simulink library "mbd_s32k1xx_ec_toolbox"  (Simulink 9.0)
settings: Solver=FixedStepDiscrete  StartTime=0.0  StopTime=10.0  FixedStep=0.1  RelTol=1e-3  EnableMultiTasking=on
InitFcn:
  | mbd_s32k_consistency_checks(bdroot(gcs));
(part 6 of 8)

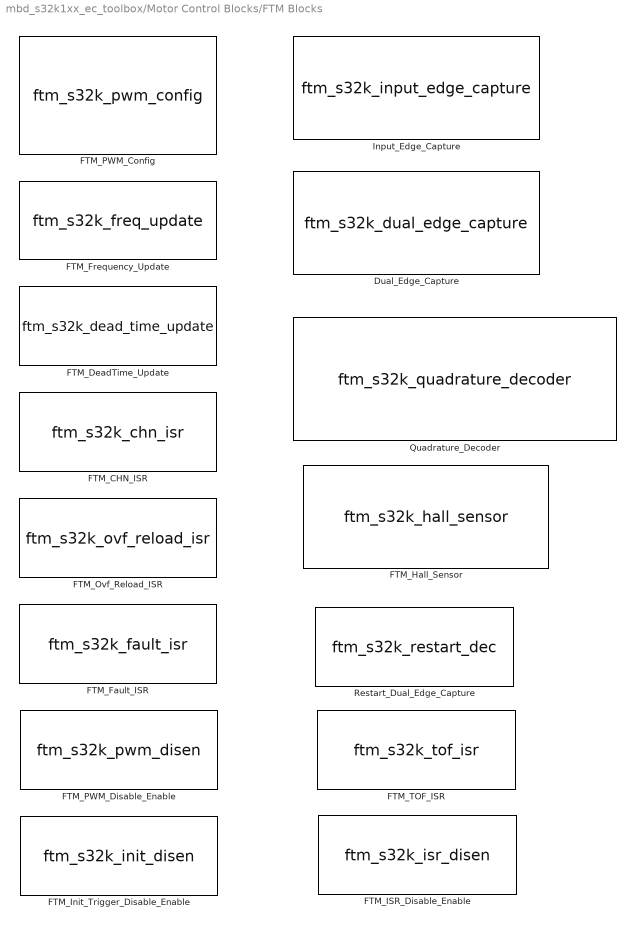
== system mbd_s32k1xx_ec_toolbox/Motor Control Blocks/FTM Blocks ==
  Dual_Edge_Capture : S-Function  FunctionName=ftm_s32k_dual_edge_capture  Parameters=funcParam  SFunctionDeploymentMode=off  EnableBusSupport=off  mask(FTM_s32k_dual_edge_capture_block){ftmModule=0, channel=0-1, c_mode=One-Shot, mesur=positive pulse (rising - falling), prescaler=1, filter_en=off, filter_value=0, isrlevel=15, pinFtmCh=PTD15: [FTM0_CH0 | FTM Channel]}
      mask prompts: ftmModule "Module"; channel "Channel pair"; c_mode "Capture mode"; mesur "Measurement"; prescaler "Prescale Factor"; filter_en "Filter enable"; filter_value "Input Filter value"; isrlevel "ISR priority"; pinFtmCh "FTM input pin"
      mask help: Dual Edge Capture block for signal pulse or period measurement on the even channel input.
      mask init:
      | mbd_s32k_ftm_display_modules(gcb);
      | mbd_s32k_ftm_edge_cbk(gcb, 'dual');
      | mbd_s32k_isr_priority_cbk(gcb, 'isrlevel');
      | 
      | [labels, maskStr] = mbd_s32k_ftm_dual_edge_init(gcb);
      | set_param(gcb, 'MaskDisplay', labels);
      | 
      | funcParam = [];
      settings: NameChangeFcn=mbd_s32k_name_check(gcb);
      mask Help: web(fullfile(mbd_s32k_block_help, 'ftm', 'dual_edge_capture_input.html'));
      mask TypeOptions ftmModule: 0 | 1 | 2 | 3 | 4 | 5 | 6 | 7
      mask Callback ftmModule:
      | mbd_s32k_ftm_display_modules(gcb);
      | mbd_s32k_ftm_edge_cbk(gcb, 'dual');
      mask TypeOptions channel: 0-1 | 2-3 | 4-5 | 6-7
      mask Callback channel: mbd_s32k_ftm_edge_cbk(gcb, 'dual');
      mask TypeOptions c_mode: One-Shot | Continuous
      mask TypeOptions mesur: positive pulse (rising - falling) | negative pulse (falling - rising) | period (rising - rising) | period (falling - falling)
      mask TypeOptions prescaler: 1 | 2 | 4 | 8 | 16 | 32 | 64 | 128
      mask Callback filter_en:
      | vis = get_param(gcb, 'MaskVisibilities');
      | 
      | %show/hide Filter value
      | idx = mbd_s32k_get_param_index(gcb, 'filter_value');
      | if strcmp(get_param(gcb,'filter_en'),'on')==1,
      |      vis{idx} = 'on';
      | elseif strcmp(get_param(gcb,'filter_en'),'off')==1,
      |     vis{idx} = 'off';
      | end
      | 
      | set_param(gcb,'MaskVisibilities',vis);
      | clear vis;
      mask TypeOptions isrlevel: 0 | 1 | 2 | 3 | 4 | 5 | 6 | 7 | 8 | 9 | 10 | 11 | 12 | 13 | 14 | 15
      mask TypeOptions pinFtmCh: PTD15: [FTM0_CH0 | FTM Channel] | PTB13: [FTM0_CH1 | FTM Channel] | PTC1: [FTM0_CH1 | FTM Channel] | PTD16: [FTM0_CH1 | FTM Channel] | PTC2: [FTM0_CH2 | FTM Channel] | PTD0: [FTM0_CH2 | FTM Channel] | PTC3: [FTM0_CH3 | FTM Channel] | PTD1: [FTM0_CH3 | FTM Channel] | PTB4: [FTM0_CH4 | FTM Channel] | PTB5: [FTM0_CH5 | FTM Channel] | PTE8: [FTM0_CH6 | FTM Channel] | PTE9: [FTM0_CH7 | FTM Channel] | PTB2: [FTM1_CH0 | FTM Channel] | PTC4: [FTM1_CH0 | FTM Channel] | PTA1: [FTM1_CH1 | FTM Channel] | PTB3: [FTM1_CH1 | FTM Channel] | PTC14: [FTM1_CH2 | FTM Channel] | PTC15: [FTM1_CH3 | FTM Channel] | PTA10: [FTM1_CH4 | FTM Channel] | PTA11: [FTM1_CH5 | FTM Channel] | PTA12: [FTM1_CH6 | FTM Channel] | PTA13: [FTM1_CH7 | FTM Channel] | PTC1: [FTM1_CH7 | FTM Channel] | PTD15: [FTM0_CH0 | FTM Channel] | PTB13: [FTM0_CH1 | FTM Channel] | PTC1: [FTM0_CH1 | FTM Channel] | PTD16: [FTM0_CH1 | FTM Channel] | PTC2: [FTM0_CH2 | FTM Channel] | PTD0: [FTM0_CH2 | FTM Channel] | PTC3: [FTM0_CH3 | FTM Channel] | PTD1: [FTM0_CH3 | FTM Channel] | PTB4: [FTM0_CH4 | FTM Channel] | PTB5: [FTM0_CH5 | FTM Channel] | PTE8: [FTM0_CH6 | FTM Channel] | PTE9: [FTM0_CH7 | FTM Channel] | PTB2: [FTM1_CH0 | FTM Channel] | PTC4: [FTM1_CH0 | FTM Channel] | PTA1: [FTM1_CH1 | FTM Channel] | PTB3: [FTM1_CH1 | FTM Channel] | PTC14: [FTM1_CH2 | FTM Channel] | PTC15: [FTM1_CH3 | FTM Channel] | PTA10: [FTM1_CH4 | FTM Channel] | PTA11: [FTM1_CH5 | FTM Channel] | PTA12: [FTM1_CH6 | FTM Channel] | PTA13: [FTM1_CH7 | FTM Channel] | PTC1: [FTM1_CH7 | FTM Channel] | PTD15: [FTM0_CH0 | FTM Channel] | PTB13: [FTM0_CH1 | FTM Channel] | PTC1: [FTM0_CH1 | FTM Channel] | PTD16: [FTM0_CH1 | FTM Channel] | PTC2: [FTM0_CH2 | FTM Channel] | PTD0: [FTM0_CH2 | FTM Channel] | PTC3: [FTM0_CH3 | FTM Channel] | PTD1: [FTM0_CH3 | FTM Channel] | PTB4: [FTM0_CH4 | FTM Channel] | PTB5: [FTM0_CH5 | FTM Channel] | PTE8: [FTM0_CH6 | FTM Channel] | PTE9: [FTM0_CH7 | FTM Channel] | PTB2: [FTM1_CH0 | FTM Channel] | PTC4: [FTM1_CH0 | FTM Channel] | PTA1: [FTM1_CH1 | FTM Channel] | PTB3: [FTM1_CH1 | FTM Channel] | PTC14: [FTM1_CH2 | FTM Channel] | PTC15: [FTM1_CH3 | FTM Channel] | PTA10: [FTM1_CH4 | FTM Channel] | PTA11: [FTM1_CH5 | FTM Channel] | PTA12: [FTM1_CH6 | FTM Channel] | PTA13: [FTM1_CH7 | FTM Channel] | PTC1: [FTM1_CH7 | FTM Channel] | PTC5: [FTM2_CH0 | FTM Channel] | PTD0: [FTM2_CH0 | FTM Channel] | PTD10: [FTM2_CH0 | FTM Channel] | PTA0: [FTM2_CH1 | FTM Channel] | PTD1: [FTM2_CH1 | FTM Channel] | PTD11: [FTM2_CH1 | FTM Channel] | PTD12: [FTM2_CH2 | FTM Channel] | PTE4: [FTM2_CH2 | FTM Channel] | PTD5: [FTM2_CH3 | FTM Channel] | PTE5: [FTM2_CH3 | FTM Channel] | PTD13: [FTM2_CH4 | FTM Channel] | PTE10: [FTM2_CH4 | FTM Channel] | PTD14: [FTM2_CH5 | FTM Channel] | PTE11: [FTM2_CH5 | FTM Channel] | PTC12: [FTM2_CH6 | FTM Channel] | PTE15: [FTM2_CH6 | FTM Channel] | PTC13: [FTM2_CH7 | FTM Channel] | PTE16: [FTM2_CH7 | FTM Channel] | PTA2: [FTM3_CH0 | FTM Channel] | PTB8: [FTM3_CH0 | FTM Channel] | PTA3: [FTM3_CH1 | FTM Channel] | PTB9: [FTM3_CH1 | FTM Channel] | PTB10: [FTM3_CH2 | FTM Channel] | PTC6: [FTM3_CH2 | FTM Channel] | PTB11: [FTM3_CH3 | FTM Channel] | PTC7: [FTM3_CH3 | FTM Channel] | PTC10: [FTM3_CH4 | FTM Channel] | PTD2: [FTM3_CH4 | FTM Channel] | PTC11: [FTM3_CH5 | FTM Channel] | PTD3: [FTM3_CH5 | FTM Channel] | PTC12: [FTM3_CH6 | FTM Channel] | PTE2: [FTM3_CH6 | FTM Channel] | PTC13: [FTM3_CH7 | FTM Channel] | PTE6: [FTM3_CH7 | FTM Channel] | PTD15: [FTM0_CH0 | FTM Channel] | PTB13: [FTM0_CH1 | FTM Channel] | PTC1: [FTM0_CH1 | FTM Channel] | PTD16: [FTM0_CH1 | FTM Channel] | PTC2: [FTM0_CH2 | FTM Channel] | PTD0: [FTM0_CH2 | FTM Channel] | PTC3: [FTM0_CH3 | FTM Channel] | PTD1: [FTM0_CH3 | FTM Channel] | PTB4: [FTM0_CH4 | FTM Channel] | PTB5: [FTM0_CH5 | FTM Channel] | PTE8: [FTM0_CH6 | FTM Channel] | PTE9: [FTM0_CH7 | FTM Channel] | PTB2: [FTM1_CH0 | FTM Channel] | PTC4: [FTM1_CH0 | FTM Channel] | PTA1: [FTM1_CH1 | FTM Channel] | PTB3: [FTM1_CH1 | FTM Channel] | PTC14: [FTM1_CH2 | FTM Channel] | PTC15: [FTM1_CH3 | FTM Channel] | PTA10: [FTM1_CH4 | FTM Channel] | PTA11: [FTM1_CH5 | FTM Channel] | PTA12: [FTM1_CH6 | FTM Channel] | PTA13: [FTM1_CH7 | FTM Channel] | PTC1: [FTM1_CH7 | FTM Channel] | PTC5: [FTM2_CH0 | FTM Channel] | PTD0: [FTM2_CH0 | FTM Channel] | PTD10: [FTM2_CH0 | FTM Channel] | PTA0: [FTM2_CH1 | FTM Channel] | PTD1: [FTM2_CH1 | FTM Channel] | PTD11: [FTM2_CH1 | FTM Channel] | PTD12: [FTM2_CH2 | FTM Channel] | PTE4: [FTM2_CH2 | FTM Channel] | PTD5: [FTM2_CH3 | FTM Channel] | PTE5: [FTM2_CH3 | FTM Channel] | PTD13: [FTM2_CH4 | FTM Channel] | PTE10: [FTM2_CH4 | FTM Channel] | PTD14: [FTM2_CH5 | FTM Channel] | PTE11: [FTM2_CH5 | FTM Channel] | PTC12: [FTM2_CH6 | FTM Channel] | PTE15: [FTM2_CH6 | FTM Channel] | PTC13: [FTM2_CH7 | FTM Channel] | PTE16: [FTM2_CH7 | FTM Channel] | PTA2: [FTM3_CH0 | FTM Channel] | PTB8: [FTM3_CH0 | FTM Channel] | PTA3: [FTM3_CH1 | FTM Channel] | PTB9: [FTM3_CH1 | FTM Channel] | PTB10: [FTM3_CH2 | FTM Channel] | PTC6: [FTM3_CH2 | FTM Channel] | PTB11: [FTM3_CH3 | FTM Channel] | PTC7: [FTM3_CH3 | FTM Channel] | PTC10: [FTM3_CH4 | FTM Channel] | PTD2: [FTM3_CH4 | FTM Channel] | PTC11: [FTM3_CH5 | FTM Channel] | PTD3: [FTM3_CH5 | FTM Channel] | PTC12: [FTM3_CH6 | FTM Channel] | PTE2: [FTM3_CH6 | FTM Channel] | PTC13: [FTM3_CH7 | FTM Channel] | PTE6: [FTM3_CH7 | FTM Channel] | PTD15: [FTM0_CH0 | FTM Channel] | PTB13: [FTM0_CH1 | FTM Channel] | PTC1: [FTM0_CH1 | FTM Channel] | PTD16: [FTM0_CH1 | FTM Channel] | PTC2: [FTM0_CH2 | FTM Channel] | PTD0: [FTM0_CH2 | FTM Channel] | PTC3: [FTM0_CH3 | FTM Channel] | PTD1: [FTM0_CH3 | FTM Channel] | PTB4: [FTM0_CH4 | FTM Channel] | PTB5: [FTM0_CH5 | FTM Channel] | PTE8: [FTM0_CH6 | FTM Channel] | PTE9: [FTM0_CH7 | FTM Channel] | PTB2: [FTM1_CH0 | FTM Channel] | PTC4: [FTM1_CH0 | FTM Channel] | PTA1: [FTM1_CH1 | FTM Channel] | PTB3: [FTM1_CH1 | FTM Channel] | PTC14: [FTM1_CH2 | FTM Channel] | PTC15: [FTM1_CH3 | FTM Channel] | PTA10: [FTM1_CH4 | FTM Channel] | PTA11: [FTM1_CH5 | FTM Channel] | PTA12: [FTM1_CH6 | FTM Channel] | PTA13: [FTM1_CH7 | FTM Channel] | PTC1: [FTM1_CH7 | FTM Channel] | PTC5: [FTM2_CH0 | FTM Channel] | PTD0: [FTM2_CH0 | FTM Channel] | PTD10: [FTM2_CH0 | FTM Channel] | PTA0: [FTM2_CH1 | FTM Channel] | PTD1: [FTM2_CH1 | FTM Channel] | PTD11: [FTM2_CH1 | FTM Channel] | PTD12: [FTM2_CH2 | FTM Channel] | PTE4: [FTM2_CH2 | FTM Channel] | PTD5: [FTM2_CH3 | FTM Channel] | PTE5: [FTM2_CH3 | FTM Channel] | PTD13: [FTM2_CH4 | FTM Channel] | PTE10: [FTM2_CH4 | FTM Channel] | PTD14: [FTM2_CH5 | FTM Channel] | PTE11: [FTM2_CH5 | FTM Channel] | PTC12: [FTM2_CH6 | FTM Channel] | PTE15: [FTM2_CH6 | FTM Channel] | PTC13: [FTM2_CH7 | FTM Channel] | PTE16: [FTM2_CH7 | FTM Channel] | PTA2: [FTM3_CH0 | FTM Channel] | PTB8: [FTM3_CH0 | FTM Channel] | PTA3: [FTM3_CH1 | FTM Channel] | PTB9: [FTM3_CH1 | FTM Channel] | PTB10: [FTM3_CH2 | FTM Channel] | PTC6: [FTM3_CH2 | FTM Channel] | PTB11: [FTM3_CH3 | FTM Channel] | PTC7: [FTM3_CH3 | FTM Channel] | PTC10: [FTM3_CH4 | FTM Channel] | PTD2: [FTM3_CH4 | FTM Channel] | PTC11: [FTM3_CH5 | FTM Channel] | PTD3: [FTM3_CH5 | FTM Channel] | PTC12: [FTM3_CH6 | FTM Channel] | PTE2: [FTM3_CH6 | FTM Channel] | PTC13: [FTM3_CH7 | FTM Channel] | PTE6: [FTM3_CH7 | FTM Channel] | PTE20: [FTM4_CH0 | FTM Channel] | PTE21: [FTM4_CH1 | FTM Channel] | PTC11: [FTM4_CH2 | FTM Channel] | PTE22: [FTM4_CH2 | FTM Channel] | PTE23: [FTM4_CH3 | FTM Channel] | PTC27: [FTM4_CH4 | FTM Channel] | PTE24: [FTM4_CH4 | FTM Channel] | PTB1: [FTM4_CH5 | FTM Channel] | PTE13: [FTM4_CH5 | FTM Channel] | PTE25: [FTM4_CH5 | FTM Channel] | PTB0: [FTM4_CH6 | FTM Channel] | PTC28: [FTM4_CH7 | FTM Channel] | PTA25: [FTM5_CH0 | FTM Channel] | PTC9: [FTM5_CH0 | FTM Channel] | PTA26: [FTM5_CH1 | FTM Channel] | PTC8: [FTM5_CH1 | FTM Channel] | PTA27: [FTM5_CH2 | FTM Channel] | PTC29: [FTM5_CH2 | FTM Channel] | PTA7: [FTM5_CH3 | FTM Channel] | PTA28: [FTM5_CH3 | FTM Channel] | PTA29: [FTM5_CH4 | FTM Channel] | PTC30: [FTM5_CH4 | FTM Channel] | PTA6: [FTM5_CH5 | FTM Channel] | PTA30: [FTM5_CH5 | FTM Channel] | PTA31: [FTM5_CH6 | FTM Channel] | PTC31: [FTM5_CH6 | FTM Channel] | PTB18: [FTM5_CH7 | FTM Channel] | PTD18: [FTM5_CH7 | FTM Channel] | PTD15: [FTM0_CH0 | FTM Channel] | PTB13: [FTM0_CH1 | FTM Channel] | PTC1: [FTM0_CH1 | FTM Channel] | PTD16: [FTM0_CH1 | FTM Channel] | PTC2: [FTM0_CH2 | FTM Channel] | PTD0: [FTM0_CH2 | FTM Channel] | PTC3: [FTM0_CH3 | FTM Channel] | PTD1: [FTM0_CH3 | FTM Channel] | PTB4: [FTM0_CH4 | FTM Channel] | PTB5: [FTM0_CH5 | FTM Channel] | PTE8: [FTM0_CH6 | FTM Channel] | PTE9: [FTM0_CH7 | FTM Channel] | PTB2: [FTM1_CH0 | FTM Channel] | PTC4: [FTM1_CH0 | FTM Channel] | PTA1: [FTM1_CH1 | FTM Channel] | PTB3: [FTM1_CH1 | FTM Channel] | PTC14: [FTM1_CH2 | FTM Channel] | PTC15: [FTM1_CH3 | FTM Channel] | PTA10: [FTM1_CH4 | FTM Channel] | PTA11: [FTM1_CH5 | FTM Channel] | PTA12: [FTM1_CH6 | FTM Channel] | PTA13: [FTM1_CH7 | FTM Channel] | PTC1: [FTM1_CH7 | FTM Channel] | PTC5: [FTM2_CH0 | FTM Channel] | PTD0: [FTM2_CH0 | FTM Channel] | PTD10: [FTM2_CH0 | FTM Channel] | PTA0: [FTM2_CH1 | FTM Channel] | PTD1: [FTM2_CH1 | FTM Channel] | PTD11: [FTM2_CH1 | FTM Channel] | PTD12: [FTM2_CH2 | FTM Channel] | PTE4: [FTM2_CH2 | FTM Channel] | PTD5: [FTM2_CH3 | FTM Channel] | PTE5: [FTM2_CH3 | FTM Channel] | PTD13: [FTM2_CH4 | FTM Channel] | PTE10: [FTM2_CH4 | FTM Channel] | PTD14: [FTM2_CH5 | FTM Channel] | PTE11: [FTM2_CH5 | FTM Channel] | PTC12: [FTM2_CH6 | FTM Channel] | PTE15: [FTM2_CH6 | FTM Channel] | PTC13: [FTM2_CH7 | FTM Channel] | PTE16: [FTM2_CH7 | FTM Channel] | PTA2: [FTM3_CH0 | FTM Channel] | PTB8: [FTM3_CH0 | FTM Channel] | PTA3: [FTM3_CH1 | FTM Channel] | PTB9: [FTM3_CH1 | FTM Channel] | PTB10: [FTM3_CH2 | FTM Channel] | PTC6: [FTM3_CH2 | FTM Channel] | PTB11: [FTM3_CH3 | FTM Channel] | PTC7: [FTM3_CH3 | FTM Channel] | PTC10: [FTM3_CH4 | FTM Channel] | PTD2: [FTM3_CH4 | FTM Channel] | PTC11: [FTM3_CH5 | FTM Channel] | PTD3: [FTM3_CH5 | FTM Channel] | PTC12: [FTM3_CH6 | FTM Channel] | PTE2: [FTM3_CH6 | FTM Channel] | PTC13: [FTM3_CH7 | FTM Channel] | PTE6: [FTM3_CH7 | FTM Channel] | PTE20: [FTM4_CH0 | FTM Channel] | PTE21: [FTM4_CH1 | FTM Channel] | PTC11: [FTM4_CH2 | FTM Channel] | PTE22: [FTM4_CH2 | FTM Channel] | PTE23: [FTM4_CH3 | FTM Channel] | PTC27: [FTM4_CH4 | FTM Channel] | PTE24: [FTM4_CH4 | FTM Channel] | PTB1: [FTM4_CH5 | FTM Channel] | PTE13: [FTM4_CH5 | FTM Channel] | PTE25: [FTM4_CH5 | FTM Channel] | PTB0: [FTM4_CH6 | FTM Channel] | PTC28: [FTM4_CH7 | FTM Channel] | PTA25: [FTM5_CH0 | FTM Channel] | PTC9: [FTM5_CH0 | FTM Channel] | PTA26: [FTM5_CH1 | FTM Channel] | PTC8: [FTM5_CH1 | FTM Channel] | PTA27: [FTM5_CH2 | FTM Channel] | PTC29: [FTM5_CH2 | FTM Channel] | PTA7: [FTM5_CH3 | FTM Channel] | PTA28: [FTM5_CH3 | FTM Channel] | PTA29: [FTM5_CH4 | FTM Channel] | PTC30: [FTM5_CH4 | FTM Channel] | PTA6: [FTM5_CH5 | FTM Channel] | PTA30: [FTM5_CH5 | FTM Channel] | PTA31: [FTM5_CH6 | FTM Channel] | PTC31: [FTM5_CH6 | FTM Channel] | PTB18: [FTM5_CH7 | FTM Channel] | PTD18: [FTM5_CH7 | FTM Channel] | PTA18: [FTM6_CH0 | FTM Channel] | PTB20: [FTM6_CH0 | FTM Channel] | PTD19: [FTM6_CH0 | FTM Channel] | PTB21: [FTM6_CH1 | FTM Channel] | PTD20: [FTM6_CH1 | FTM Channel] | PTB22: [FTM6_CH2 | FTM Channel] | PTD21: [FTM6_CH2 | FTM Channel] | PTB23: [FTM6_CH3 | FTM Channel] | PTD22: [FTM6_CH3 | FTM Channel] | PTB24: [FTM6_CH4 | FTM Channel] | PTD23: [FTM6_CH4 | FTM Channel] | PTB25: [FTM6_CH5 | FTM Channel] | PTD24: [FTM6_CH5 | FTM Channel] | PTB26: [FTM6_CH6 | FTM Channel] | PTD25: [FTM6_CH6 | FTM Channel] | PTB27: [FTM6_CH7 | FTM Channel] | PTD26: [FTM6_CH7 | FTM Channel] | PTB28: [FTM7_CH0 | FTM Channel] | PTD27: [FTM7_CH0 | FTM Channel] | PTB29: [FTM7_CH1 | FTM Channel] | PTD28: [FTM7_CH1 | FTM Channel] | PTB30: [FTM7_CH2 | FTM Channel] | PTD29: [FTM7_CH2 | FTM Channel] | PTB31: [FTM7_CH3 | FTM Channel] | PTD30: [FTM7_CH3 | FTM Channel] | PTC18: [FTM7_CH4 | FTM Channel] | PTD31: [FTM7_CH4 | FTM Channel] | PTC19: [FTM7_CH5 | FTM Channel] | PTE17: [FTM7_CH5 | FTM Channel] | PTC20: [FTM7_CH6 | FTM Channel] | PTE18: [FTM7_CH6 | FTM Channel] | PTC21: [FTM7_CH7 | FTM Channel] | PTE19: [FTM7_CH7 | FTM Channel]
      mask Display:
      | image('nxp_logo.png', 'top-right');
      | port_label('output',1,'Trigger');
      | port_label('output',2,'Measured Time');
      | disp(maskStr);
  FTM_CHN_ISR : S-Function  Priority=10  FunctionName=ftm_s32k_chn_isr  Parameters=ftmModule,channel,isrlevel  SFunctionDeploymentMode=off  EnableBusSupport=off  mask(FTM_s32k_chn_isr_block){ftmModule=0, channel=0, isrlevel=15, mcuTargetUpdate=on}
      mask prompts: ftmModule "Module"; isrlevel "ISR priority"; mcuTargetUpdate "Mcu target update"
      mask help: FTM Channel interrupt handler
      mask init:
      | mbd_s32k_ftm_display_modules(gcb);
      | mbd_s32k_isr_priority_cbk(gcb, 'isrlevel');
      | 
      | maskStr = [ 'FTM PWM Channel ISR', newline, newline, ...
      |             'Module : ', get_param(gcb,'ftmModule'), newline, ...
      |             'Channel: ', get_param(gcb, 'channel'), newline, ...
      |             'Interrupt Priority: ', get_param(gcb, 'isrlevel')];
      settings: NameChangeFcn=mbd_s32k_name_check(gcb);
      mask Help: web(fullfile(mbd_s32k_block_help, 'ftm', 'ftm_chn_isr_block.html'));
      mask TypeOptions ftmModule: 0 | 1 | 2 | 3 | 4 | 5 | 6 | 7
      mask TypeOptions channel: 0 | 1 | 2 | 3 | 4 | 5 | 6 | 7
      mask TypeOptions isrlevel: 0 | 1 | 2 | 3 | 4 | 5 | 6 | 7 | 8 | 9 | 10 | 11 | 12 | 13 | 14 | 15
      mask Display:
      | image('nxp_logo.png', 'top-right');
      | disp(maskStr);
      | port_label('output',1,'function');
  FTM_DeadTime_Update : S-Function  Priority=1  FunctionName=ftm_s32k_dead_time_update  Parameters=funcParams  SFunctionDeploymentMode=off  EnableBusSupport=off  mask(FTM_s32k_dead_time_update_block){ftmModule=0, mcuTargetUpdate=on, deadtimeUnits=Nanoseconds, deadtimePrescaler=Divide by 1}
      mask prompts: ftmModule "Module"; mcuTargetUpdate "Mcu target update"; deadtimeUnits "Deadtime expressed in units of:"; deadtimePrescaler "Deadtime prescaler"
      mask help: FTM DeadTime update for PWM output block.
      mask init:
      | mbd_s32k_ftm_display_modules(gcb);
      | 
      | [labels, maskStr] = mbd_s32k_ftm_pwm_deadtime_update_init(gcb);
      | 
      | funcParams = [0 10 1];
      | set_param(gcb, 'MaskDisplay', labels);
      settings: NameChangeFcn=mbd_s32k_name_check(gcb);
      mask Help: web(fullfile(mbd_s32k_block_help, 'ftm', 'ftm_dead_time_update_block.html'));
      mask TypeOptions ftmModule: 0 | 1 | 2 | 3 | 4 | 5 | 6 | 7
      mask TypeOptions deadtimeUnits: Ticks | Nanoseconds
      mask Callback deadtimeUnits: mbd_s32k_ftm_pwm_deadtime_update_cbk(gcb, 'ftm_show_deadtime');
      mask TypeOptions deadtimePrescaler: Divide by 1 | Divide by 4 | Divide by 16
      mask DialogControl ParameterTabVar0 Prompt: General
      mask Display:
      | image('nxp_logo.png', 'top-right');
      | port_label('input',1,'DeadTime')
      | disp(maskStr);
  FTM_Fault_ISR : S-Function  Priority=10  FunctionName=ftm_s32k_fault_isr  Parameters=sFuncParams  SFunctionDeploymentMode=off  EnableBusSupport=off  mask(FTM_s32k_fault_isr){ftmModule=0, faultChannel=1, isrPriority=15, mcuTargetUpdate=on}
      mask prompts: ftmModule "Module"; faultChannel "Channel"; isrPriority "ISR priority"; mcuTargetUpdate "Mcu target update"
      mask help: FTM Channel Fault Interrupt Handler
      mask init:
      | mbd_s32k_ftm_display_modules(gcb);
      | sFuncParams = [];
      | maskStr = [ 'FTM PWM Fault ISR', newline, newline, ...
      |             'Module : ', get_param(gcb,'ftmModule'), newline, ...
      |             'Fault channel: ', get_param(gcb,'faultChannel')];
      settings: NameChangeFcn=mbd_s32k_name_check(gcb);
      mask Help: web(fullfile(mbd_s32k_block_help, 'ftm', 'ftm_fault_isr_block.html'));
      mask TypeOptions ftmModule: 0 | 1 | 2 | 3 | 4 | 5 | 6 | 7
      mask Callback ftmModule:
      | mbd_s32k_ftm_display_modules(gcb);
      | mbd_s32k_ftm_pwm_fault_cbk(gcb, 'ftm_update_fault_channel');
      mask TypeOptions faultChannel: 0 | 1 | 2 | 3
      mask TypeOptions isrPriority: 0 | 1 | 2 | 3 | 4 | 5 | 6 | 7 | 8 | 9 | 10 | 11 | 12 | 13 | 14 | 15
      mask Display:
      | image('nxp_logo.png', 'top-right');
      | disp(maskStr);
      | port_label('output',1,'function');
  FTM_Frequency_Update : S-Function  Priority=1  FunctionName=ftm_s32k_freq_update  Parameters=funcParams  SFunctionDeploymentMode=off  EnableBusSupport=off  mask(FTM_s32k_freq_update_block){ftmModule=0, mcuTargetUpdate=on, ftmPwmUnits=Hz}
      mask prompts: ftmModule "Module"; mcuTargetUpdate "Mcu target update"; ftmPwmUnits "PWM Period expressed in units of:"
      mask help: FTM PWM output frequency update.
      mask init:
      | mbd_s32k_ftm_display_modules(gcb);
      | 
      | funcParams = [0];
      | 
      | [labels, maskStr] = mbd_s32k_ftm_pwm_frequency_update_init(gcb);
      | 
      | funcParams = [0 10 1];
      | set_param(gcb, 'MaskDisplay', labels);
      settings: NameChangeFcn=mbd_s32k_name_check(gcb);
      mask Help: web(fullfile(mbd_s32k_block_help, 'ftm', 'ftm_freq_update_block.html'));
      mask TypeOptions ftmModule: 0 | 1 | 2 | 3 | 4 | 5 | 6 | 7
      mask TypeOptions ftmPwmUnits: Ticks | Hz
      mask DialogControl ParameterTabVar0 Prompt: General
      mask Display:
      | image('nxp_logo.png', 'top-right');
      | port_label('input',1,'Frequency')
      | disp(maskStr);
  FTM_Hall_Sensor : S-Function  Priority=1  FunctionName=ftm_s32k_hall_sensor  Parameters=funcParam  SFunctionDeploymentMode=off  EnableBusSupport=off  mask(FTM_s32k_hall_sensor_block){e_mode=Rising or Falling, prescaler=1, max_period=0.00081919, isrlevel=15, mcuTargetUpdate=on, filter_en=off, filter_value=0, pinFtm1Ch1=PTA1: [FTM1_CH1 | FTM Channel], pinFtm2Ch0=PTD10: [FTM2_CH0 | FTM Channel], pinFtm2Ch1=PTD11: [FTM2_CH1 | FTM Channel]}
      mask prompts: e_mode "Edge-sensitive mode"; prescaler "Prescale Factor"; max_period "Max period (s)"; isrlevel "ISR priority"; filter_en "Filter enable"; filter_value "Input Filter value"; pinFtm1Ch1 "FTM1 Channel 1 input pin"; pinFtm2Ch0 "FTM2 Channel 0 input pin"; pinFtm2Ch1 "FTM2 Channel 1 input pin"
      mask help: To simplify the speed calculation required by the CPU on each hall sensor's input, all 3 inputs are "exclusively OR'd" into one timer channel and the free running counter is refreshed on every edge. The counter value is returned as block output value.
      mask init:
      | mbd_s32k_ftm_hall_sensor_cbk(gcb);
      | 
      | [labels, maskStr] = mbd_s32k_ftm_hall_sensor_init(gcb);
      | set_param(gcb, 'MaskDisplay', labels);
      | 
      | funcParam = [];
      settings: NameChangeFcn=mbd_s32k_name_check(gcb);
      mask Help: web(fullfile(mbd_s32k_block_help, 'ftm', 'hall_sensor.html'));
      mask TypeOptions e_mode: Rising | Falling | Rising or Falling
      mask Callback e_mode: mbd_s32k_ftm_hall_sensor_cbk(gcb)
      mask TypeOptions prescaler: 1 | 2 | 4 | 8 | 16 | 32 | 64 | 128
      mask Callback prescaler:
      | prescale = str2double(get_param(gcb, 'prescaler'));
      | clockFreq = mbd_s32k_get_system_clock();
      | max_period = ((2^16-1) * prescale) / clockFreq;
      | set_param(gcb, 'max_period',num2str(max_period));
      mask TypeOptions isrlevel: 0 | 1 | 2 | 3 | 4 | 5 | 6 | 7 | 8 | 9 | 10 | 11 | 12 | 13 | 14 | 15
      mask Callback filter_en:
      | vis = get_param(gcb, 'MaskVisibilities');
      | 
      | %show/hide Filter value
      | idx = mbd_s32k_get_param_index(gcb, 'filter_value');
      | if strcmp(get_param(gcb,'filter_en'),'on')==1,
      |      vis{idx} = 'on';
      | elseif strcmp(get_param(gcb,'filter_en'),'off')==1,
      |     vis{idx} = 'off';
      | end
      | 
      | set_param(gcb,'MaskVisibilities',vis);
      mask TypeOptions pinFtm1Ch1: PTD15: [FTM0_CH0 | FTM Channel] | PTB13: [FTM0_CH1 | FTM Channel] | PTC1: [FTM0_CH1 | FTM Channel] | PTD16: [FTM0_CH1 | FTM Channel] | PTC2: [FTM0_CH2 | FTM Channel] | PTD0: [FTM0_CH2 | FTM Channel] | PTC3: [FTM0_CH3 | FTM Channel] | PTD1: [FTM0_CH3 | FTM Channel] | PTB4: [FTM0_CH4 | FTM Channel] | PTB5: [FTM0_CH5 | FTM Channel] | PTE8: [FTM0_CH6 | FTM Channel] | PTE9: [FTM0_CH7 | FTM Channel] | PTB2: [FTM1_CH0 | FTM Channel] | PTC4: [FTM1_CH0 | FTM Channel] | PTA1: [FTM1_CH1 | FTM Channel] | PTB3: [FTM1_CH1 | FTM Channel] | PTC14: [FTM1_CH2 | FTM Channel] | PTC15: [FTM1_CH3 | FTM Channel] | PTA10: [FTM1_CH4 | FTM Channel] | PTA11: [FTM1_CH5 | FTM Channel] | PTA12: [FTM1_CH6 | FTM Channel] | PTA13: [FTM1_CH7 | FTM Channel] | PTC1: [FTM1_CH7 | FTM Channel] | PTD15: [FTM0_CH0 | FTM Channel] | PTB13: [FTM0_CH1 | FTM Channel] | PTC1: [FTM0_CH1 | FTM Channel] | PTD16: [FTM0_CH1 | FTM Channel] | PTC2: [FTM0_CH2 | FTM Channel] | PTD0: [FTM0_CH2 | FTM Channel] | PTC3: [FTM0_CH3 | FTM Channel] | PTD1: [FTM0_CH3 | FTM Channel] | PTB4: [FTM0_CH4 | FTM Channel] | PTB5: [FTM0_CH5 | FTM Channel] | PTE8: [FTM0_CH6 | FTM Channel] | PTE9: [FTM0_CH7 | FTM Channel] | PTB2: [FTM1_CH0 | FTM Channel] | PTC4: [FTM1_CH0 | FTM Channel] | PTA1: [FTM1_CH1 | FTM Channel] | PTB3: [FTM1_CH1 | FTM Channel] | PTC14: [FTM1_CH2 | FTM Channel] | PTC15: [FTM1_CH3 | FTM Channel] | PTA10: [FTM1_CH4 | FTM Channel] | PTA11: [FTM1_CH5 | FTM Channel] | PTA12: [FTM1_CH6 | FTM Channel] | PTA13: [FTM1_CH7 | FTM Channel] | PTC1: [FTM1_CH7 | FTM Channel] | PTD15: [FTM0_CH0 | FTM Channel] | PTB13: [FTM0_CH1 | FTM Channel] | PTC1: [FTM0_CH1 | FTM Channel] | PTD16: [FTM0_CH1 | FTM Channel] | PTC2: [FTM0_CH2 | FTM Channel] | PTD0: [FTM0_CH2 | FTM Channel] | PTC3: [FTM0_CH3 | FTM Channel] | PTD1: [FTM0_CH3 | FTM Channel] | PTB4: [FTM0_CH4 | FTM Channel] | PTB5: [FTM0_CH5 | FTM Channel] | PTE8: [FTM0_CH6 | FTM Channel] | PTE9: [FTM0_CH7 | FTM Channel] | PTB2: [FTM1_CH0 | FTM Channel] | PTC4: [FTM1_CH0 | FTM Channel] | PTA1: [FTM1_CH1 | FTM Channel] | PTB3: [FTM1_CH1 | FTM Channel] | PTC14: [FTM1_CH2 | FTM Channel] | PTC15: [FTM1_CH3 | FTM Channel] | PTA10: [FTM1_CH4 | FTM Channel] | PTA11: [FTM1_CH5 | FTM Channel] | PTA12: [FTM1_CH6 | FTM Channel] | PTA13: [FTM1_CH7 | FTM Channel] | PTC1: [FTM1_CH7 | FTM Channel] | PTC5: [FTM2_CH0 | FTM Channel] | PTD0: [FTM2_CH0 | FTM Channel] | PTD10: [FTM2_CH0 | FTM Channel] | PTA0: [FTM2_CH1 | FTM Channel] | PTD1: [FTM2_CH1 | FTM Channel] | PTD11: [FTM2_CH1 | FTM Channel] | PTD12: [FTM2_CH2 | FTM Channel] | PTE4: [FTM2_CH2 | FTM Channel] | PTD5: [FTM2_CH3 | FTM Channel] | PTE5: [FTM2_CH3 | FTM Channel] | PTD13: [FTM2_CH4 | FTM Channel] | PTE10: [FTM2_CH4 | FTM Channel] | PTD14: [FTM2_CH5 | FTM Channel] | PTE11: [FTM2_CH5 | FTM Channel] | PTC12: [FTM2_CH6 | FTM Channel] | PTE15: [FTM2_CH6 | FTM Channel] | PTC13: [FTM2_CH7 | FTM Channel] | PTE16: [FTM2_CH7 | FTM Channel] | PTA2: [FTM3_CH0 | FTM Channel] | PTB8: [FTM3_CH0 | FTM Channel] | PTA3: [FTM3_CH1 | FTM Channel] | PTB9: [FTM3_CH1 | FTM Channel] | PTB10: [FTM3_CH2 | FTM Channel] | PTC6: [FTM3_CH2 | FTM Channel] | PTB11: [FTM3_CH3 | FTM Channel] | PTC7: [FTM3_CH3 | FTM Channel] | PTC10: [FTM3_CH4 | FTM Channel] | PTD2: [FTM3_CH4 | FTM Channel] | PTC11: [FTM3_CH5 | FTM Channel] | PTD3: [FTM3_CH5 | FTM Channel] | PTC12: [FTM3_CH6 | FTM Channel] | PTE2: [FTM3_CH6 | FTM Channel] | PTC13: [FTM3_CH7 | FTM Channel] | PTE6: [FTM3_CH7 | FTM Channel] | PTD15: [FTM0_CH0 | FTM Channel] | PTB13: [FTM0_CH1 | FTM Channel] | PTC1: [FTM0_CH1 | FTM Channel] | PTD16: [FTM0_CH1 | FTM Channel] | PTC2: [FTM0_CH2 | FTM Channel] | PTD0: [FTM0_CH2 | FTM Channel] | PTC3: [FTM0_CH3 | FTM Channel] | PTD1: [FTM0_CH3 | FTM Channel] | PTB4: [FTM0_CH4 | FTM Channel] | PTB5: [FTM0_CH5 | FTM Channel] | PTE8: [FTM0_CH6 | FTM Channel] | PTE9: [FTM0_CH7 | FTM Channel] | PTB2: [FTM1_CH0 | FTM Channel] | PTC4: [FTM1_CH0 | FTM Channel] | PTA1: [FTM1_CH1 | FTM Channel] | PTB3: [FTM1_CH1 | FTM Channel] | PTC14: [FTM1_CH2 | FTM Channel] | PTC15: [FTM1_CH3 | FTM Channel] | PTA10: [FTM1_CH4 | FTM Channel] | PTA11: [FTM1_CH5 | FTM Channel] | PTA12: [FTM1_CH6 | FTM Channel] | PTA13: [FTM1_CH7 | FTM Channel] | PTC1: [FTM1_CH7 | FTM Channel] | PTC5: [FTM2_CH0 | FTM Channel] | PTD0: [FTM2_CH0 | FTM Channel] | PTD10: [FTM2_CH0 | FTM Channel] | PTA0: [FTM2_CH1 | FTM Channel] | PTD1: [FTM2_CH1 | FTM Channel] | PTD11: [FTM2_CH1 | FTM Channel] | PTD12: [FTM2_CH2 | FTM Channel] | PTE4: [FTM2_CH2 | FTM Channel] | PTD5: [FTM2_CH3 | FTM Channel] | PTE5: [FTM2_CH3 | FTM Channel] | PTD13: [FTM2_CH4 | FTM Channel] | PTE10: [FTM2_CH4 | FTM Channel] | PTD14: [FTM2_CH5 | FTM Channel] | PTE11: [FTM2_CH5 | FTM Channel] | PTC12: [FTM2_CH6 | FTM Channel] | PTE15: [FTM2_CH6 | FTM Channel] | PTC13: [FTM2_CH7 | FTM Channel] | PTE16: [FTM2_CH7 | FTM Channel] | PTA2: [FTM3_CH0 | FTM Channel] | PTB8: [FTM3_CH0 | FTM Channel] | PTA3: [FTM3_CH1 | FTM Channel] | PTB9: [FTM3_CH1 | FTM Channel] | PTB10: [FTM3_CH2 | FTM Channel] | PTC6: [FTM3_CH2 | FTM Channel] | PTB11: [FTM3_CH3 | FTM Channel] | PTC7: [FTM3_CH3 | FTM Channel] | PTC10: [FTM3_CH4 | FTM Channel] | PTD2: [FTM3_CH4 | FTM Channel] | PTC11: [FTM3_CH5 | FTM Channel] | PTD3: [FTM3_CH5 | FTM Channel] | PTC12: [FTM3_CH6 | FTM Channel] | PTE2: [FTM3_CH6 | FTM Channel] | PTC13: [FTM3_CH7 | FTM Channel] | PTE6: [FTM3_CH7 | FTM Channel] | PTD15: [FTM0_CH0 | FTM Channel] | PTB13: [FTM0_CH1 | FTM Channel] | PTC1: [FTM0_CH1 | FTM Channel] | PTD16: [FTM0_CH1 | FTM Channel] | PTC2: [FTM0_CH2 | FTM Channel] | PTD0: [FTM0_CH2 | FTM Channel] | PTC3: [FTM0_CH3 | FTM Channel] | PTD1: [FTM0_CH3 | FTM Channel] | PTB4: [FTM0_CH4 | FTM Channel] | PTB5: [FTM0_CH5 | FTM Channel] | PTE8: [FTM0_CH6 | FTM Channel] | PTE9: [FTM0_CH7 | FTM Channel] | PTB2: [FTM1_CH0 | FTM Channel] | PTC4: [FTM1_CH0 | FTM Channel] | PTA1: [FTM1_CH1 | FTM Channel] | PTB3: [FTM1_CH1 | FTM Channel] | PTC14: [FTM1_CH2 | FTM Channel] | PTC15: [FTM1_CH3 | FTM Channel] | PTA10: [FTM1_CH4 | FTM Channel] | PTA11: [FTM1_CH5 | FTM Channel] | PTA12: [FTM1_CH6 | FTM Channel] | PTA13: [FTM1_CH7 | FTM Channel] | PTC1: [FTM1_CH7 | FTM Channel] | PTC5: [FTM2_CH0 | FTM Channel] | PTD0: [FTM2_CH0 | FTM Channel] | PTD10: [FTM2_CH0 | FTM Channel] | PTA0: [FTM2_CH1 | FTM Channel] | PTD1: [FTM2_CH1 | FTM Channel] | PTD11: [FTM2_CH1 | FTM Channel] | PTD12: [FTM2_CH2 | FTM Channel] | PTE4: [FTM2_CH2 | FTM Channel] | PTD5: [FTM2_CH3 | FTM Channel] | PTE5: [FTM2_CH3 | FTM Channel] | PTD13: [FTM2_CH4 | FTM Channel] | PTE10: [FTM2_CH4 | FTM Channel] | PTD14: [FTM2_CH5 | FTM Channel] | PTE11: [FTM2_CH5 | FTM Channel] | PTC12: [FTM2_CH6 | FTM Channel] | PTE15: [FTM2_CH6 | FTM Channel] | PTC13: [FTM2_CH7 | FTM Channel] | PTE16: [FTM2_CH7 | FTM Channel] | PTA2: [FTM3_CH0 | FTM Channel] | PTB8: [FTM3_CH0 | FTM Channel] | PTA3: [FTM3_CH1 | FTM Channel] | PTB9: [FTM3_CH1 | FTM Channel] | PTB10: [FTM3_CH2 | FTM Channel] | PTC6: [FTM3_CH2 | FTM Channel] | PTB11: [FTM3_CH3 | FTM Channel] | PTC7: [FTM3_CH3 | FTM Channel] | PTC10: [FTM3_CH4 | FTM Channel] | PTD2: [FTM3_CH4 | FTM Channel] | PTC11: [FTM3_CH5 | FTM Channel] | PTD3: [FTM3_CH5 | FTM Channel] | PTC12: [FTM3_CH6 | FTM Channel] | PTE2: [FTM3_CH6 | FTM Channel] | PTC13: [FTM3_CH7 | FTM Channel] | PTE6: [FTM3_CH7 | FTM Channel] | PTE20: [FTM4_CH0 | FTM Channel] | PTE21: [FTM4_CH1 | FTM Channel] | PTC11: [FTM4_CH2 | FTM Channel] | PTE22: [FTM4_CH2 | FTM Channel] | PTE23: [FTM4_CH3 | FTM Channel] | PTC27: [FTM4_CH4 | FTM Channel] | PTE24: [FTM4_CH4 | FTM Channel] | PTB1: [FTM4_CH5 | FTM Channel] | PTE13: [FTM4_CH5 | FTM Channel] | PTE25: [FTM4_CH5 | FTM Channel] | PTB0: [FTM4_CH6 | FTM Channel] | PTC28: [FTM4_CH7 | FTM Channel] | PTA25: [FTM5_CH0 | FTM Channel] | PTC9: [FTM5_CH0 | FTM Channel] | PTA26: [FTM5_CH1 | FTM Channel] | PTC8: [FTM5_CH1 | FTM Channel] | PTA27: [FTM5_CH2 | FTM Channel] | PTC29: [FTM5_CH2 | FTM Channel] | PTA7: [FTM5_CH3 | FTM Channel] | PTA28: [FTM5_CH3 | FTM Channel] | PTA29: [FTM5_CH4 | FTM Channel] | PTC30: [FTM5_CH4 | FTM Channel] | PTA6: [FTM5_CH5 | FTM Channel] | PTA30: [FTM5_CH5 | FTM Channel] | PTA31: [FTM5_CH6 | FTM Channel] | PTC31: [FTM5_CH6 | FTM Channel] | PTB18: [FTM5_CH7 | FTM Channel] | PTD18: [FTM5_CH7 | FTM Channel] | PTD15: [FTM0_CH0 | FTM Channel] | PTB13: [FTM0_CH1 | FTM Channel] | PTC1: [FTM0_CH1 | FTM Channel] | PTD16: [FTM0_CH1 | FTM Channel] | PTC2: [FTM0_CH2 | FTM Channel] | PTD0: [FTM0_CH2 | FTM Channel] | PTC3: [FTM0_CH3 | FTM Channel] | PTD1: [FTM0_CH3 | FTM Channel] | PTB4: [FTM0_CH4 | FTM Channel] | PTB5: [FTM0_CH5 | FTM Channel] | PTE8: [FTM0_CH6 | FTM Channel] | PTE9: [FTM0_CH7 | FTM Channel] | PTB2: [FTM1_CH0 | FTM Channel] | PTC4: [FTM1_CH0 | FTM Channel] | PTA1: [FTM1_CH1 | FTM Channel] | PTB3: [FTM1_CH1 | FTM Channel] | PTC14: [FTM1_CH2 | FTM Channel] | PTC15: [FTM1_CH3 | FTM Channel] | PTA10: [FTM1_CH4 | FTM Channel] | PTA11: [FTM1_CH5 | FTM Channel] | PTA12: [FTM1_CH6 | FTM Channel] | PTA13: [FTM1_CH7 | FTM Channel] | PTC1: [FTM1_CH7 | FTM Channel] | PTC5: [FTM2_CH0 | FTM Channel] | PTD0: [FTM2_CH0 | FTM Channel] | PTD10: [FTM2_CH0 | FTM Channel] | PTA0: [FTM2_CH1 | FTM Channel] | PTD1: [FTM2_CH1 | FTM Channel] | PTD11: [FTM2_CH1 | FTM Channel] | PTD12: [FTM2_CH2 | FTM Channel] | PTE4: [FTM2_CH2 | FTM Channel] | PTD5: [FTM2_CH3 | FTM Channel] | PTE5: [FTM2_CH3 | FTM Channel] | PTD13: [FTM2_CH4 | FTM Channel] | PTE10: [FTM2_CH4 | FTM Channel] | PTD14: [FTM2_CH5 | FTM Channel] | PTE11: [FTM2_CH5 | FTM Channel] | PTC12: [FTM2_CH6 | FTM Channel] | PTE15: [FTM2_CH6 | FTM Channel] | PTC13: [FTM2_CH7 | FTM Channel] | PTE16: [FTM2_CH7 | FTM Channel] | PTA2: [FTM3_CH0 | FTM Channel] | PTB8: [FTM3_CH0 | FTM Channel] | PTA3: [FTM3_CH1 | FTM Channel] | PTB9: [FTM3_CH1 | FTM Channel] | PTB10: [FTM3_CH2 | FTM Channel] | PTC6: [FTM3_CH2 | FTM Channel] | PTB11: [FTM3_CH3 | FTM Channel] | PTC7: [FTM3_CH3 | FTM Channel] | PTC10: [FTM3_CH4 | FTM Channel] | PTD2: [FTM3_CH4 | FTM Channel] | PTC11: [FTM3_CH5 | FTM Channel] | PTD3: [FTM3_CH5 | FTM Channel] | PTC12: [FTM3_CH6 | FTM Channel] | PTE2: [FTM3_CH6 | FTM Channel] | PTC13: [FTM3_CH7 | FTM Channel] | PTE6: [FTM3_CH7 | FTM Channel] | PTE20: [FTM4_CH0 | FTM Channel] | PTE21: [FTM4_CH1 | FTM Channel] | PTC11: [FTM4_CH2 | FTM Channel] | PTE22: [FTM4_CH2 | FTM Channel] | PTE23: [FTM4_CH3 | FTM Channel] | PTC27: [FTM4_CH4 | FTM Channel] | PTE24: [FTM4_CH4 | FTM Channel] | PTB1: [FTM4_CH5 | FTM Channel] | PTE13: [FTM4_CH5 | FTM Channel] | PTE25: [FTM4_CH5 | FTM Channel] | PTB0: [FTM4_CH6 | FTM Channel] | PTC28: [FTM4_CH7 | FTM Channel] | PTA25: [FTM5_CH0 | FTM Channel] | PTC9: [FTM5_CH0 | FTM Channel] | PTA26: [FTM5_CH1 | FTM Channel] | PTC8: [FTM5_CH1 | FTM Channel] | PTA27: [FTM5_CH2 | FTM Channel] | PTC29: [FTM5_CH2 | FTM Channel] | PTA7: [FTM5_CH3 | FTM Channel] | PTA28: [FTM5_CH3 | FTM Channel] | PTA29: [FTM5_CH4 | FTM Channel] | PTC30: [FTM5_CH4 | FTM Channel] | PTA6: [FTM5_CH5 | FTM Channel] | PTA30: [FTM5_CH5 | FTM Channel] | PTA31: [FTM5_CH6 | FTM Channel] | PTC31: [FTM5_CH6 | FTM Channel] | PTB18: [FTM5_CH7 | FTM Channel] | PTD18: [FTM5_CH7 | FTM Channel] | PTA18: [FTM6_CH0 | FTM Channel] | PTB20: [FTM6_CH0 | FTM Channel] | PTD19: [FTM6_CH0 | FTM Channel] | PTB21: [FTM6_CH1 | FTM Channel] | PTD20: [FTM6_CH1 | FTM Channel] | PTB22: [FTM6_CH2 | FTM Channel] | PTD21: [FTM6_CH2 | FTM Channel] | PTB23: [FTM6_CH3 | FTM Channel] | PTD22: [FTM6_CH3 | FTM Channel] | PTB24: [FTM6_CH4 | FTM Channel] | PTD23: [FTM6_CH4 | FTM Channel] | PTB25: [FTM6_CH5 | FTM Channel] | PTD24: [FTM6_CH5 | FTM Channel] | PTB26: [FTM6_CH6 | FTM Channel] | PTD25: [FTM6_CH6 | FTM Channel] | PTB27: [FTM6_CH7 | FTM Channel] | PTD26: [FTM6_CH7 | FTM Channel] | PTB28: [FTM7_CH0 | FTM Channel] | PTD27: [FTM7_CH0 | FTM Channel] | PTB29: [FTM7_CH1 | FTM Channel] | PTD28: [FTM7_CH1 | FTM Channel] | PTB30: [FTM7_CH2 | FTM Channel] | PTD29: [FTM7_CH2 | FTM Channel] | PTB31: [FTM7_CH3 | FTM Channel] | PTD30: [FTM7_CH3 | FTM Channel] | PTC18: [FTM7_CH4 | FTM Channel] | PTD31: [FTM7_CH4 | FTM Channel] | PTC19: [FTM7_CH5 | FTM Channel] | PTE17: [FTM7_CH5 | FTM Channel] | PTC20: [FTM7_CH6 | FTM Channel] | PTE18: [FTM7_CH6 | FTM Channel] | PTC21: [FTM7_CH7 | FTM Channel] | PTE19: [FTM7_CH7 | FTM Channel]
      mask TypeOptions pinFtm2Ch0: PTD15: [FTM0_CH0 | FTM Channel] | PTB13: [FTM0_CH1 | FTM Channel] | PTC1: [FTM0_CH1 | FTM Channel] | PTD16: [FTM0_CH1 | FTM Channel] | PTC2: [FTM0_CH2 | FTM Channel] | PTD0: [FTM0_CH2 | FTM Channel] | PTC3: [FTM0_CH3 | FTM Channel] | PTD1: [FTM0_CH3 | FTM Channel] | PTB4: [FTM0_CH4 | FTM Channel] | PTB5: [FTM0_CH5 | FTM Channel] | PTE8: [FTM0_CH6 | FTM Channel] | PTE9: [FTM0_CH7 | FTM Channel] | PTB2: [FTM1_CH0 | FTM Channel] | PTC4: [FTM1_CH0 | FTM Channel] | PTA1: [FTM1_CH1 | FTM Channel] | PTB3: [FTM1_CH1 | FTM Channel] | PTC14: [FTM1_CH2 | FTM Channel] | PTC15: [FTM1_CH3 | FTM Channel] | PTA10: [FTM1_CH4 | FTM Channel] | PTA11: [FTM1_CH5 | FTM Channel] | PTA12: [FTM1_CH6 | FTM Channel] | PTA13: [FTM1_CH7 | FTM Channel] | PTC1: [FTM1_CH7 | FTM Channel] | PTD15: [FTM0_CH0 | FTM Channel] | PTB13: [FTM0_CH1 | FTM Channel] | PTC1: [FTM0_CH1 | FTM Channel] | PTD16: [FTM0_CH1 | FTM Channel] | PTC2: [FTM0_CH2 | FTM Channel] | PTD0: [FTM0_CH2 | FTM Channel] | PTC3: [FTM0_CH3 | FTM Channel] | PTD1: [FTM0_CH3 | FTM Channel] | PTB4: [FTM0_CH4 | FTM Channel] | PTB5: [FTM0_CH5 | FTM Channel] | PTE8: [FTM0_CH6 | FTM Channel] | PTE9: [FTM0_CH7 | FTM Channel] | PTB2: [FTM1_CH0 | FTM Channel] | PTC4: [FTM1_CH0 | FTM Channel] | PTA1: [FTM1_CH1 | FTM Channel] | PTB3: [FTM1_CH1 | FTM Channel] | PTC14: [FTM1_CH2 | FTM Channel] | PTC15: [FTM1_CH3 | FTM Channel] | PTA10: [FTM1_CH4 | FTM Channel] | PTA11: [FTM1_CH5 | FTM Channel] | PTA12: [FTM1_CH6 | FTM Channel] | PTA13: [FTM1_CH7 | FTM Channel] | PTC1: [FTM1_CH7 | FTM Channel] | PTD15: [FTM0_CH0 | FTM Channel] | PTB13: [FTM0_CH1 | FTM Channel] | PTC1: [FTM0_CH1 | FTM Channel] | PTD16: [FTM0_CH1 | FTM Channel] | PTC2: [FTM0_CH2 | FTM Channel] | PTD0: [FTM0_CH2 | FTM Channel] | PTC3: [FTM0_CH3 | FTM Channel] | PTD1: [FTM0_CH3 | FTM Channel] | PTB4: [FTM0_CH4 | FTM Channel] | PTB5: [FTM0_CH5 | FTM Channel] | PTE8: [FTM0_CH6 | FTM Channel] | PTE9: [FTM0_CH7 | FTM Channel] | PTB2: [FTM1_CH0 | FTM Channel] | PTC4: [FTM1_CH0 | FTM Channel] | PTA1: [FTM1_CH1 | FTM Channel] | PTB3: [FTM1_CH1 | FTM Channel] | PTC14: [FTM1_CH2 | FTM Channel] | PTC15: [FTM1_CH3 | FTM Channel] | PTA10: [FTM1_CH4 | FTM Channel] | PTA11: [FTM1_CH5 | FTM Channel] | PTA12: [FTM1_CH6 | FTM Channel] | PTA13: [FTM1_CH7 | FTM Channel] | PTC1: [FTM1_CH7 | FTM Channel] | PTC5: [FTM2_CH0 | FTM Channel] | PTD0: [FTM2_CH0 | FTM Channel] | PTD10: [FTM2_CH0 | FTM Channel] | PTA0: [FTM2_CH1 | FTM Channel] | PTD1: [FTM2_CH1 | FTM Channel] | PTD11: [FTM2_CH1 | FTM Channel] | PTD12: [FTM2_CH2 | FTM Channel] | PTE4: [FTM2_CH2 | FTM Channel] | PTD5: [FTM2_CH3 | FTM Channel] | PTE5: [FTM2_CH3 | FTM Channel] | PTD13: [FTM2_CH4 | FTM Channel] | PTE10: [FTM2_CH4 | FTM Channel] | PTD14: [FTM2_CH5 | FTM Channel] | PTE11: [FTM2_CH5 | FTM Channel] | PTC12: [FTM2_CH6 | FTM Channel] | PTE15: [FTM2_CH6 | FTM Channel] | PTC13: [FTM2_CH7 | FTM Channel] | PTE16: [FTM2_CH7 | FTM Channel] | PTA2: [FTM3_CH0 | FTM Channel] | PTB8: [FTM3_CH0 | FTM Channel] | PTA3: [FTM3_CH1 | FTM Channel] | PTB9: [FTM3_CH1 | FTM Channel] | PTB10: [FTM3_CH2 | FTM Channel] | PTC6: [FTM3_CH2 | FTM Channel] | PTB11: [FTM3_CH3 | FTM Channel] | PTC7: [FTM3_CH3 | FTM Channel] | PTC10: [FTM3_CH4 | FTM Channel] | PTD2: [FTM3_CH4 | FTM Channel] | PTC11: [FTM3_CH5 | FTM Channel] | PTD3: [FTM3_CH5 | FTM Channel] | PTC12: [FTM3_CH6 | FTM Channel] | PTE2: [FTM3_CH6 | FTM Channel] | PTC13: [FTM3_CH7 | FTM Channel] | PTE6: [FTM3_CH7 | FTM Channel] | PTD15: [FTM0_CH0 | FTM Channel] | PTB13: [FTM0_CH1 | FTM Channel] | PTC1: [FTM0_CH1 | FTM Channel] | PTD16: [FTM0_CH1 | FTM Channel] | PTC2: [FTM0_CH2 | FTM Channel] | PTD0: [FTM0_CH2 | FTM Channel] | PTC3: [FTM0_CH3 | FTM Channel] | PTD1: [FTM0_CH3 | FTM Channel] | PTB4: [FTM0_CH4 | FTM Channel] | PTB5: [FTM0_CH5 | FTM Channel] | PTE8: [FTM0_CH6 | FTM Channel] | PTE9: [FTM0_CH7 | FTM Channel] | PTB2: [FTM1_CH0 | FTM Channel] | PTC4: [FTM1_CH0 | FTM Channel] | PTA1: [FTM1_CH1 | FTM Channel] | PTB3: [FTM1_CH1 | FTM Channel] | PTC14: [FTM1_CH2 | FTM Channel] | PTC15: [FTM1_CH3 | FTM Channel] | PTA10: [FTM1_CH4 | FTM Channel] | PTA11: [FTM1_CH5 | FTM Channel] | PTA12: [FTM1_CH6 | FTM Channel] | PTA13: [FTM1_CH7 | FTM Channel] | PTC1: [FTM1_CH7 | FTM Channel] | PTC5: [FTM2_CH0 | FTM Channel] | PTD0: [FTM2_CH0 | FTM Channel] | PTD10: [FTM2_CH0 | FTM Channel] | PTA0: [FTM2_CH1 | FTM Channel] | PTD1: [FTM2_CH1 | FTM Channel] | PTD11: [FTM2_CH1 | FTM Channel] | PTD12: [FTM2_CH2 | FTM Channel] | PTE4: [FTM2_CH2 | FTM Channel] | PTD5: [FTM2_CH3 | FTM Channel] | PTE5: [FTM2_CH3 | FTM Channel] | PTD13: [FTM2_CH4 | FTM Channel] | PTE10: [FTM2_CH4 | FTM Channel] | PTD14: [FTM2_CH5 | FTM Channel] | PTE11: [FTM2_CH5 | FTM Channel] | PTC12: [FTM2_CH6 | FTM Channel] | PTE15: [FTM2_CH6 | FTM Channel] | PTC13: [FTM2_CH7 | FTM Channel] | PTE16: [FTM2_CH7 | FTM Channel] | PTA2: [FTM3_CH0 | FTM Channel] | PTB8: [FTM3_CH0 | FTM Channel] | PTA3: [FTM3_CH1 | FTM Channel] | PTB9: [FTM3_CH1 | FTM Channel] | PTB10: [FTM3_CH2 | FTM Channel] | PTC6: [FTM3_CH2 | FTM Channel] | PTB11: [FTM3_CH3 | FTM Channel] | PTC7: [FTM3_CH3 | FTM Channel] | PTC10: [FTM3_CH4 | FTM Channel] | PTD2: [FTM3_CH4 | FTM Channel] | PTC11: [FTM3_CH5 | FTM Channel] | PTD3: [FTM3_CH5 | FTM Channel] | PTC12: [FTM3_CH6 | FTM Channel] | PTE2: [FTM3_CH6 | FTM Channel] | PTC13: [FTM3_CH7 | FTM Channel] | PTE6: [FTM3_CH7 | FTM Channel] | PTD15: [FTM0_CH0 | FTM Channel] | PTB13: [FTM0_CH1 | FTM Channel] | PTC1: [FTM0_CH1 | FTM Channel] | PTD16: [FTM0_CH1 | FTM Channel] | PTC2: [FTM0_CH2 | FTM Channel] | PTD0: [FTM0_CH2 | FTM Channel] | PTC3: [FTM0_CH3 | FTM Channel] | PTD1: [FTM0_CH3 | FTM Channel] | PTB4: [FTM0_CH4 | FTM Channel] | PTB5: [FTM0_CH5 | FTM Channel] | PTE8: [FTM0_CH6 | FTM Channel] | PTE9: [FTM0_CH7 | FTM Channel] | PTB2: [FTM1_CH0 | FTM Channel] | PTC4: [FTM1_CH0 | FTM Channel] | PTA1: [FTM1_CH1 | FTM Channel] | PTB3: [FTM1_CH1 | FTM Channel] | PTC14: [FTM1_CH2 | FTM Channel] | PTC15: [FTM1_CH3 | FTM Channel] | PTA10: [FTM1_CH4 | FTM Channel] | PTA11: [FTM1_CH5 | FTM Channel] | PTA12: [FTM1_CH6 | FTM Channel] | PTA13: [FTM1_CH7 | FTM Channel] | PTC1: [FTM1_CH7 | FTM Channel] | PTC5: [FTM2_CH0 | FTM Channel] | PTD0: [FTM2_CH0 | FTM Channel] | PTD10: [FTM2_CH0 | FTM Channel] | PTA0: [FTM2_CH1 | FTM Channel] | PTD1: [FTM2_CH1 | FTM Channel] | PTD11: [FTM2_CH1 | FTM Channel] | PTD12: [FTM2_CH2 | FTM Channel] | PTE4: [FTM2_CH2 | FTM Channel] | PTD5: [FTM2_CH3 | FTM Channel] | PTE5: [FTM2_CH3 | FTM Channel] | PTD13: [FTM2_CH4 | FTM Channel] | PTE10: [FTM2_CH4 | FTM Channel] | PTD14: [FTM2_CH5 | FTM Channel] | PTE11: [FTM2_CH5 | FTM Channel] | PTC12: [FTM2_CH6 | FTM Channel] | PTE15: [FTM2_CH6 | FTM Channel] | PTC13: [FTM2_CH7 | FTM Channel] | PTE16: [FTM2_CH7 | FTM Channel] | PTA2: [FTM3_CH0 | FTM Channel] | PTB8: [FTM3_CH0 | FTM Channel] | PTA3: [FTM3_CH1 | FTM Channel] | PTB9: [FTM3_CH1 | FTM Channel] | PTB10: [FTM3_CH2 | FTM Channel] | PTC6: [FTM3_CH2 | FTM Channel] | PTB11: [FTM3_CH3 | FTM Channel] | PTC7: [FTM3_CH3 | FTM Channel] | PTC10: [FTM3_CH4 | FTM Channel] | PTD2: [FTM3_CH4 | FTM Channel] | PTC11: [FTM3_CH5 | FTM Channel] | PTD3: [FTM3_CH5 | FTM Channel] | PTC12: [FTM3_CH6 | FTM Channel] | PTE2: [FTM3_CH6 | FTM Channel] | PTC13: [FTM3_CH7 | FTM Channel] | PTE6: [FTM3_CH7 | FTM Channel] | PTE20: [FTM4_CH0 | FTM Channel] | PTE21: [FTM4_CH1 | FTM Channel] | PTC11: [FTM4_CH2 | FTM Channel] | PTE22: [FTM4_CH2 | FTM Channel] | PTE23: [FTM4_CH3 | FTM Channel] | PTC27: [FTM4_CH4 | FTM Channel] | PTE24: [FTM4_CH4 | FTM Channel] | PTB1: [FTM4_CH5 | FTM Channel] | PTE13: [FTM4_CH5 | FTM Channel] | PTE25: [FTM4_CH5 | FTM Channel] | PTB0: [FTM4_CH6 | FTM Channel] | PTC28: [FTM4_CH7 | FTM Channel] | PTA25: [FTM5_CH0 | FTM Channel] | PTC9: [FTM5_CH0 | FTM Channel] | PTA26: [FTM5_CH1 | FTM Channel] | PTC8: [FTM5_CH1 | FTM Channel] | PTA27: [FTM5_CH2 | FTM Channel] | PTC29: [FTM5_CH2 | FTM Channel] | PTA7: [FTM5_CH3 | FTM Channel] | PTA28: [FTM5_CH3 | FTM Channel] | PTA29: [FTM5_CH4 | FTM Channel] | PTC30: [FTM5_CH4 | FTM Channel] | PTA6: [FTM5_CH5 | FTM Channel] | PTA30: [FTM5_CH5 | FTM Channel] | PTA31: [FTM5_CH6 | FTM Channel] | PTC31: [FTM5_CH6 | FTM Channel] | PTB18: [FTM5_CH7 | FTM Channel] | PTD18: [FTM5_CH7 | FTM Channel] | PTD15: [FTM0_CH0 | FTM Channel] | PTB13: [FTM0_CH1 | FTM Channel] | PTC1: [FTM0_CH1 | FTM Channel] | PTD16: [FTM0_CH1 | FTM Channel] | PTC2: [FTM0_CH2 | FTM Channel] | PTD0: [FTM0_CH2 | FTM Channel] | PTC3: [FTM0_CH3 | FTM Channel] | PTD1: [FTM0_CH3 | FTM Channel] | PTB4: [FTM0_CH4 | FTM Channel] | PTB5: [FTM0_CH5 | FTM Channel] | PTE8: [FTM0_CH6 | FTM Channel] | PTE9: [FTM0_CH7 | FTM Channel] | PTB2: [FTM1_CH0 | FTM Channel] | PTC4: [FTM1_CH0 | FTM Channel] | PTA1: [FTM1_CH1 | FTM Channel] | PTB3: [FTM1_CH1 | FTM Channel] | PTC14: [FTM1_CH2 | FTM Channel] | PTC15: [FTM1_CH3 | FTM Channel] | PTA10: [FTM1_CH4 | FTM Channel] | PTA11: [FTM1_CH5 | FTM Channel] | PTA12: [FTM1_CH6 | FTM Channel] | PTA13: [FTM1_CH7 | FTM Channel] | PTC1: [FTM1_CH7 | FTM Channel] | PTC5: [FTM2_CH0 | FTM Channel] | PTD0: [FTM2_CH0 | FTM Channel] | PTD10: [FTM2_CH0 | FTM Channel] | PTA0: [FTM2_CH1 | FTM Channel] | PTD1: [FTM2_CH1 | FTM Channel] | PTD11: [FTM2_CH1 | FTM Channel] | PTD12: [FTM2_CH2 | FTM Channel] | PTE4: [FTM2_CH2 | FTM Channel] | PTD5: [FTM2_CH3 | FTM Channel] | PTE5: [FTM2_CH3 | FTM Channel] | PTD13: [FTM2_CH4 | FTM Channel] | PTE10: [FTM2_CH4 | FTM Channel] | PTD14: [FTM2_CH5 | FTM Channel] | PTE11: [FTM2_CH5 | FTM Channel] | PTC12: [FTM2_CH6 | FTM Channel] | PTE15: [FTM2_CH6 | FTM Channel] | PTC13: [FTM2_CH7 | FTM Channel] | PTE16: [FTM2_CH7 | FTM Channel] | PTA2: [FTM3_CH0 | FTM Channel] | PTB8: [FTM3_CH0 | FTM Channel] | PTA3: [FTM3_CH1 | FTM Channel] | PTB9: [FTM3_CH1 | FTM Channel] | PTB10: [FTM3_CH2 | FTM Channel] | PTC6: [FTM3_CH2 | FTM Channel] | PTB11: [FTM3_CH3 | FTM Channel] | PTC7: [FTM3_CH3 | FTM Channel] | PTC10: [FTM3_CH4 | FTM Channel] | PTD2: [FTM3_CH4 | FTM Channel] | PTC11: [FTM3_CH5 | FTM Channel] | PTD3: [FTM3_CH5 | FTM Channel] | PTC12: [FTM3_CH6 | FTM Channel] | PTE2: [FTM3_CH6 | FTM Channel] | PTC13: [FTM3_CH7 | FTM Channel] | PTE6: [FTM3_CH7 | FTM Channel] | PTE20: [FTM4_CH0 | FTM Channel] | PTE21: [FTM4_CH1 | FTM Channel] | PTC11: [FTM4_CH2 | FTM Channel] | PTE22: [FTM4_CH2 | FTM Channel] | PTE23: [FTM4_CH3 | FTM Channel] | PTC27: [FTM4_CH4 | FTM Channel] | PTE24: [FTM4_CH4 | FTM Channel] | PTB1: [FTM4_CH5 | FTM Channel] | PTE13: [FTM4_CH5 | FTM Channel] | PTE25: [FTM4_CH5 | FTM Channel] | PTB0: [FTM4_CH6 | FTM Channel] | PTC28: [FTM4_CH7 | FTM Channel] | PTA25: [FTM5_CH0 | FTM Channel] | PTC9: [FTM5_CH0 | FTM Channel] | PTA26: [FTM5_CH1 | FTM Channel] | PTC8: [FTM5_CH1 | FTM Channel] | PTA27: [FTM5_CH2 | FTM Channel] | PTC29: [FTM5_CH2 | FTM Channel] | PTA7: [FTM5_CH3 | FTM Channel] | PTA28: [FTM5_CH3 | FTM Channel] | PTA29: [FTM5_CH4 | FTM Channel] | PTC30: [FTM5_CH4 | FTM Channel] | PTA6: [FTM5_CH5 | FTM Channel] | PTA30: [FTM5_CH5 | FTM Channel] | PTA31: [FTM5_CH6 | FTM Channel] | PTC31: [FTM5_CH6 | FTM Channel] | PTB18: [FTM5_CH7 | FTM Channel] | PTD18: [FTM5_CH7 | FTM Channel] | PTA18: [FTM6_CH0 | FTM Channel] | PTB20: [FTM6_CH0 | FTM Channel] | PTD19: [FTM6_CH0 | FTM Channel] | PTB21: [FTM6_CH1 | FTM Channel] | PTD20: [FTM6_CH1 | FTM Channel] | PTB22: [FTM6_CH2 | FTM Channel] | PTD21: [FTM6_CH2 | FTM Channel] | PTB23: [FTM6_CH3 | FTM Channel] | PTD22: [FTM6_CH3 | FTM Channel] | PTB24: [FTM6_CH4 | FTM Channel] | PTD23: [FTM6_CH4 | FTM Channel] | PTB25: [FTM6_CH5 | FTM Channel] | PTD24: [FTM6_CH5 | FTM Channel] | PTB26: [FTM6_CH6 | FTM Channel] | PTD25: [FTM6_CH6 | FTM Channel] | PTB27: [FTM6_CH7 | FTM Channel] | PTD26: [FTM6_CH7 | FTM Channel] | PTB28: [FTM7_CH0 | FTM Channel] | PTD27: [FTM7_CH0 | FTM Channel] | PTB29: [FTM7_CH1 | FTM Channel] | PTD28: [FTM7_CH1 | FTM Channel] | PTB30: [FTM7_CH2 | FTM Channel] | PTD29: [FTM7_CH2 | FTM Channel] | PTB31: [FTM7_CH3 | FTM Channel] | PTD30: [FTM7_CH3 | FTM Channel] | PTC18: [FTM7_CH4 | FTM Channel] | PTD31: [FTM7_CH4 | FTM Channel] | PTC19: [FTM7_CH5 | FTM Channel] | PTE17: [FTM7_CH5 | FTM Channel] | PTC20: [FTM7_CH6 | FTM Channel] | PTE18: [FTM7_CH6 | FTM Channel] | PTC21: [FTM7_CH7 | FTM Channel] | PTE19: [FTM7_CH7 | FTM Channel]
      mask TypeOptions pinFtm2Ch1: PTD15: [FTM0_CH0 | FTM Channel] | PTB13: [FTM0_CH1 | FTM Channel] | PTC1: [FTM0_CH1 | FTM Channel] | PTD16: [FTM0_CH1 | FTM Channel] | PTC2: [FTM0_CH2 | FTM Channel] | PTD0: [FTM0_CH2 | FTM Channel] | PTC3: [FTM0_CH3 | FTM Channel] | PTD1: [FTM0_CH3 | FTM Channel] | PTB4: [FTM0_CH4 | FTM Channel] | PTB5: [FTM0_CH5 | FTM Channel] | PTE8: [FTM0_CH6 | FTM Channel] | PTE9: [FTM0_CH7 | FTM Channel] | PTB2: [FTM1_CH0 | FTM Channel] | PTC4: [FTM1_CH0 | FTM Channel] | PTA1: [FTM1_CH1 | FTM Channel] | PTB3: [FTM1_CH1 | FTM Channel] | PTC14: [FTM1_CH2 | FTM Channel] | PTC15: [FTM1_CH3 | FTM Channel] | PTA10: [FTM1_CH4 | FTM Channel] | PTA11: [FTM1_CH5 | FTM Channel] | PTA12: [FTM1_CH6 | FTM Channel] | PTA13: [FTM1_CH7 | FTM Channel] | PTC1: [FTM1_CH7 | FTM Channel] | PTD15: [FTM0_CH0 | FTM Channel] | PTB13: [FTM0_CH1 | FTM Channel] | PTC1: [FTM0_CH1 | FTM Channel] | PTD16: [FTM0_CH1 | FTM Channel] | PTC2: [FTM0_CH2 | FTM Channel] | PTD0: [FTM0_CH2 | FTM Channel] | PTC3: [FTM0_CH3 | FTM Channel] | PTD1: [FTM0_CH3 | FTM Channel] | PTB4: [FTM0_CH4 | FTM Channel] | PTB5: [FTM0_CH5 | FTM Channel] | PTE8: [FTM0_CH6 | FTM Channel] | PTE9: [FTM0_CH7 | FTM Channel] | PTB2: [FTM1_CH0 | FTM Channel] | PTC4: [FTM1_CH0 | FTM Channel] | PTA1: [FTM1_CH1 | FTM Channel] | PTB3: [FTM1_CH1 | FTM Channel] | PTC14: [FTM1_CH2 | FTM Channel] | PTC15: [FTM1_CH3 | FTM Channel] | PTA10: [FTM1_CH4 | FTM Channel] | PTA11: [FTM1_CH5 | FTM Channel] | PTA12: [FTM1_CH6 | FTM Channel] | PTA13: [FTM1_CH7 | FTM Channel] | PTC1: [FTM1_CH7 | FTM Channel] | PTD15: [FTM0_CH0 | FTM Channel] | PTB13: [FTM0_CH1 | FTM Channel] | PTC1: [FTM0_CH1 | FTM Channel] | PTD16: [FTM0_CH1 | FTM Channel] | PTC2: [FTM0_CH2 | FTM Channel] | PTD0: [FTM0_CH2 | FTM Channel] | PTC3: [FTM0_CH3 | FTM Channel] | PTD1: [FTM0_CH3 | FTM Channel] | PTB4: [FTM0_CH4 | FTM Channel] | PTB5: [FTM0_CH5 | FTM Channel] | PTE8: [FTM0_CH6 | FTM Channel] | PTE9: [FTM0_CH7 | FTM Channel] | PTB2: [FTM1_CH0 | FTM Channel] | PTC4: [FTM1_CH0 | FTM Channel] | PTA1: [FTM1_CH1 | FTM Channel] | PTB3: [FTM1_CH1 | FTM Channel] | PTC14: [FTM1_CH2 | FTM Channel] | PTC15: [FTM1_CH3 | FTM Channel] | PTA10: [FTM1_CH4 | FTM Channel] | PTA11: [FTM1_CH5 | FTM Channel] | PTA12: [FTM1_CH6 | FTM Channel] | PTA13: [FTM1_CH7 | FTM Channel] | PTC1: [FTM1_CH7 | FTM Channel] | PTC5: [FTM2_CH0 | FTM Channel] | PTD0: [FTM2_CH0 | FTM Channel] | PTD10: [FTM2_CH0 | FTM Channel] | PTA0: [FTM2_CH1 | FTM Channel] | PTD1: [FTM2_CH1 | FTM Channel] | PTD11: [FTM2_CH1 | FTM Channel] | PTD12: [FTM2_CH2 | FTM Channel] | PTE4: [FTM2_CH2 | FTM Channel] | PTD5: [FTM2_CH3 | FTM Channel] | PTE5: [FTM2_CH3 | FTM Channel] | PTD13: [FTM2_CH4 | FTM Channel] | PTE10: [FTM2_CH4 | FTM Channel] | PTD14: [FTM2_CH5 | FTM Channel] | PTE11: [FTM2_CH5 | FTM Channel] | PTC12: [FTM2_CH6 | FTM Channel] | PTE15: [FTM2_CH6 | FTM Channel] | PTC13: [FTM2_CH7 | FTM Channel] | PTE16: [FTM2_CH7 | FTM Channel] | PTA2: [FTM3_CH0 | FTM Channel] | PTB8: [FTM3_CH0 | FTM Channel] | PTA3: [FTM3_CH1 | FTM Channel] | PTB9: [FTM3_CH1 | FTM Channel] | PTB10: [FTM3_CH2 | FTM Channel] | PTC6: [FTM3_CH2 | FTM Channel] | PTB11: [FTM3_CH3 | FTM Channel] | PTC7: [FTM3_CH3 | FTM Channel] | PTC10: [FTM3_CH4 | FTM Channel] | PTD2: [FTM3_CH4 | FTM Channel] | PTC11: [FTM3_CH5 | FTM Channel] | PTD3: [FTM3_CH5 | FTM Channel] | PTC12: [FTM3_CH6 | FTM Channel] | PTE2: [FTM3_CH6 | FTM Channel] | PTC13: [FTM3_CH7 | FTM Channel] | PTE6: [FTM3_CH7 | FTM Channel] | PTD15: [FTM0_CH0 | FTM Channel] | PTB13: [FTM0_CH1 | FTM Channel] | PTC1: [FTM0_CH1 | FTM Channel] | PTD16: [FTM0_CH1 | FTM Channel] | PTC2: [FTM0_CH2 | FTM Channel] | PTD0: [FTM0_CH2 | FTM Channel] | PTC3: [FTM0_CH3 | FTM Channel] | PTD1: [FTM0_CH3 | FTM Channel] | PTB4: [FTM0_CH4 | FTM Channel] | PTB5: [FTM0_CH5 | FTM Channel] | PTE8: [FTM0_CH6 | FTM Channel] | PTE9: [FTM0_CH7 | FTM Channel] | PTB2: [FTM1_CH0 | FTM Channel] | PTC4: [FTM1_CH0 | FTM Channel] | PTA1: [FTM1_CH1 | FTM Channel] | PTB3: [FTM1_CH1 | FTM Channel] | PTC14: [FTM1_CH2 | FTM Channel] | PTC15: [FTM1_CH3 | FTM Channel] | PTA10: [FTM1_CH4 | FTM Channel] | PTA11: [FTM1_CH5 | FTM Channel] | PTA12: [FTM1_CH6 | FTM Channel] | PTA13: [FTM1_CH7 | FTM Channel] | PTC1: [FTM1_CH7 | FTM Channel] | PTC5: [FTM2_CH0 | FTM Channel] | PTD0: [FTM2_CH0 | FTM Channel] | PTD10: [FTM2_CH0 | FTM Channel] | PTA0: [FTM2_CH1 | FTM Channel] | PTD1: [FTM2_CH1 | FTM Channel] | PTD11: [FTM2_CH1 | FTM Channel] | PTD12: [FTM2_CH2 | FTM Channel] | PTE4: [FTM2_CH2 | FTM Channel] | PTD5: [FTM2_CH3 | FTM Channel] | PTE5: [FTM2_CH3 | FTM Channel] | PTD13: [FTM2_CH4 | FTM Channel] | PTE10: [FTM2_CH4 | FTM Channel] | PTD14: [FTM2_CH5 | FTM Channel] | PTE11: [FTM2_CH5 | FTM Channel] | PTC12: [FTM2_CH6 | FTM Channel] | PTE15: [FTM2_CH6 | FTM Channel] | PTC13: [FTM2_CH7 | FTM Channel] | PTE16: [FTM2_CH7 | FTM Channel] | PTA2: [FTM3_CH0 | FTM Channel] | PTB8: [FTM3_CH0 | FTM Channel] | PTA3: [FTM3_CH1 | FTM Channel] | PTB9: [FTM3_CH1 | FTM Channel] | PTB10: [FTM3_CH2 | FTM Channel] | PTC6: [FTM3_CH2 | FTM Channel] | PTB11: [FTM3_CH3 | FTM Channel] | PTC7: [FTM3_CH3 | FTM Channel] | PTC10: [FTM3_CH4 | FTM Channel] | PTD2: [FTM3_CH4 | FTM Channel] | PTC11: [FTM3_CH5 | FTM Channel] | PTD3: [FTM3_CH5 | FTM Channel] | PTC12: [FTM3_CH6 | FTM Channel] | PTE2: [FTM3_CH6 | FTM Channel] | PTC13: [FTM3_CH7 | FTM Channel] | PTE6: [FTM3_CH7 | FTM Channel] | PTD15: [FTM0_CH0 | FTM Channel] | PTB13: [FTM0_CH1 | FTM Channel] | PTC1: [FTM0_CH1 | FTM Channel] | PTD16: [FTM0_CH1 | FTM Channel] | PTC2: [FTM0_CH2 | FTM Channel] | PTD0: [FTM0_CH2 | FTM Channel] | PTC3: [FTM0_CH3 | FTM Channel] | PTD1: [FTM0_CH3 | FTM Channel] | PTB4: [FTM0_CH4 | FTM Channel] | PTB5: [FTM0_CH5 | FTM Channel] | PTE8: [FTM0_CH6 | FTM Channel] | PTE9: [FTM0_CH7 | FTM Channel] | PTB2: [FTM1_CH0 | FTM Channel] | PTC4: [FTM1_CH0 | FTM Channel] | PTA1: [FTM1_CH1 | FTM Channel] | PTB3: [FTM1_CH1 | FTM Channel] | PTC14: [FTM1_CH2 | FTM Channel] | PTC15: [FTM1_CH3 | FTM Channel] | PTA10: [FTM1_CH4 | FTM Channel] | PTA11: [FTM1_CH5 | FTM Channel] | PTA12: [FTM1_CH6 | FTM Channel] | PTA13: [FTM1_CH7 | FTM Channel] | PTC1: [FTM1_CH7 | FTM Channel] | PTC5: [FTM2_CH0 | FTM Channel] | PTD0: [FTM2_CH0 | FTM Channel] | PTD10: [FTM2_CH0 | FTM Channel] | PTA0: [FTM2_CH1 | FTM Channel] | PTD1: [FTM2_CH1 | FTM Channel] | PTD11: [FTM2_CH1 | FTM Channel] | PTD12: [FTM2_CH2 | FTM Channel] | PTE4: [FTM2_CH2 | FTM Channel] | PTD5: [FTM2_CH3 | FTM Channel] | PTE5: [FTM2_CH3 | FTM Channel] | PTD13: [FTM2_CH4 | FTM Channel] | PTE10: [FTM2_CH4 | FTM Channel] | PTD14: [FTM2_CH5 | FTM Channel] | PTE11: [FTM2_CH5 | FTM Channel] | PTC12: [FTM2_CH6 | FTM Channel] | PTE15: [FTM2_CH6 | FTM Channel] | PTC13: [FTM2_CH7 | FTM Channel] | PTE16: [FTM2_CH7 | FTM Channel] | PTA2: [FTM3_CH0 | FTM Channel] | PTB8: [FTM3_CH0 | FTM Channel] | PTA3: [FTM3_CH1 | FTM Channel] | PTB9: [FTM3_CH1 | FTM Channel] | PTB10: [FTM3_CH2 | FTM Channel] | PTC6: [FTM3_CH2 | FTM Channel] | PTB11: [FTM3_CH3 | FTM Channel] | PTC7: [FTM3_CH3 | FTM Channel] | PTC10: [FTM3_CH4 | FTM Channel] | PTD2: [FTM3_CH4 | FTM Channel] | PTC11: [FTM3_CH5 | FTM Channel] | PTD3: [FTM3_CH5 | FTM Channel] | PTC12: [FTM3_CH6 | FTM Channel] | PTE2: [FTM3_CH6 | FTM Channel] | PTC13: [FTM3_CH7 | FTM Channel] | PTE6: [FTM3_CH7 | FTM Channel] | PTE20: [FTM4_CH0 | FTM Channel] | PTE21: [FTM4_CH1 | FTM Channel] | PTC11: [FTM4_CH2 | FTM Channel] | PTE22: [FTM4_CH2 | FTM Channel] | PTE23: [FTM4_CH3 | FTM Channel] | PTC27: [FTM4_CH4 | FTM Channel] | PTE24: [FTM4_CH4 | FTM Channel] | PTB1: [FTM4_CH5 | FTM Channel] | PTE13: [FTM4_CH5 | FTM Channel] | PTE25: [FTM4_CH5 | FTM Channel] | PTB0: [FTM4_CH6 | FTM Channel] | PTC28: [FTM4_CH7 | FTM Channel] | PTA25: [FTM5_CH0 | FTM Channel] | PTC9: [FTM5_CH0 | FTM Channel] | PTA26: [FTM5_CH1 | FTM Channel] | PTC8: [FTM5_CH1 | FTM Channel] | PTA27: [FTM5_CH2 | FTM Channel] | PTC29: [FTM5_CH2 | FTM Channel] | PTA7: [FTM5_CH3 | FTM Channel] | PTA28: [FTM5_CH3 | FTM Channel] | PTA29: [FTM5_CH4 | FTM Channel] | PTC30: [FTM5_CH4 | FTM Channel] | PTA6: [FTM5_CH5 | FTM Channel] | PTA30: [FTM5_CH5 | FTM Channel] | PTA31: [FTM5_CH6 | FTM Channel] | PTC31: [FTM5_CH6 | FTM Channel] | PTB18: [FTM5_CH7 | FTM Channel] | PTD18: [FTM5_CH7 | FTM Channel] | PTD15: [FTM0_CH0 | FTM Channel] | PTB13: [FTM0_CH1 | FTM Channel] | PTC1: [FTM0_CH1 | FTM Channel] | PTD16: [FTM0_CH1 | FTM Channel] | PTC2: [FTM0_CH2 | FTM Channel] | PTD0: [FTM0_CH2 | FTM Channel] | PTC3: [FTM0_CH3 | FTM Channel] | PTD1: [FTM0_CH3 | FTM Channel] | PTB4: [FTM0_CH4 | FTM Channel] | PTB5: [FTM0_CH5 | FTM Channel] | PTE8: [FTM0_CH6 | FTM Channel] | PTE9: [FTM0_CH7 | FTM Channel] | PTB2: [FTM1_CH0 | FTM Channel] | PTC4: [FTM1_CH0 | FTM Channel] | PTA1: [FTM1_CH1 | FTM Channel] | PTB3: [FTM1_CH1 | FTM Channel] | PTC14: [FTM1_CH2 | FTM Channel] | PTC15: [FTM1_CH3 | FTM Channel] | PTA10: [FTM1_CH4 | FTM Channel] | PTA11: [FTM1_CH5 | FTM Channel] | PTA12: [FTM1_CH6 | FTM Channel] | PTA13: [FTM1_CH7 | FTM Channel] | PTC1: [FTM1_CH7 | FTM Channel] | PTC5: [FTM2_CH0 | FTM Channel] | PTD0: [FTM2_CH0 | FTM Channel] | PTD10: [FTM2_CH0 | FTM Channel] | PTA0: [FTM2_CH1 | FTM Channel] | PTD1: [FTM2_CH1 | FTM Channel] | PTD11: [FTM2_CH1 | FTM Channel] | PTD12: [FTM2_CH2 | FTM Channel] | PTE4: [FTM2_CH2 | FTM Channel] | PTD5: [FTM2_CH3 | FTM Channel] | PTE5: [FTM2_CH3 | FTM Channel] | PTD13: [FTM2_CH4 | FTM Channel] | PTE10: [FTM2_CH4 | FTM Channel] | PTD14: [FTM2_CH5 | FTM Channel] | PTE11: [FTM2_CH5 | FTM Channel] | PTC12: [FTM2_CH6 | FTM Channel] | PTE15: [FTM2_CH6 | FTM Channel] | PTC13: [FTM2_CH7 | FTM Channel] | PTE16: [FTM2_CH7 | FTM Channel] | PTA2: [FTM3_CH0 | FTM Channel] | PTB8: [FTM3_CH0 | FTM Channel] | PTA3: [FTM3_CH1 | FTM Channel] | PTB9: [FTM3_CH1 | FTM Channel] | PTB10: [FTM3_CH2 | FTM Channel] | PTC6: [FTM3_CH2 | FTM Channel] | PTB11: [FTM3_CH3 | FTM Channel] | PTC7: [FTM3_CH3 | FTM Channel] | PTC10: [FTM3_CH4 | FTM Channel] | PTD2: [FTM3_CH4 | FTM Channel] | PTC11: [FTM3_CH5 | FTM Channel] | PTD3: [FTM3_CH5 | FTM Channel] | PTC12: [FTM3_CH6 | FTM Channel] | PTE2: [FTM3_CH6 | FTM Channel] | PTC13: [FTM3_CH7 | FTM Channel] | PTE6: [FTM3_CH7 | FTM Channel] | PTE20: [FTM4_CH0 | FTM Channel] | PTE21: [FTM4_CH1 | FTM Channel] | PTC11: [FTM4_CH2 | FTM Channel] | PTE22: [FTM4_CH2 | FTM Channel] | PTE23: [FTM4_CH3 | FTM Channel] | PTC27: [FTM4_CH4 | FTM Channel] | PTE24: [FTM4_CH4 | FTM Channel] | PTB1: [FTM4_CH5 | FTM Channel] | PTE13: [FTM4_CH5 | FTM Channel] | PTE25: [FTM4_CH5 | FTM Channel] | PTB0: [FTM4_CH6 | FTM Channel] | PTC28: [FTM4_CH7 | FTM Channel] | PTA25: [FTM5_CH0 | FTM Channel] | PTC9: [FTM5_CH0 | FTM Channel] | PTA26: [FTM5_CH1 | FTM Channel] | PTC8: [FTM5_CH1 | FTM Channel] | PTA27: [FTM5_CH2 | FTM Channel] | PTC29: [FTM5_CH2 | FTM Channel] | PTA7: [FTM5_CH3 | FTM Channel] | PTA28: [FTM5_CH3 | FTM Channel] | PTA29: [FTM5_CH4 | FTM Channel] | PTC30: [FTM5_CH4 | FTM Channel] | PTA6: [FTM5_CH5 | FTM Channel] | PTA30: [FTM5_CH5 | FTM Channel] | PTA31: [FTM5_CH6 | FTM Channel] | PTC31: [FTM5_CH6 | FTM Channel] | PTB18: [FTM5_CH7 | FTM Channel] | PTD18: [FTM5_CH7 | FTM Channel] | PTA18: [FTM6_CH0 | FTM Channel] | PTB20: [FTM6_CH0 | FTM Channel] | PTD19: [FTM6_CH0 | FTM Channel] | PTB21: [FTM6_CH1 | FTM Channel] | PTD20: [FTM6_CH1 | FTM Channel] | PTB22: [FTM6_CH2 | FTM Channel] | PTD21: [FTM6_CH2 | FTM Channel] | PTB23: [FTM6_CH3 | FTM Channel] | PTD22: [FTM6_CH3 | FTM Channel] | PTB24: [FTM6_CH4 | FTM Channel] | PTD23: [FTM6_CH4 | FTM Channel] | PTB25: [FTM6_CH5 | FTM Channel] | PTD24: [FTM6_CH5 | FTM Channel] | PTB26: [FTM6_CH6 | FTM Channel] | PTD25: [FTM6_CH6 | FTM Channel] | PTB27: [FTM6_CH7 | FTM Channel] | PTD26: [FTM6_CH7 | FTM Channel] | PTB28: [FTM7_CH0 | FTM Channel] | PTD27: [FTM7_CH0 | FTM Channel] | PTB29: [FTM7_CH1 | FTM Channel] | PTD28: [FTM7_CH1 | FTM Channel] | PTB30: [FTM7_CH2 | FTM Channel] | PTD29: [FTM7_CH2 | FTM Channel] | PTB31: [FTM7_CH3 | FTM Channel] | PTD30: [FTM7_CH3 | FTM Channel] | PTC18: [FTM7_CH4 | FTM Channel] | PTD31: [FTM7_CH4 | FTM Channel] | PTC19: [FTM7_CH5 | FTM Channel] | PTE17: [FTM7_CH5 | FTM Channel] | PTC20: [FTM7_CH6 | FTM Channel] | PTE18: [FTM7_CH6 | FTM Channel] | PTC21: [FTM7_CH7 | FTM Channel] | PTE19: [FTM7_CH7 | FTM Channel]
      mask Display:
      | image('nxp_logo.png', 'top-right');
      | port_label('output',1,'Trigger');
      | port_label('output',2,'FTM Counter');
      | disp(maskStr);
  FTM_ISR_Disable_Enable : S-Function  FunctionName=ftm_s32k_isr_disen  Parameters=ftmModule,channel,dis  SFunctionDeploymentMode=off  EnableBusSupport=off  mask(FTM_s32k_isr_disen){ftmModule=0, channel=TOF, dis=interrupt source Disable, mcuTargetUpdate=0}
      mask prompts: ftmModule "Module"; channel "Interrupt source"; dis "Enable/Disable"
      mask help: This block allows user to Enable\Disable FTM ISR routine.
      mask init:
      | mbd_s32k_ftm_display_modules(gcb);
      | 
      | st = [ 'FTM ISR Disable Enable', newline, newline, ...
      |     'Module: ', get_param(gcb,'ftmModule'), newline, ...
      |     get_param(gcb, 'channel'), ' ', get_param(gcb,'dis') ];
      settings: NameChangeFcn=mbd_s32k_name_check(gcb);
      mask Help: web(fullfile(mbd_s32k_block_help, 'ftm', 'ftm_isr_endis.html'));
      mask TypeOptions ftmModule: 0 | 1 | 2 | 3 | 4 | 5 | 6 | 7
      mask Callback ftmModule: mbd_s32k_ftm_display_modules(gcb);
      mask TypeOptions channel: TOF | channel 0 | channel 1 | channel 2 | channel 3 | channel 4 | channel 5 | channel 6 | channel 7
      mask TypeOptions dis: interrupt source Disable | interrupt source Enable
      mask Display:
      | image('nxp_logo.png', 'top-right');
      | disp(st);
  FTM_Init_Trigger_Disable_Enable : S-Function  FunctionName=ftm_s32k_init_disen  SFunctionDeploymentMode=off  EnableBusSupport=off  mask(FTM_s32k_init_disen){ftmModule=0, action=Disable}
      mask prompts: ftmModule "Module"
      mask help: Disables/Enables the PWM Init Trigger for the selected PWM module.
      mask init:
      | mbd_s32k_ftm_display_modules(gcb);
      | maskStr = ['FTM PWM Init Trigger Disable Enable', newline, newline, ...
      |     'Module : ', get_param(gcb,'ftmModule'), newline, ...
      |     ' Action : ', get_param(gcb,'action') ];
      settings: NameChangeFcn=mbd_s32k_name_check(gcb);
      mask Help: web(fullfile(mbd_s32k_block_help, 'ftm', 'ftm_init_disen.html'));
      mask TypeOptions ftmModule: 0 | 1 | 2 | 3 | 4 | 5 | 6 | 7
      mask TypeOptions action: Disable | Enable
      mask Display:
      | image('nxp_logo.png', 'top-right');
      | disp(maskStr);
  FTM_Ovf_Reload_ISR : S-Function  Priority=10  FunctionName=ftm_s32k_ovf_reload_isr  Parameters=sFuncParams  SFunctionDeploymentMode=off  EnableBusSupport=off  mask(FTM_s32k_ovf_reload_isr){ftmModule=0, mcuTargetUpdate=on}
      mask prompts: ftmModule "Module"; mcuTargetUpdate "Mcu target update"
      mask help: FTM Channel timer overflow reload interrupt handler for PWM blocks.
      mask init:
      | mbd_s32k_ftm_display_modules(gcb);
      | maskStr = [ 'FTM PWM Overflow ISR', newline, newline, ...
      |             'Module : ', get_param(gcb,'ftmModule')];
      | sFuncParams = [];
      settings: NameChangeFcn=mbd_s32k_name_check(gcb);
      mask Help: web(fullfile(mbd_s32k_block_help, 'ftm', 'ftm_ovf_reload_isr_block.html'));
      mask TypeOptions ftmModule: 0 | 1 | 2 | 3 | 4 | 5 | 6 | 7
      mask Display:
      | image('nxp_logo.png', 'top-right');
      | disp(maskStr);
      | port_label('output',1,'function');
  FTM_PWM_Config : S-Function  FunctionName=ftm_s32k_pwm_config  Parameters=funcParams  SFunctionDeploymentMode=off  EnableBusSupport=off  mask(FTM_s32k_pwm_config_block){ftmModule=0, ftmMode=Edge-Aligned PWM, ftmSourceClock=80 MHz, swcontrol_enable=off, chan0En=on, chan0Type=Complementary, chan2En=off, chan2Type=Independent, chan4En=off, chan4Type=Independent, chan6En=off, chan6Type=Independent, ftmPwmUnits=Hz, outFrequency=1000, ftmPeriod=20000, ftmPrescaler=Divide by 4, deadtimeUnits=Nanoseconds, deadtimeNs=0, deadtimeTicks=0, deadtimePrescaler=Divide by 1, dutyCycleCh0=0.25, dutyCycleCh1=0.25, dutyCycleCh2=0.25, dutyCycleCh3=0.25, dutyCycleCh4=0.25, dutyCycleCh5=0.25, dutyCycleCh6=0.25, dutyCycleCh7=0.25, dutyCycleSim=on, startAfterInit=on, showAdvOpt=on, pinFtmCh0=PTD15: [FTM0_CH0 | FTM Channel], pinFtmCh1=None, pinPolCh0=Active Low, pinPolCh1=Active Low, outputComplem0=Main duplicated, outputLevel0=Low, outputLevel1=Low, pinFtmCh2=PTC2: [FTM0_CH2 | FTM Channel], pinFtmCh3=None, pinPolCh2=Active Low, pinPolCh3=Active Low, outputComplem2=Main duplicated, outputLevel2=Low, outputLevel3=Low, pinFtmCh4=PTB4: [FTM0_CH4 | FTM Channel], pinFtmCh5=None, pinPolCh4=Active Low, pinPolCh5=Active Low, outputComplem4=Main duplicated, outputLevel4=Low, outputLevel5=Low, pinFtmCh6=PTD15: [FTM0_CH0 | FTM Channel], pinFtmCh7=None, pinPolCh6=Active Low, pinPolCh7=Active Low, outputComplem6=Main duplicated, outputLevel6=Low, outputLevel7=Low, initTrigger=off, chTrigger0=off, chTrigger1=off, chTrigger2=off, chTrigger3=off, chTrigger4=off, chTrigger5=off, chTrigger6=off, chTrigger7=off, mcuTargetUpdate=on, pwmSyncTrg=Software trigger, pwmSyncHwRouting=TRGMUX_FTM7, pwmSyncTrg0=off, pwmSyncTrg1=off, pwmSyncTrg2=off, pwmSyncAutoClear=on, pwmSyncMinLoad=on, pwmSyncMaxLoad=on, pwmSyncInvert=System Clock, pwmSyncOutControl=System Clock, pwmSyncOutMask=System Clock, pwmSyncCounterInitial=System Clock, pwmSyncPoints=Update now, reloadEnable=off, reloadPriority=15, reloadHalfCycle=off, reloadHCR=0, reloadFrequency=0, chnMatch0=off, chnMatch1=off, chnMatch2=off, chnMatch3=off, chnMatch4=off, chnMatch5=off, chnMatch6=off, chnMatch7=off, pwmFaultProtection=off, pwmFaultInterrupt=off, pwmFaultClearing=Fault control disabled, pwmFaultPinState=Safe Value, pwmFaultFilterValue=0, pwmFaultPriority=15, fault_disen_0=off, fault_filter_0=off, fault_polarity_0=Active High, fault_disen_1=off, fault_filter_1=off, fault_polarity_1=Active high, fault_disen_2=off, fault_filter_2=off, fault_polarity_2=Active high, fault_disen_3=off, fault_filter_3=off, fault_polarity_3=Active high, fault_pin_0=None, fault_pin_1=None, fault_pin_2=None, fault_pin_3=None}
      mask prompts: ftmModule "Module"; ftmMode "Mode"; ftmSourceClock "FTM Source Clock"; swcontrol_enable "FTM Software Output Control"; chan0En "PWM Pair 0 - 1 (A)"; chan2En "PWM Pair 2 - 3 (B)"; chan4En "PWM Pair 4 - 5 (C)"; chan6En "PWM Pair 6 - 7 (D)"; ftmPwmUnits "PWM Period expressed in units of:"; outFrequency "PWM Output Frequency (Hz)"; ftmPeriod "PWM Period Value (Ticks)"; ftmPrescaler "PWM Prescaler"; deadtimeUnits "Deadtime expressed in units of:"; deadtimeNs "Deadtime (ns)"; deadtimeTicks "Deadtime (Ticks)"; deadtimePrescaler "Deadtime Prescaler"; dutyCycleCh0 "Initial Duty Cycle Ch 0 (0 - 1.0)"; dutyCycleCh1 "Initial Duty Cycle Ch 1 (0 - 1.0)"; dutyCycleCh2 "Initial Duty Cycle Ch 2 (0 - 1.0)"; dutyCycleCh3 "Initial Duty Cycle Ch 3 (0 - 1.0)"; dutyCycleCh4 "Initial Duty Cycle Ch 4 (0 - 1.0)"; dutyCycleCh5 "Initial Duty Cycle Ch 5 (0 - 1.0)"; dutyCycleCh6 "Initial Duty Cycle Ch 6 (0 - 1.0)"; dutyCycleCh7 "Initial Duty Cycle Ch 7 (0 - 1.0)"; dutyCycleSim "Duty Cycle Simulation output"; startAfterInit "Start PWM signals generation immediately after initialization"; showAdvOpt "Show advanced options"; pinFtmCh0 "Ch[0] output pin"; pinFtmCh1 "Ch[1] output pin"; pinPolCh0 "Ch[0] polarity"; pinPolCh1 "Ch[1] polarity"; outputComplem0 "Ch[1] polarity"; outputLevel0 "Ch[0] safe state"; outputLevel1 "Ch[1] safe state"; pinFtmCh2 "Ch[2] output pin"; pinFtmCh3 "Ch[3] output pin"; pinPolCh2 "Ch[2] polarity"; pinPolCh3 "Ch[3] polarity"; outputComplem2 "Ch[3] polarity"; outputLevel2 "Ch[2] safe state"; outputLevel3 "Ch[3] safe state"; pinFtmCh4 "Ch[4] output pin"; pinFtmCh5 "Ch[5] output pin"; pinPolCh4 "Ch[4] polarity"; pinPolCh5 "Ch[5] polarity"; outputComplem4 "Ch[5] polarity"; outputLevel4 "Ch[4] safe state"; outputLevel5 "Ch[5] safe state"; pinFtmCh6 "Ch[6] output pin"; pinFtmCh7 "Ch[7] output pin"; pinPolCh6 "Ch[6] polarity"; pinPolCh7 "Ch[7] polarity"; outputComplem6 "Ch[7] polarity"; outputLevel6 "Ch[6] safe state"; outputLevel7 "Ch[7] safe state"; initTrigger "Initialization Trigger"; chTrigger0 "Ch[0] Trigger"; chTrigger1 "Ch[1] Trigger"; chTrigger2 "Ch[2] Trigger"; chTrigger3 "Ch[3] Trigger"; chTrigger4 "Ch[4] Trigger"; chTrigger5 "Ch[5] Trigger"; chTrigger6 "Ch[6] Trigger"; chTrigger7 "Ch[7] Trigger"; mcuTargetUpdate "Mcu target update"; pwmSyncTrg "PWM synchronization"; pwmSyncHwRouting "HW sync routing"; pwmSyncTrg0 "Hardware trigger 0"; pwmSyncTrg1 "Hardware trigger 1"; pwmSyncTrg2 "Hardware trigger 2"; pwmSyncAutoClear "Auto Clear Trigger"; pwmSyncMinLoad "Minimum Loading Point Enable"; pwmSyncMaxLoad "Maximum Loading Point Enable"; pwmSyncInvert "Inverting Control Synchronization"; pwmSyncOutControl "Software Output Control Synchronization"; pwmSyncOutMask "Output Mask Synchronization"; pwmSyncCounterInitial "Counter Initial Synchronization"; pwmSyncPoints "Synchronization Points"; reloadEnable "Enable Reload Interrupt"; reloadPriority "Reload Interrupt Priority"; reloadHalfCycle "Half-cycle reload"; reloadHCR "Half Cycle Register (HCR)"; reloadFrequency "Frequency of the Reload Opportunities"; chnMatch0 "Channel 0 match is included as a reload opportunity"; chnMatch1 "Channel 1 match is included as a reload opportunity"; chnMatch2 "Channel 2 match is included as a reload opportunity"; chnMatch3 "Channel 3 match is included as a reload opportunity"; chnMatch4 "Channel 4 match is included as a reload opportunity"; chnMatch5 "Channel 5 match is included as a reload opportunity"; chnMatch6 "Channel 6 match is included as a reload opportunity"; chnMatch7 "Channel 7 match is included as a reload opportunity"; pwmFaultProtection "Enable Fault Protection"; pwmFaultInterrupt "Enable Fault Interrupt"; pwmFaultClearing "Automatic clearing"; pwmFaultPinState "PWM Output-pin State on Fault"; pwmFaultFilterValue "Fault Filter Value"; pwmFaultPriority "Fault Interrupt Priority"; fault_disen_0 "Channel 0"; fault_filter_0 "Filter enabled"; fault_polarity_0 "Polarity"; fault_disen_1 "Channel 1"; fault_filter_1 "Filter enabled"; fault_polarity_1 "Polarity"; fault_disen_2 "Channel 2"; fault_filter_2 "Filter enabled"; fault_polarity_2 "Polarity"; fault_disen_3 "Channel 3"; fault_filter_3 "Filter enabled"; fault_polarity_3 "Polarity"; fault_pin_0 "Fault 0 input pin"; fault_pin_1 "Fault 1 input pin"; fault_pin_2 "Fault 2 input pin"; fault_pin_3 "Fault 3 input pin"
      mask help: FTM Pulse Width Modulation Configuration Block which enables PWM signals on each FTM module in Edge/Center-Aligned/Combined mode with Deadtime, Syncronization points and Fault management.
      mask init:
      | funcParams = mbd_s32k_ftm_pwm_config_make_params(gcb);
      | 
      | mbd_s32k_isr_priority_cbk(gcb, 'reloadPriority');
      | mbd_s32k_isr_priority_cbk(gcb, 'pwmFaultPriority');
      | 
      | [labels, maskStr] = mbd_s32k_ftm_pwm_config_init(gcb);
      | set_param(gcb, 'MaskDisplay', labels);
      settings: NameChangeFcn=mbd_s32k_name_check(gcb);
      mask Help: web(fullfile(mbd_s32k_block_help, 'ftm', 'ftm_pwm_config_block.html'));
      mask TypeOptions ftmModule: 0 | 1 | 2 | 3 | 4 | 5 | 6 | 7
      mask Callback ftmModule:
      | mbd_s32k_ftm_display_modules(gcb);
      | 
      | mbd_s32k_ftm_pwm_config_cbk(gcb, 'ftm_change_modules');
      | mbd_s32k_ftm_pwm_config_cbk(gcb, 'ftm_show_pins');
      | mbd_s32k_ftm_pwm_config_cbk(gcb, 'ftm_fault_pins');
      | mbd_s32k_ftm_pwm_config_cbk(gcb, 'ftm_pwm_signals');
      mask TypeOptions ftmMode: Edge-Aligned PWM | Center-Aligned PWM | Combine mode PWM
      mask Callback ftmMode:
      | mbd_s32k_ftm_pwm_config_cbk(gcb, 'ftm_set_mode');
      | mbd_s32k_ftm_pwm_config_cbk(gcb, 'ftm_show_pins');
      mask Callback swcontrol_enable: mbd_s32k_ftm_pwm_config_cbk(gcb, 'ftm_sw_control');
      mask Callback chan0En: mbd_s32k_ftm_pwm_config_cbk(gcb, 'ftm_show_pins');
      mask TypeOptions chan0Type: Independent | Complementary
      mask Callback chan0Type: mbd_s32k_ftm_pwm_config_cbk(gcb, 'ftm_show_pins');
      mask Callback chan2En: mbd_s32k_ftm_pwm_config_cbk(gcb, 'ftm_show_pins');
      mask TypeOptions chan2Type: Independent | Complementary
      mask Callback chan2Type: mbd_s32k_ftm_pwm_config_cbk(gcb, 'ftm_show_pins');
      mask Callback chan4En: mbd_s32k_ftm_pwm_config_cbk(gcb, 'ftm_show_pins');
      mask TypeOptions chan4Type: Independent | Complementary
      mask Callback chan4Type: mbd_s32k_ftm_pwm_config_cbk(gcb, 'ftm_show_pins');
      mask Callback chan6En: mbd_s32k_ftm_pwm_config_cbk(gcb, 'ftm_show_pins');
      mask TypeOptions chan6Type: Independent | Complementary
      mask Callback chan6Type: mbd_s32k_ftm_pwm_config_cbk(gcb, 'ftm_show_pins');
      mask TypeOptions ftmPwmUnits: Hz | Ticks
      mask Callback ftmPwmUnits:
      | mbd_s32k_ftm_pwm_config_cbk(gcb, 'ftm_show_frequency');
      | mbd_s32k_ftm_pwm_config_cbk(gcb, 'ftm_set_frequency');
      mask Callback outFrequency: mbd_s32k_ftm_pwm_config_cbk(gcb, 'ftm_set_frequency');
      mask Callback ftmPeriod: mbd_s32k_ftm_pwm_config_cbk(gcb, 'ftm_set_frequency');
      mask TypeOptions ftmPrescaler: Divide by 1 | Divide by 2 | Divide by 4 | Divide by 8 | Divide by 16 | Divide by 32 | Divide by 64 | Divide by 128
      mask Callback ftmPrescaler: mbd_s32k_ftm_pwm_config_cbk(gcb, 'ftm_set_frequency');
      mask TypeOptions deadtimeUnits: Ticks | Nanoseconds
      mask Callback deadtimeUnits:
      | mbd_s32k_ftm_pwm_config_cbk(gcb, 'ftm_show_deadtime');
      | mbd_s32k_ftm_pwm_config_cbk(gcb, 'ftm_set_deadtime');
      mask Callback deadtimeNs: mbd_s32k_ftm_pwm_config_cbk(gcb, 'ftm_set_deadtime');
      mask Callback deadtimeTicks: mbd_s32k_ftm_pwm_config_cbk(gcb, 'ftm_set_deadtime');
      mask TypeOptions deadtimePrescaler: Divide by 1 | Divide by 4 | Divide by 16
      mask Callback deadtimePrescaler: mbd_s32k_ftm_pwm_config_cbk(gcb, 'ftm_set_deadtime');
      mask Callback dutyCycleCh0: mbd_s32k_ftm_pwm_config_cbk(gcb, 'ftm_check_duty_cycle');
      mask Callback dutyCycleCh1: mbd_s32k_ftm_pwm_config_cbk(gcb, 'ftm_check_duty_cycle');
      mask Callback dutyCycleCh2: mbd_s32k_ftm_pwm_config_cbk(gcb, 'ftm_check_duty_cycle');
      mask Callback dutyCycleCh3: mbd_s32k_ftm_pwm_config_cbk(gcb, 'ftm_check_duty_cycle');
      mask Callback dutyCycleCh4: mbd_s32k_ftm_pwm_config_cbk(gcb, 'ftm_check_duty_cycle');
      mask Callback dutyCycleCh5: mbd_s32k_ftm_pwm_config_cbk(gcb, 'ftm_check_duty_cycle');
      mask Callback dutyCycleCh6: mbd_s32k_ftm_pwm_config_cbk(gcb, 'ftm_check_duty_cycle');
      mask Callback dutyCycleCh7: mbd_s32k_ftm_pwm_config_cbk(gcb, 'ftm_check_duty_cycle');
      mask Callback showAdvOpt: mbd_s32k_ftm_pwm_config_cbk(gcb, 'ftm_show_adv_opts');
      mask TypeOptions pinFtmCh0: PTD15: [FTM0_CH0 | FTM Channel] | PTB13: [FTM0_CH1 | FTM Channel] | PTC1: [FTM0_CH1 | FTM Channel] | PTD16: [FTM0_CH1 | FTM Channel] | PTC2: [FTM0_CH2 | FTM Channel] | PTD0: [FTM0_CH2 | FTM Channel] | PTC3: [FTM0_CH3 | FTM Channel] | PTD1: [FTM0_CH3 | FTM Channel] | PTB4: [FTM0_CH4 | FTM Channel] | PTB5: [FTM0_CH5 | FTM Channel] | PTE8: [FTM0_CH6 | FTM Channel] | PTE9: [FTM0_CH7 | FTM Channel] | PTB2: [FTM1_CH0 | FTM Channel] | PTC4: [FTM1_CH0 | FTM Channel] | PTA1: [FTM1_CH1 | FTM Channel] | PTB3: [FTM1_CH1 | FTM Channel] | PTC14: [FTM1_CH2 | FTM Channel] | PTC15: [FTM1_CH3 | FTM Channel] | PTA10: [FTM1_CH4 | FTM Channel] | PTA11: [FTM1_CH5 | FTM Channel] | PTA12: [FTM1_CH6 | FTM Channel] | PTA13: [FTM1_CH7 | FTM Channel] | PTC1: [FTM1_CH7 | FTM Channel] | PTD15: [FTM0_CH0 | FTM Channel] | PTB13: [FTM0_CH1 | FTM Channel] | PTC1: [FTM0_CH1 | FTM Channel] | PTD16: [FTM0_CH1 | FTM Channel] | PTC2: [FTM0_CH2 | FTM Channel] | PTD0: [FTM0_CH2 | FTM Channel] | PTC3: [FTM0_CH3 | FTM Channel] | PTD1: [FTM0_CH3 | FTM Channel] | PTB4: [FTM0_CH4 | FTM Channel] | PTB5: [FTM0_CH5 | FTM Channel] | PTE8: [FTM0_CH6 | FTM Channel] | PTE9: [FTM0_CH7 | FTM Channel] | PTB2: [FTM1_CH0 | FTM Channel] | PTC4: [FTM1_CH0 | FTM Channel] | PTA1: [FTM1_CH1 | FTM Channel] | PTB3: [FTM1_CH1 | FTM Channel] | PTC14: [FTM1_CH2 | FTM Channel] | PTC15: [FTM1_CH3 | FTM Channel] | PTA10: [FTM1_CH4 | FTM Channel] | PTA11: [FTM1_CH5 | FTM Channel] | PTA12: [FTM1_CH6 | FTM Channel] | PTA13: [FTM1_CH7 | FTM Channel] | PTC1: [FTM1_CH7 | FTM Channel] | PTD15: [FTM0_CH0 | FTM Channel] | PTB13: [FTM0_CH1 | FTM Channel] | PTC1: [FTM0_CH1 | FTM Channel] | PTD16: [FTM0_CH1 | FTM Channel] | PTC2: [FTM0_CH2 | FTM Channel] | PTD0: [FTM0_CH2 | FTM Channel] | PTC3: [FTM0_CH3 | FTM Channel] | PTD1: [FTM0_CH3 | FTM Channel] | PTB4: [FTM0_CH4 | FTM Channel] | PTB5: [FTM0_CH5 | FTM Channel] | PTE8: [FTM0_CH6 | FTM Channel] | PTE9: [FTM0_CH7 | FTM Channel] | PTB2: [FTM1_CH0 | FTM Channel] | PTC4: [FTM1_CH0 | FTM Channel] | PTA1: [FTM1_CH1 | FTM Channel] | PTB3: [FTM1_CH1 | FTM Channel] | PTC14: [FTM1_CH2 | FTM Channel] | PTC15: [FTM1_CH3 | FTM Channel] | PTA10: [FTM1_CH4 | FTM Channel] | PTA11: [FTM1_CH5 | FTM Channel] | PTA12: [FTM1_CH6 | FTM Channel] | PTA13: [FTM1_CH7 | FTM Channel] | PTC1: [FTM1_CH7 | FTM Channel] | PTC5: [FTM2_CH0 | FTM Channel] | PTD0: [FTM2_CH0 | FTM Channel] | PTD10: [FTM2_CH0 | FTM Channel] | PTA0: [FTM2_CH1 | FTM Channel] | PTD1: [FTM2_CH1 | FTM Channel] | PTD11: [FTM2_CH1 | FTM Channel] | PTD12: [FTM2_CH2 | FTM Channel] | PTE4: [FTM2_CH2 | FTM Channel] | PTD5: [FTM2_CH3 | FTM Channel] | PTE5: [FTM2_CH3 | FTM Channel] | PTD13: [FTM2_CH4 | FTM Channel] | PTE10: [FTM2_CH4 | FTM Channel] | PTD14: [FTM2_CH5 | FTM Channel] | PTE11: [FTM2_CH5 | FTM Channel] | PTC12: [FTM2_CH6 | FTM Channel] | PTE15: [FTM2_CH6 | FTM Channel] | PTC13: [FTM2_CH7 | FTM Channel] | PTE16: [FTM2_CH7 | FTM Channel] | PTA2: [FTM3_CH0 | FTM Channel] | PTB8: [FTM3_CH0 | FTM Channel] | PTA3: [FTM3_CH1 | FTM Channel] | PTB9: [FTM3_CH1 | FTM Channel] | PTB10: [FTM3_CH2 | FTM Channel] | PTC6: [FTM3_CH2 | FTM Channel] | PTB11: [FTM3_CH3 | FTM Channel] | PTC7: [FTM3_CH3 | FTM Channel] | PTC10: [FTM3_CH4 | FTM Channel] | PTD2: [FTM3_CH4 | FTM Channel] | PTC11: [FTM3_CH5 | FTM Channel] | PTD3: [FTM3_CH5 | FTM Channel] | PTC12: [FTM3_CH6 | FTM Channel] | PTE2: [FTM3_CH6 | FTM Channel] | PTC13: [FTM3_CH7 | FTM Channel] | PTE6: [FTM3_CH7 | FTM Channel] | PTD15: [FTM0_CH0 | FTM Channel] | PTB13: [FTM0_CH1 | FTM Channel] | PTC1: [FTM0_CH1 | FTM Channel] | PTD16: [FTM0_CH1 | FTM Channel] | PTC2: [FTM0_CH2 | FTM Channel] | PTD0: [FTM0_CH2 | FTM Channel] | PTC3: [FTM0_CH3 | FTM Channel] | PTD1: [FTM0_CH3 | FTM Channel] | PTB4: [FTM0_CH4 | FTM Channel] | PTB5: [FTM0_CH5 | FTM Channel] | PTE8: [FTM0_CH6 | FTM Channel] | PTE9: [FTM0_CH7 | FTM Channel] | PTB2: [FTM1_CH0 | FTM Channel] | PTC4: [FTM1_CH0 | FTM Channel] | PTA1: [FTM1_CH1 | FTM Channel] | PTB3: [FTM1_CH1 | FTM Channel] | PTC14: [FTM1_CH2 | FTM Channel] | PTC15: [FTM1_CH3 | FTM Channel] | PTA10: [FTM1_CH4 | FTM Channel] | PTA11: [FTM1_CH5 | FTM Channel] | PTA12: [FTM1_CH6 | FTM Channel] | PTA13: [FTM1_CH7 | FTM Channel] | PTC1: [FTM1_CH7 | FTM Channel] | PTC5: [FTM2_CH0 | FTM Channel] | PTD0: [FTM2_CH0 | FTM Channel] | PTD10: [FTM2_CH0 | FTM Channel] | PTA0: [FTM2_CH1 | FTM Channel] | PTD1: [FTM2_CH1 | FTM Channel] | PTD11: [FTM2_CH1 | FTM Channel] | PTD12: [FTM2_CH2 | FTM Channel] | PTE4: [FTM2_CH2 | FTM Channel] | PTD5: [FTM2_CH3 | FTM Channel] | PTE5: [FTM2_CH3 | FTM Channel] | PTD13: [FTM2_CH4 | FTM Channel] | PTE10: [FTM2_CH4 | FTM Channel] | PTD14: [FTM2_CH5 | FTM Channel] | PTE11: [FTM2_CH5 | FTM Channel] | PTC12: [FTM2_CH6 | FTM Channel] | PTE15: [FTM2_CH6 | FTM Channel] | PTC13: [FTM2_CH7 | FTM Channel] | PTE16: [FTM2_CH7 | FTM Channel] | PTA2: [FTM3_CH0 | FTM Channel] | PTB8: [FTM3_CH0 | FTM Channel] | PTA3: [FTM3_CH1 | FTM Channel] | PTB9: [FTM3_CH1 | FTM Channel] | PTB10: [FTM3_CH2 | FTM Channel] | PTC6: [FTM3_CH2 | FTM Channel] | PTB11: [FTM3_CH3 | FTM Channel] | PTC7: [FTM3_CH3 | FTM Channel] | PTC10: [FTM3_CH4 | FTM Channel] | PTD2: [FTM3_CH4 | FTM Channel] | PTC11: [FTM3_CH5 | FTM Channel] | PTD3: [FTM3_CH5 | FTM Channel] | PTC12: [FTM3_CH6 | FTM Channel] | PTE2: [FTM3_CH6 | FTM Channel] | PTC13: [FTM3_CH7 | FTM Channel] | PTE6: [FTM3_CH7 | FTM Channel] | PTD15: [FTM0_CH0 | FTM Channel] | PTB13: [FTM0_CH1 | FTM Channel] | PTC1: [FTM0_CH1 | FTM Channel] | PTD16: [FTM0_CH1 | FTM Channel] | PTC2: [FTM0_CH2 | FTM Channel] | PTD0: [FTM0_CH2 | FTM Channel] | PTC3: [FTM0_CH3 | FTM Channel] | PTD1: [FTM0_CH3 | FTM Channel] | PTB4: [FTM0_CH4 | FTM Channel] | PTB5: [FTM0_CH5 | FTM Channel] | PTE8: [FTM0_CH6 | FTM Channel] | PTE9: [FTM0_CH7 | FTM Channel] | PTB2: [FTM1_CH0 | FTM Channel] | PTC4: [FTM1_CH0 | FTM Channel] | PTA1: [FTM1_CH1 | FTM Channel] | PTB3: [FTM1_CH1 | FTM Channel] | PTC14: [FTM1_CH2 | FTM Channel] | PTC15: [FTM1_CH3 | FTM Channel] | PTA10: [FTM1_CH4 | FTM Channel] | PTA11: [FTM1_CH5 | FTM Channel] | PTA12: [FTM1_CH6 | FTM Channel] | PTA13: [FTM1_CH7 | FTM Channel] | PTC1: [FTM1_CH7 | FTM Channel] | PTC5: [FTM2_CH0 | FTM Channel] | PTD0: [FTM2_CH0 | FTM Channel] | PTD10: [FTM2_CH0 | FTM Channel] | PTA0: [FTM2_CH1 | FTM Channel] | PTD1: [FTM2_CH1 | FTM Channel] | PTD11: [FTM2_CH1 | FTM Channel] | PTD12: [FTM2_CH2 | FTM Channel] | PTE4: [FTM2_CH2 | FTM Channel] | PTD5: [FTM2_CH3 | FTM Channel] | PTE5: [FTM2_CH3 | FTM Channel] | PTD13: [FTM2_CH4 | FTM Channel] | PTE10: [FTM2_CH4 | FTM Channel] | PTD14: [FTM2_CH5 | FTM Channel] | PTE11: [FTM2_CH5 | FTM Channel] | PTC12: [FTM2_CH6 | FTM Channel] | PTE15: [FTM2_CH6 | FTM Channel] | PTC13: [FTM2_CH7 | FTM Channel] | PTE16: [FTM2_CH7 | FTM Channel] | PTA2: [FTM3_CH0 | FTM Channel] | PTB8: [FTM3_CH0 | FTM Channel] | PTA3: [FTM3_CH1 | FTM Channel] | PTB9: [FTM3_CH1 | FTM Channel] | PTB10: [FTM3_CH2 | FTM Channel] | PTC6: [FTM3_CH2 | FTM Channel] | PTB11: [FTM3_CH3 | FTM Channel] | PTC7: [FTM3_CH3 | FTM Channel] | PTC10: [FTM3_CH4 | FTM Channel] | PTD2: [FTM3_CH4 | FTM Channel] | PTC11: [FTM3_CH5 | FTM Channel] | PTD3: [FTM3_CH5 | FTM Channel] | PTC12: [FTM3_CH6 | FTM Channel] | PTE2: [FTM3_CH6 | FTM Channel] | PTC13: [FTM3_CH7 | FTM Channel] | PTE6: [FTM3_CH7 | FTM Channel] | PTE20: [FTM4_CH0 | FTM Channel] | PTE21: [FTM4_CH1 | FTM Channel] | PTC11: [FTM4_CH2 | FTM Channel] | PTE22: [FTM4_CH2 | FTM Channel] | PTE23: [FTM4_CH3 | FTM Channel] | PTC27: [FTM4_CH4 | FTM Channel] | PTE24: [FTM4_CH4 | FTM Channel] | PTB1: [FTM4_CH5 | FTM Channel] | PTE13: [FTM4_CH5 | FTM Channel] | PTE25: [FTM4_CH5 | FTM Channel] | PTB0: [FTM4_CH6 | FTM Channel] | PTC28: [FTM4_CH7 | FTM Channel] | PTA25: [FTM5_CH0 | FTM Channel] | PTC9: [FTM5_CH0 | FTM Channel] | PTA26: [FTM5_CH1 | FTM Channel] | PTC8: [FTM5_CH1 | FTM Channel] | PTA27: [FTM5_CH2 | FTM Channel] | PTC29: [FTM5_CH2 | FTM Channel] | PTA7: [FTM5_CH3 | FTM Channel] | PTA28: [FTM5_CH3 | FTM Channel] | PTA29: [FTM5_CH4 | FTM Channel] | PTC30: [FTM5_CH4 | FTM Channel] | PTA6: [FTM5_CH5 | FTM Channel] | PTA30: [FTM5_CH5 | FTM Channel] | PTA31: [FTM5_CH6 | FTM Channel] | PTC31: [FTM5_CH6 | FTM Channel] | PTB18: [FTM5_CH7 | FTM Channel] | PTD18: [FTM5_CH7 | FTM Channel] | PTD15: [FTM0_CH0 | FTM Channel] | PTB13: [FTM0_CH1 | FTM Channel] | PTC1: [FTM0_CH1 | FTM Channel] | PTD16: [FTM0_CH1 | FTM Channel] | PTC2: [FTM0_CH2 | FTM Channel] | PTD0: [FTM0_CH2 | FTM Channel] | PTC3: [FTM0_CH3 | FTM Channel] | PTD1: [FTM0_CH3 | FTM Channel] | PTB4: [FTM0_CH4 | FTM Channel] | PTB5: [FTM0_CH5 | FTM Channel] | PTE8: [FTM0_CH6 | FTM Channel] | PTE9: [FTM0_CH7 | FTM Channel] | PTB2: [FTM1_CH0 | FTM Channel] | PTC4: [FTM1_CH0 | FTM Channel] | PTA1: [FTM1_CH1 | FTM Channel] | PTB3: [FTM1_CH1 | FTM Channel] | PTC14: [FTM1_CH2 | FTM Channel] | PTC15: [FTM1_CH3 | FTM Channel] | PTA10: [FTM1_CH4 | FTM Channel] | PTA11: [FTM1_CH5 | FTM Channel] | PTA12: [FTM1_CH6 | FTM Channel] | PTA13: [FTM1_CH7 | FTM Channel] | PTC1: [FTM1_CH7 | FTM Channel] | PTC5: [FTM2_CH0 | FTM Channel] | PTD0: [FTM2_CH0 | FTM Channel] | PTD10: [FTM2_CH0 | FTM Channel] | PTA0: [FTM2_CH1 | FTM Channel] | PTD1: [FTM2_CH1 | FTM Channel] | PTD11: [FTM2_CH1 | FTM Channel] | PTD12: [FTM2_CH2 | FTM Channel] | PTE4: [FTM2_CH2 | FTM Channel] | PTD5: [FTM2_CH3 | FTM Channel] | PTE5: [FTM2_CH3 | FTM Channel] | PTD13: [FTM2_CH4 | FTM Channel] | PTE10: [FTM2_CH4 | FTM Channel] | PTD14: [FTM2_CH5 | FTM Channel] | PTE11: [FTM2_CH5 | FTM Channel] | PTC12: [FTM2_CH6 | FTM Channel] | PTE15: [FTM2_CH6 | FTM Channel] | PTC13: [FTM2_CH7 | FTM Channel] | PTE16: [FTM2_CH7 | FTM Channel] | PTA2: [FTM3_CH0 | FTM Channel] | PTB8: [FTM3_CH0 | FTM Channel] | PTA3: [FTM3_CH1 | FTM Channel] | PTB9: [FTM3_CH1 | FTM Channel] | PTB10: [FTM3_CH2 | FTM Channel] | PTC6: [FTM3_CH2 | FTM Channel] | PTB11: [FTM3_CH3 | FTM Channel] | PTC7: [FTM3_CH3 | FTM Channel] | PTC10: [FTM3_CH4 | FTM Channel] | PTD2: [FTM3_CH4 | FTM Channel] | PTC11: [FTM3_CH5 | FTM Channel] | PTD3: [FTM3_CH5 | FTM Channel] | PTC12: [FTM3_CH6 | FTM Channel] | PTE2: [FTM3_CH6 | FTM Channel] | PTC13: [FTM3_CH7 | FTM Channel] | PTE6: [FTM3_CH7 | FTM Channel] | PTE20: [FTM4_CH0 | FTM Channel] | PTE21: [FTM4_CH1 | FTM Channel] | PTC11: [FTM4_CH2 | FTM Channel] | PTE22: [FTM4_CH2 | FTM Channel] | PTE23: [FTM4_CH3 | FTM Channel] | PTC27: [FTM4_CH4 | FTM Channel] | PTE24: [FTM4_CH4 | FTM Channel] | PTB1: [FTM4_CH5 | FTM Channel] | PTE13: [FTM4_CH5 | FTM Channel] | PTE25: [FTM4_CH5 | FTM Channel] | PTB0: [FTM4_CH6 | FTM Channel] | PTC28: [FTM4_CH7 | FTM Channel] | PTA25: [FTM5_CH0 | FTM Channel] | PTC9: [FTM5_CH0 | FTM Channel] | PTA26: [FTM5_CH1 | FTM Channel] | PTC8: [FTM5_CH1 | FTM Channel] | PTA27: [FTM5_CH2 | FTM Channel] | PTC29: [FTM5_CH2 | FTM Channel] | PTA7: [FTM5_CH3 | FTM Channel] | PTA28: [FTM5_CH3 | FTM Channel] | PTA29: [FTM5_CH4 | FTM Channel] | PTC30: [FTM5_CH4 | FTM Channel] | PTA6: [FTM5_CH5 | FTM Channel] | PTA30: [FTM5_CH5 | FTM Channel] | PTA31: [FTM5_CH6 | FTM Channel] | PTC31: [FTM5_CH6 | FTM Channel] | PTB18: [FTM5_CH7 | FTM Channel] | PTD18: [FTM5_CH7 | FTM Channel] | PTA18: [FTM6_CH0 | FTM Channel] | PTB20: [FTM6_CH0 | FTM Channel] | PTD19: [FTM6_CH0 | FTM Channel] | PTB21: [FTM6_CH1 | FTM Channel] | PTD20: [FTM6_CH1 | FTM Channel] | PTB22: [FTM6_CH2 | FTM Channel] | PTD21: [FTM6_CH2 | FTM Channel] | PTB23: [FTM6_CH3 | FTM Channel] | PTD22: [FTM6_CH3 | FTM Channel] | PTB24: [FTM6_CH4 | FTM Channel] | PTD23: [FTM6_CH4 | FTM Channel] | PTB25: [FTM6_CH5 | FTM Channel] | PTD24: [FTM6_CH5 | FTM Channel] | PTB26: [FTM6_CH6 | FTM Channel] | PTD25: [FTM6_CH6 | FTM Channel] | PTB27: [FTM6_CH7 | FTM Channel] | PTD26: [FTM6_CH7 | FTM Channel] | PTB28: [FTM7_CH0 | FTM Channel] | PTD27: [FTM7_CH0 | FTM Channel] | PTB29: [FTM7_CH1 | FTM Channel] | PTD28: [FTM7_CH1 | FTM Channel] | PTB30: [FTM7_CH2 | FTM Channel] | PTD29: [FTM7_CH2 | FTM Channel] | PTB31: [FTM7_CH3 | FTM Channel] | PTD30: [FTM7_CH3 | FTM Channel] | PTC18: [FTM7_CH4 | FTM Channel] | PTD31: [FTM7_CH4 | FTM Channel] | PTC19: [FTM7_CH5 | FTM Channel] | PTE17: [FTM7_CH5 | FTM Channel] | PTC20: [FTM7_CH6 | FTM Channel] | PTE18: [FTM7_CH6 | FTM Channel] | PTC21: [FTM7_CH7 | FTM Channel] | PTE19: [FTM7_CH7 | FTM Channel]
      mask TypeOptions pinFtmCh1: None | PTD15: [FTM0_CH0 | FTM Channel] | PTB13: [FTM0_CH1 | FTM Channel] | PTC1: [FTM0_CH1 | FTM Channel] | PTD16: [FTM0_CH1 | FTM Channel] | PTC2: [FTM0_CH2 | FTM Channel] | PTD0: [FTM0_CH2 | FTM Channel] | PTC3: [FTM0_CH3 | FTM Channel] | PTD1: [FTM0_CH3 | FTM Channel] | PTB4: [FTM0_CH4 | FTM Channel] | PTB5: [FTM0_CH5 | FTM Channel] | PTE8: [FTM0_CH6 | FTM Channel] | PTE9: [FTM0_CH7 | FTM Channel] | PTB2: [FTM1_CH0 | FTM Channel] | PTC4: [FTM1_CH0 | FTM Channel] | PTA1: [FTM1_CH1 | FTM Channel] | PTB3: [FTM1_CH1 | FTM Channel] | PTC14: [FTM1_CH2 | FTM Channel] | PTC15: [FTM1_CH3 | FTM Channel] | PTA10: [FTM1_CH4 | FTM Channel] | PTA11: [FTM1_CH5 | FTM Channel] | PTA12: [FTM1_CH6 | FTM Channel] | PTA13: [FTM1_CH7 | FTM Channel] | PTC1: [FTM1_CH7 | FTM Channel] | PTD15: [FTM0_CH0 | FTM Channel] | PTB13: [FTM0_CH1 | FTM Channel] | PTC1: [FTM0_CH1 | FTM Channel] | PTD16: [FTM0_CH1 | FTM Channel] | PTC2: [FTM0_CH2 | FTM Channel] | PTD0: [FTM0_CH2 | FTM Channel] | PTC3: [FTM0_CH3 | FTM Channel] | PTD1: [FTM0_CH3 | FTM Channel] | PTB4: [FTM0_CH4 | FTM Channel] | PTB5: [FTM0_CH5 | FTM Channel] | PTE8: [FTM0_CH6 | FTM Channel] | PTE9: [FTM0_CH7 | FTM Channel] | PTB2: [FTM1_CH0 | FTM Channel] | PTC4: [FTM1_CH0 | FTM Channel] | PTA1: [FTM1_CH1 | FTM Channel] | PTB3: [FTM1_CH1 | FTM Channel] | PTC14: [FTM1_CH2 | FTM Channel] | PTC15: [FTM1_CH3 | FTM Channel] | PTA10: [FTM1_CH4 | FTM Channel] | PTA11: [FTM1_CH5 | FTM Channel] | PTA12: [FTM1_CH6 | FTM Channel] | PTA13: [FTM1_CH7 | FTM Channel] | PTC1: [FTM1_CH7 | FTM Channel] | PTD15: [FTM0_CH0 | FTM Channel] | PTB13: [FTM0_CH1 | FTM Channel] | PTC1: [FTM0_CH1 | FTM Channel] | PTD16: [FTM0_CH1 | FTM Channel] | PTC2: [FTM0_CH2 | FTM Channel] | PTD0: [FTM0_CH2 | FTM Channel] | PTC3: [FTM0_CH3 | FTM Channel] | PTD1: [FTM0_CH3 | FTM Channel] | PTB4: [FTM0_CH4 | FTM Channel] | PTB5: [FTM0_CH5 | FTM Channel] | PTE8: [FTM0_CH6 | FTM Channel] | PTE9: [FTM0_CH7 | FTM Channel] | PTB2: [FTM1_CH0 | FTM Channel] | PTC4: [FTM1_CH0 | FTM Channel] | PTA1: [FTM1_CH1 | FTM Channel] | PTB3: [FTM1_CH1 | FTM Channel] | PTC14: [FTM1_CH2 | FTM Channel] | PTC15: [FTM1_CH3 | FTM Channel] | PTA10: [FTM1_CH4 | FTM Channel] | PTA11: [FTM1_CH5 | FTM Channel] | PTA12: [FTM1_CH6 | FTM Channel] | PTA13: [FTM1_CH7 | FTM Channel] | PTC1: [FTM1_CH7 | FTM Channel] | PTC5: [FTM2_CH0 | FTM Channel] | PTD0: [FTM2_CH0 | FTM Channel] | PTD10: [FTM2_CH0 | FTM Channel] | PTA0: [FTM2_CH1 | FTM Channel] | PTD1: [FTM2_CH1 | FTM Channel] | PTD11: [FTM2_CH1 | FTM Channel] | PTD12: [FTM2_CH2 | FTM Channel] | PTE4: [FTM2_CH2 | FTM Channel] | PTD5: [FTM2_CH3 | FTM Channel] | PTE5: [FTM2_CH3 | FTM Channel] | PTD13: [FTM2_CH4 | FTM Channel] | PTE10: [FTM2_CH4 | FTM Channel] | PTD14: [FTM2_CH5 | FTM Channel] | PTE11: [FTM2_CH5 | FTM Channel] | PTC12: [FTM2_CH6 | FTM Channel] | PTE15: [FTM2_CH6 | FTM Channel] | PTC13: [FTM2_CH7 | FTM Channel] | PTE16: [FTM2_CH7 | FTM Channel] | PTA2: [FTM3_CH0 | FTM Channel] | PTB8: [FTM3_CH0 | FTM Channel] | PTA3: [FTM3_CH1 | FTM Channel] | PTB9: [FTM3_CH1 | FTM Channel] | PTB10: [FTM3_CH2 | FTM Channel] | PTC6: [FTM3_CH2 | FTM Channel] | PTB11: [FTM3_CH3 | FTM Channel] | PTC7: [FTM3_CH3 | FTM Channel] | PTC10: [FTM3_CH4 | FTM Channel] | PTD2: [FTM3_CH4 | FTM Channel] | PTC11: [FTM3_CH5 | FTM Channel] | PTD3: [FTM3_CH5 | FTM Channel] | PTC12: [FTM3_CH6 | FTM Channel] | PTE2: [FTM3_CH6 | FTM Channel] | PTC13: [FTM3_CH7 | FTM Channel] | PTE6: [FTM3_CH7 | FTM Channel] | PTD15: [FTM0_CH0 | FTM Channel] | PTB13: [FTM0_CH1 | FTM Channel] | PTC1: [FTM0_CH1 | FTM Channel] | PTD16: [FTM0_CH1 | FTM Channel] | PTC2: [FTM0_CH2 | FTM Channel] | PTD0: [FTM0_CH2 | FTM Channel] | PTC3: [FTM0_CH3 | FTM Channel] | PTD1: [FTM0_CH3 | FTM Channel] | PTB4: [FTM0_CH4 | FTM Channel] | PTB5: [FTM0_CH5 | FTM Channel] | PTE8: [FTM0_CH6 | FTM Channel] | PTE9: [FTM0_CH7 | FTM Channel] | PTB2: [FTM1_CH0 | FTM Channel] | PTC4: [FTM1_CH0 | FTM Channel] | PTA1: [FTM1_CH1 | FTM Channel] | PTB3: [FTM1_CH1 | FTM Channel] | PTC14: [FTM1_CH2 | FTM Channel] | PTC15: [FTM1_CH3 | FTM Channel] | PTA10: [FTM1_CH4 | FTM Channel] | PTA11: [FTM1_CH5 | FTM Channel] | PTA12: [FTM1_CH6 | FTM Channel] | PTA13: [FTM1_CH7 | FTM Channel] | PTC1: [FTM1_CH7 | FTM Channel] | PTC5: [FTM2_CH0 | FTM Channel] | PTD0: [FTM2_CH0 | FTM Channel] | PTD10: [FTM2_CH0 | FTM Channel] | PTA0: [FTM2_CH1 | FTM Channel] | PTD1: [FTM2_CH1 | FTM Channel] | PTD11: [FTM2_CH1 | FTM Channel] | PTD12: [FTM2_CH2 | FTM Channel] | PTE4: [FTM2_CH2 | FTM Channel] | PTD5: [FTM2_CH3 | FTM Channel] | PTE5: [FTM2_CH3 | FTM Channel] | PTD13: [FTM2_CH4 | FTM Channel] | PTE10: [FTM2_CH4 | FTM Channel] | PTD14: [FTM2_CH5 | FTM Channel] | PTE11: [FTM2_CH5 | FTM Channel] | PTC12: [FTM2_CH6 | FTM Channel] | PTE15: [FTM2_CH6 | FTM Channel] | PTC13: [FTM2_CH7 | FTM Channel] | PTE16: [FTM2_CH7 | FTM Channel] | PTA2: [FTM3_CH0 | FTM Channel] | PTB8: [FTM3_CH0 | FTM Channel] | PTA3: [FTM3_CH1 | FTM Channel] | PTB9: [FTM3_CH1 | FTM Channel] | PTB10: [FTM3_CH2 | FTM Channel] | PTC6: [FTM3_CH2 | FTM Channel] | PTB11: [FTM3_CH3 | FTM Channel] | PTC7: [FTM3_CH3 | FTM Channel] | PTC10: [FTM3_CH4 | FTM Channel] | PTD2: [FTM3_CH4 | FTM Channel] | PTC11: [FTM3_CH5 | FTM Channel] | PTD3: [FTM3_CH5 | FTM Channel] | PTC12: [FTM3_CH6 | FTM Channel] | PTE2: [FTM3_CH6 | FTM Channel] | PTC13: [FTM3_CH7 | FTM Channel] | PTE6: [FTM3_CH7 | FTM Channel] | PTD15: [FTM0_CH0 | FTM Channel] | PTB13: [FTM0_CH1 | FTM Channel] | PTC1: [FTM0_CH1 | FTM Channel] | PTD16: [FTM0_CH1 | FTM Channel] | PTC2: [FTM0_CH2 | FTM Channel] | PTD0: [FTM0_CH2 | FTM Channel] | PTC3: [FTM0_CH3 | FTM Channel] | PTD1: [FTM0_CH3 | FTM Channel] | PTB4: [FTM0_CH4 | FTM Channel] | PTB5: [FTM0_CH5 | FTM Channel] | PTE8: [FTM0_CH6 | FTM Channel] | PTE9: [FTM0_CH7 | FTM Channel] | PTB2: [FTM1_CH0 | FTM Channel] | PTC4: [FTM1_CH0 | FTM Channel] | PTA1: [FTM1_CH1 | FTM Channel] | PTB3: [FTM1_CH1 | FTM Channel] | PTC14: [FTM1_CH2 | FTM Channel] | PTC15: [FTM1_CH3 | FTM Channel] | PTA10: [FTM1_CH4 | FTM Channel] | PTA11: [FTM1_CH5 | FTM Channel] | PTA12: [FTM1_CH6 | FTM Channel] | PTA13: [FTM1_CH7 | FTM Channel] | PTC1: [FTM1_CH7 | FTM Channel] | PTC5: [FTM2_CH0 | FTM Channel] | PTD0: [FTM2_CH0 | FTM Channel] | PTD10: [FTM2_CH0 | FTM Channel] | PTA0: [FTM2_CH1 | FTM Channel] | PTD1: [FTM2_CH1 | FTM Channel] | PTD11: [FTM2_CH1 | FTM Channel] | PTD12: [FTM2_CH2 | FTM Channel] | PTE4: [FTM2_CH2 | FTM Channel] | PTD5: [FTM2_CH3 | FTM Channel] | PTE5: [FTM2_CH3 | FTM Channel] | PTD13: [FTM2_CH4 | FTM Channel] | PTE10: [FTM2_CH4 | FTM Channel] | PTD14: [FTM2_CH5 | FTM Channel] | PTE11: [FTM2_CH5 | FTM Channel] | PTC12: [FTM2_CH6 | FTM Channel] | PTE15: [FTM2_CH6 | FTM Channel] | PTC13: [FTM2_CH7 | FTM Channel] | PTE16: [FTM2_CH7 | FTM Channel] | PTA2: [FTM3_CH0 | FTM Channel] | PTB8: [FTM3_CH0 | FTM Channel] | PTA3: [FTM3_CH1 | FTM Channel] | PTB9: [FTM3_CH1 | FTM Channel] | PTB10: [FTM3_CH2 | FTM Channel] | PTC6: [FTM3_CH2 | FTM Channel] | PTB11: [FTM3_CH3 | FTM Channel] | PTC7: [FTM3_CH3 | FTM Channel] | PTC10: [FTM3_CH4 | FTM Channel] | PTD2: [FTM3_CH4 | FTM Channel] | PTC11: [FTM3_CH5 | FTM Channel] | PTD3: [FTM3_CH5 | FTM Channel] | PTC12: [FTM3_CH6 | FTM Channel] | PTE2: [FTM3_CH6 | FTM Channel] | PTC13: [FTM3_CH7 | FTM Channel] | PTE6: [FTM3_CH7 | FTM Channel] | PTE20: [FTM4_CH0 | FTM Channel] | PTE21: [FTM4_CH1 | FTM Channel] | PTC11: [FTM4_CH2 | FTM Channel] | PTE22: [FTM4_CH2 | FTM Channel] | PTE23: [FTM4_CH3 | FTM Channel] | PTC27: [FTM4_CH4 | FTM Channel] | PTE24: [FTM4_CH4 | FTM Channel] | PTB1: [FTM4_CH5 | FTM Channel] | PTE13: [FTM4_CH5 | FTM Channel] | PTE25: [FTM4_CH5 | FTM Channel] | PTB0: [FTM4_CH6 | FTM Channel] | PTC28: [FTM4_CH7 | FTM Channel] | PTA25: [FTM5_CH0 | FTM Channel] | PTC9: [FTM5_CH0 | FTM Channel] | PTA26: [FTM5_CH1 | FTM Channel] | PTC8: [FTM5_CH1 | FTM Channel] | PTA27: [FTM5_CH2 | FTM Channel] | PTC29: [FTM5_CH2 | FTM Channel] | PTA7: [FTM5_CH3 | FTM Channel] | PTA28: [FTM5_CH3 | FTM Channel] | PTA29: [FTM5_CH4 | FTM Channel] | PTC30: [FTM5_CH4 | FTM Channel] | PTA6: [FTM5_CH5 | FTM Channel] | PTA30: [FTM5_CH5 | FTM Channel] | PTA31: [FTM5_CH6 | FTM Channel] | PTC31: [FTM5_CH6 | FTM Channel] | PTB18: [FTM5_CH7 | FTM Channel] | PTD18: [FTM5_CH7 | FTM Channel] | PTD15: [FTM0_CH0 | FTM Channel] | PTB13: [FTM0_CH1 | FTM Channel] | PTC1: [FTM0_CH1 | FTM Channel] | PTD16: [FTM0_CH1 | FTM Channel] | PTC2: [FTM0_CH2 | FTM Channel] | PTD0: [FTM0_CH2 | FTM Channel] | PTC3: [FTM0_CH3 | FTM Channel] | PTD1: [FTM0_CH3 | FTM Channel] | PTB4: [FTM0_CH4 | FTM Channel] | PTB5: [FTM0_CH5 | FTM Channel] | PTE8: [FTM0_CH6 | FTM Channel] | PTE9: [FTM0_CH7 | FTM Channel] | PTB2: [FTM1_CH0 | FTM Channel] | PTC4: [FTM1_CH0 | FTM Channel] | PTA1: [FTM1_CH1 | FTM Channel] | PTB3: [FTM1_CH1 | FTM Channel] | PTC14: [FTM1_CH2 | FTM Channel] | PTC15: [FTM1_CH3 | FTM Channel] | PTA10: [FTM1_CH4 | FTM Channel] | PTA11: [FTM1_CH5 | FTM Channel] | PTA12: [FTM1_CH6 | FTM Channel] | PTA13: [FTM1_CH7 | FTM Channel] | PTC1: [FTM1_CH7 | FTM Channel] | PTC5: [FTM2_CH0 | FTM Channel] | PTD0: [FTM2_CH0 | FTM Channel] | PTD10: [FTM2_CH0 | FTM Channel] | PTA0: [FTM2_CH1 | FTM Channel] | PTD1: [FTM2_CH1 | FTM Channel] | PTD11: [FTM2_CH1 | FTM Channel] | PTD12: [FTM2_CH2 | FTM Channel] | PTE4: [FTM2_CH2 | FTM Channel] | PTD5: [FTM2_CH3 | FTM Channel] | PTE5: [FTM2_CH3 | FTM Channel] | PTD13: [FTM2_CH4 | FTM Channel] | PTE10: [FTM2_CH4 | FTM Channel] | PTD14: [FTM2_CH5 | FTM Channel] | PTE11: [FTM2_CH5 | FTM Channel] | PTC12: [FTM2_CH6 | FTM Channel] | PTE15: [FTM2_CH6 | FTM Channel] | PTC13: [FTM2_CH7 | FTM Channel] | PTE16: [FTM2_CH7 | FTM Channel] | PTA2: [FTM3_CH0 | FTM Channel] | PTB8: [FTM3_CH0 | FTM Channel] | PTA3: [FTM3_CH1 | FTM Channel] | PTB9: [FTM3_CH1 | FTM Channel] | PTB10: [FTM3_CH2 | FTM Channel] | PTC6: [FTM3_CH2 | FTM Channel] | PTB11: [FTM3_CH3 | FTM Channel] | PTC7: [FTM3_CH3 | FTM Channel] | PTC10: [FTM3_CH4 | FTM Channel] | PTD2: [FTM3_CH4 | FTM Channel] | PTC11: [FTM3_CH5 | FTM Channel] | PTD3: [FTM3_CH5 | FTM Channel] | PTC12: [FTM3_CH6 | FTM Channel] | PTE2: [FTM3_CH6 | FTM Channel] | PTC13: [FTM3_CH7 | FTM Channel] | PTE6: [FTM3_CH7 | FTM Channel] | PTE20: [FTM4_CH0 | FTM Channel] | PTE21: [FTM4_CH1 | FTM Channel] | PTC11: [FTM4_CH2 | FTM Channel] | PTE22: [FTM4_CH2 | FTM Channel] | PTE23: [FTM4_CH3 | FTM Channel] | PTC27: [FTM4_CH4 | FTM Channel] | PTE24: [FTM4_CH4 | FTM Channel] | PTB1: [FTM4_CH5 | FTM Channel] | PTE13: [FTM4_CH5 | FTM Channel] | PTE25: [FTM4_CH5 | FTM Channel] | PTB0: [FTM4_CH6 | FTM Channel] | PTC28: [FTM4_CH7 | FTM Channel] | PTA25: [FTM5_CH0 | FTM Channel] | PTC9: [FTM5_CH0 | FTM Channel] | PTA26: [FTM5_CH1 | FTM Channel] | PTC8: [FTM5_CH1 | FTM Channel] | PTA27: [FTM5_CH2 | FTM Channel] | PTC29: [FTM5_CH2 | FTM Channel] | PTA7: [FTM5_CH3 | FTM Channel] | PTA28: [FTM5_CH3 | FTM Channel] | PTA29: [FTM5_CH4 | FTM Channel] | PTC30: [FTM5_CH4 | FTM Channel] | PTA6: [FTM5_CH5 | FTM Channel] | PTA30: [FTM5_CH5 | FTM Channel] | PTA31: [FTM5_CH6 | FTM Channel] | PTC31: [FTM5_CH6 | FTM Channel] | PTB18: [FTM5_CH7 | FTM Channel] | PTD18: [FTM5_CH7 | FTM Channel] | PTA18: [FTM6_CH0 | FTM Channel] | PTB20: [FTM6_CH0 | FTM Channel] | PTD19: [FTM6_CH0 | FTM Channel] | PTB21: [FTM6_CH1 | FTM Channel] | PTD20: [FTM6_CH1 | FTM Channel] | PTB22: [FTM6_CH2 | FTM Channel] | PTD21: [FTM6_CH2 | FTM Channel] | PTB23: [FTM6_CH3 | FTM Channel] | PTD22: [FTM6_CH3 | FTM Channel] | PTB24: [FTM6_CH4 | FTM Channel] | PTD23: [FTM6_CH4 | FTM Channel] | PTB25: [FTM6_CH5 | FTM Channel] | PTD24: [FTM6_CH5 | FTM Channel] | PTB26: [FTM6_CH6 | FTM Channel] | PTD25: [FTM6_CH6 | FTM Channel] | PTB27: [FTM6_CH7 | FTM Channel] | PTD26: [FTM6_CH7 | FTM Channel] | PTB28: [FTM7_CH0 | FTM Channel] | PTD27: [FTM7_CH0 | FTM Channel] | PTB29: [FTM7_CH1 | FTM Channel] | PTD28: [FTM7_CH1 | FTM Channel] | PTB30: [FTM7_CH2 | FTM Channel] | PTD29: [FTM7_CH2 | FTM Channel] | PTB31: [FTM7_CH3 | FTM Channel] | PTD30: [FTM7_CH3 | FTM Channel] | PTC18: [FTM7_CH4 | FTM Channel] | PTD31: [FTM7_CH4 | FTM Channel] | PTC19: [FTM7_CH5 | FTM Channel] | PTE17: [FTM7_CH5 | FTM Channel] | PTC20: [FTM7_CH6 | FTM Channel] | PTE18: [FTM7_CH6 | FTM Channel] | PTC21: [FTM7_CH7 | FTM Channel] | PTE19: [FTM7_CH7 | FTM Channel]
      mask TypeOptions pinPolCh0: Active Low | Active High
      mask TypeOptions pinPolCh1: Active Low | Active High
      mask TypeOptions outputComplem0: Main duplicated | Main inverted
      mask TypeOptions outputLevel0: Low | High
      mask TypeOptions outputLevel1: Low | High
      mask TypeOptions pinFtmCh2: PTD15: [FTM0_CH0 | FTM Channel] | PTB13: [FTM0_CH1 | FTM Channel] | PTC1: [FTM0_CH1 | FTM Channel] | PTD16: [FTM0_CH1 | FTM Channel] | PTC2: [FTM0_CH2 | FTM Channel] | PTD0: [FTM0_CH2 | FTM Channel] | PTC3: [FTM0_CH3 | FTM Channel] | PTD1: [FTM0_CH3 | FTM Channel] | PTB4: [FTM0_CH4 | FTM Channel] | PTB5: [FTM0_CH5 | FTM Channel] | PTE8: [FTM0_CH6 | FTM Channel] | PTE9: [FTM0_CH7 | FTM Channel] | PTB2: [FTM1_CH0 | FTM Channel] | PTC4: [FTM1_CH0 | FTM Channel] | PTA1: [FTM1_CH1 | FTM Channel] | PTB3: [FTM1_CH1 | FTM Channel] | PTC14: [FTM1_CH2 | FTM Channel] | PTC15: [FTM1_CH3 | FTM Channel] | PTA10: [FTM1_CH4 | FTM Channel] | PTA11: [FTM1_CH5 | FTM Channel] | PTA12: [FTM1_CH6 | FTM Channel] | PTA13: [FTM1_CH7 | FTM Channel] | PTC1: [FTM1_CH7 | FTM Channel] | PTD15: [FTM0_CH0 | FTM Channel] | PTB13: [FTM0_CH1 | FTM Channel] | PTC1: [FTM0_CH1 | FTM Channel] | PTD16: [FTM0_CH1 | FTM Channel] | PTC2: [FTM0_CH2 | FTM Channel] | PTD0: [FTM0_CH2 | FTM Channel] | PTC3: [FTM0_CH3 | FTM Channel] | PTD1: [FTM0_CH3 | FTM Channel] | PTB4: [FTM0_CH4 | FTM Channel] | PTB5: [FTM0_CH5 | FTM Channel] | PTE8: [FTM0_CH6 | FTM Channel] | PTE9: [FTM0_CH7 | FTM Channel] | PTB2: [FTM1_CH0 | FTM Channel] | PTC4: [FTM1_CH0 | FTM Channel] | PTA1: [FTM1_CH1 | FTM Channel] | PTB3: [FTM1_CH1 | FTM Channel] | PTC14: [FTM1_CH2 | FTM Channel] | PTC15: [FTM1_CH3 | FTM Channel] | PTA10: [FTM1_CH4 | FTM Channel] | PTA11: [FTM1_CH5 | FTM Channel] | PTA12: [FTM1_CH6 | FTM Channel] | PTA13: [FTM1_CH7 | FTM Channel] | PTC1: [FTM1_CH7 | FTM Channel] | PTD15: [FTM0_CH0 | FTM Channel] | PTB13: [FTM0_CH1 | FTM Channel] | PTC1: [FTM0_CH1 | FTM Channel] | PTD16: [FTM0_CH1 | FTM Channel] | PTC2: [FTM0_CH2 | FTM Channel] | PTD0: [FTM0_CH2 | FTM Channel] | PTC3: [FTM0_CH3 | FTM Channel] | PTD1: [FTM0_CH3 | FTM Channel] | PTB4: [FTM0_CH4 | FTM Channel] | PTB5: [FTM0_CH5 | FTM Channel] | PTE8: [FTM0_CH6 | FTM Channel] | PTE9: [FTM0_CH7 | FTM Channel] | PTB2: [FTM1_CH0 | FTM Channel] | PTC4: [FTM1_CH0 | FTM Channel] | PTA1: [FTM1_CH1 | FTM Channel] | PTB3: [FTM1_CH1 | FTM Channel] | PTC14: [FTM1_CH2 | FTM Channel] | PTC15: [FTM1_CH3 | FTM Channel] | PTA10: [FTM1_CH4 | FTM Channel] | PTA11: [FTM1_CH5 | FTM Channel] | PTA12: [FTM1_CH6 | FTM Channel] | PTA13: [FTM1_CH7 | FTM Channel] | PTC1: [FTM1_CH7 | FTM Channel] | PTC5: [FTM2_CH0 | FTM Channel] | PTD0: [FTM2_CH0 | FTM Channel] | PTD10: [FTM2_CH0 | FTM Channel] | PTA0: [FTM2_CH1 | FTM Channel] | PTD1: [FTM2_CH1 | FTM Channel] | PTD11: [FTM2_CH1 | FTM Channel] | PTD12: [FTM2_CH2 | FTM Channel] | PTE4: [FTM2_CH2 | FTM Channel] | PTD5: [FTM2_CH3 | FTM Channel] | PTE5: [FTM2_CH3 | FTM Channel] | PTD13: [FTM2_CH4 | FTM Channel] | PTE10: [FTM2_CH4 | FTM Channel] | PTD14: [FTM2_CH5 | FTM Channel] | PTE11: [FTM2_CH5 | FTM Channel] | PTC12: [FTM2_CH6 | FTM Channel] | PTE15: [FTM2_CH6 | FTM Channel] | PTC13: [FTM2_CH7 | FTM Channel] | PTE16: [FTM2_CH7 | FTM Channel] | PTA2: [FTM3_CH0 | FTM Channel] | PTB8: [FTM3_CH0 | FTM Channel] | PTA3: [FTM3_CH1 | FTM Channel] | PTB9: [FTM3_CH1 | FTM Channel] | PTB10: [FTM3_CH2 | FTM Channel] | PTC6: [FTM3_CH2 | FTM Channel] | PTB11: [FTM3_CH3 | FTM Channel] | PTC7: [FTM3_CH3 | FTM Channel] | PTC10: [FTM3_CH4 | FTM Channel] | PTD2: [FTM3_CH4 | FTM Channel] | PTC11: [FTM3_CH5 | FTM Channel] | PTD3: [FTM3_CH5 | FTM Channel] | PTC12: [FTM3_CH6 | FTM Channel] | PTE2: [FTM3_CH6 | FTM Channel] | PTC13: [FTM3_CH7 | FTM Channel] | PTE6: [FTM3_CH7 | FTM Channel] | PTD15: [FTM0_CH0 | FTM Channel] | PTB13: [FTM0_CH1 | FTM Channel] | PTC1: [FTM0_CH1 | FTM Channel] | PTD16: [FTM0_CH1 | FTM Channel] | PTC2: [FTM0_CH2 | FTM Channel] | PTD0: [FTM0_CH2 | FTM Channel] | PTC3: [FTM0_CH3 | FTM Channel] | PTD1: [FTM0_CH3 | FTM Channel] | PTB4: [FTM0_CH4 | FTM Channel] | PTB5: [FTM0_CH5 | FTM Channel] | PTE8: [FTM0_CH6 | FTM Channel] | PTE9: [FTM0_CH7 | FTM Channel] | PTB2: [FTM1_CH0 | FTM Channel] | PTC4: [FTM1_CH0 | FTM Channel] | PTA1: [FTM1_CH1 | FTM Channel] | PTB3: [FTM1_CH1 | FTM Channel] | PTC14: [FTM1_CH2 | FTM Channel] | PTC15: [FTM1_CH3 | FTM Channel] | PTA10: [FTM1_CH4 | FTM Channel] | PTA11: [FTM1_CH5 | FTM Channel] | PTA12: [FTM1_CH6 | FTM Channel] | PTA13: [FTM1_CH7 | FTM Channel] | PTC1: [FTM1_CH7 | FTM Channel] | PTC5: [FTM2_CH0 | FTM Channel] | PTD0: [FTM2_CH0 | FTM Channel] | PTD10: [FTM2_CH0 | FTM Channel] | PTA0: [FTM2_CH1 | FTM Channel] | PTD1: [FTM2_CH1 | FTM Channel] | PTD11: [FTM2_CH1 | FTM Channel] | PTD12: [FTM2_CH2 | FTM Channel] | PTE4: [FTM2_CH2 | FTM Channel] | PTD5: [FTM2_CH3 | FTM Channel] | PTE5: [FTM2_CH3 | FTM Channel] | PTD13: [FTM2_CH4 | FTM Channel] | PTE10: [FTM2_CH4 | FTM Channel] | PTD14: [FTM2_CH5 | FTM Channel] | PTE11: [FTM2_CH5 | FTM Channel] | PTC12: [FTM2_CH6 | FTM Channel] | PTE15: [FTM2_CH6 | FTM Channel] | PTC13: [FTM2_CH7 | FTM Channel] | PTE16: [FTM2_CH7 | FTM Channel] | PTA2: [FTM3_CH0 | FTM Channel] | PTB8: [FTM3_CH0 | FTM Channel] | PTA3: [FTM3_CH1 | FTM Channel] | PTB9: [FTM3_CH1 | FTM Channel] | PTB10: [FTM3_CH2 | FTM Channel] | PTC6: [FTM3_CH2 | FTM Channel] | PTB11: [FTM3_CH3 | FTM Channel] | PTC7: [FTM3_CH3 | FTM Channel] | PTC10: [FTM3_CH4 | FTM Channel] | PTD2: [FTM3_CH4 | FTM Channel] | PTC11: [FTM3_CH5 | FTM Channel] | PTD3: [FTM3_CH5 | FTM Channel] | PTC12: [FTM3_CH6 | FTM Channel] | PTE2: [FTM3_CH6 | FTM Channel] | PTC13: [FTM3_CH7 | FTM Channel] | PTE6: [FTM3_CH7 | FTM Channel] | PTD15: [FTM0_CH0 | FTM Channel] | PTB13: [FTM0_CH1 | FTM Channel] | PTC1: [FTM0_CH1 | FTM Channel] | PTD16: [FTM0_CH1 | FTM Channel] | PTC2: [FTM0_CH2 | FTM Channel] | PTD0: [FTM0_CH2 | FTM Channel] | PTC3: [FTM0_CH3 | FTM Channel] | PTD1: [FTM0_CH3 | FTM Channel] | PTB4: [FTM0_CH4 | FTM Channel] | PTB5: [FTM0_CH5 | FTM Channel] | PTE8: [FTM0_CH6 | FTM Channel] | PTE9: [FTM0_CH7 | FTM Channel] | PTB2: [FTM1_CH0 | FTM Channel] | PTC4: [FTM1_CH0 | FTM Channel] | PTA1: [FTM1_CH1 | FTM Channel] | PTB3: [FTM1_CH1 | FTM Channel] | PTC14: [FTM1_CH2 | FTM Channel] | PTC15: [FTM1_CH3 | FTM Channel] | PTA10: [FTM1_CH4 | FTM Channel] | PTA11: [FTM1_CH5 | FTM Channel] | PTA12: [FTM1_CH6 | FTM Channel] | PTA13: [FTM1_CH7 | FTM Channel] | PTC1: [FTM1_CH7 | FTM Channel] | PTC5: [FTM2_CH0 | FTM Channel] | PTD0: [FTM2_CH0 | FTM Channel] | PTD10: [FTM2_CH0 | FTM Channel] | PTA0: [FTM2_CH1 | FTM Channel] | PTD1: [FTM2_CH1 | FTM Channel] | PTD11: [FTM2_CH1 | FTM Channel] | PTD12: [FTM2_CH2 | FTM Channel] | PTE4: [FTM2_CH2 | FTM Channel] | PTD5: [FTM2_CH3 | FTM Channel] | PTE5: [FTM2_CH3 | FTM Channel] | PTD13: [FTM2_CH4 | FTM Channel] | PTE10: [FTM2_CH4 | FTM Channel] | PTD14: [FTM2_CH5 | FTM Channel] | PTE11: [FTM2_CH5 | FTM Channel] | PTC12: [FTM2_CH6 | FTM Channel] | PTE15: [FTM2_CH6 | FTM Channel] | PTC13: [FTM2_CH7 | FTM Channel] | PTE16: [FTM2_CH7 | FTM Channel] | PTA2: [FTM3_CH0 | FTM Channel] | PTB8: [FTM3_CH0 | FTM Channel] | PTA3: [FTM3_CH1 | FTM Channel] | PTB9: [FTM3_CH1 | FTM Channel] | PTB10: [FTM3_CH2 | FTM Channel] | PTC6: [FTM3_CH2 | FTM Channel] | PTB11: [FTM3_CH3 | FTM Channel] | PTC7: [FTM3_CH3 | FTM Channel] | PTC10: [FTM3_CH4 | FTM Channel] | PTD2: [FTM3_CH4 | FTM Channel] | PTC11: [FTM3_CH5 | FTM Channel] | PTD3: [FTM3_CH5 | FTM Channel] | PTC12: [FTM3_CH6 | FTM Channel] | PTE2: [FTM3_CH6 | FTM Channel] | PTC13: [FTM3_CH7 | FTM Channel] | PTE6: [FTM3_CH7 | FTM Channel] | PTE20: [FTM4_CH0 | FTM Channel] | PTE21: [FTM4_CH1 | FTM Channel] | PTC11: [FTM4_CH2 | FTM Channel] | PTE22: [FTM4_CH2 | FTM Channel] | PTE23: [FTM4_CH3 | FTM Channel] | PTC27: [FTM4_CH4 | FTM Channel] | PTE24: [FTM4_CH4 | FTM Channel] | PTB1: [FTM4_CH5 | FTM Channel] | PTE13: [FTM4_CH5 | FTM Channel] | PTE25: [FTM4_CH5 | FTM Channel] | PTB0: [FTM4_CH6 | FTM Channel] | PTC28: [FTM4_CH7 | FTM Channel] | PTA25: [FTM5_CH0 | FTM Channel] | PTC9: [FTM5_CH0 | FTM Channel] | PTA26: [FTM5_CH1 | FTM Channel] | PTC8: [FTM5_CH1 | FTM Channel] | PTA27: [FTM5_CH2 | FTM Channel] | PTC29: [FTM5_CH2 | FTM Channel] | PTA7: [FTM5_CH3 | FTM Channel] | PTA28: [FTM5_CH3 | FTM Channel] | PTA29: [FTM5_CH4 | FTM Channel] | PTC30: [FTM5_CH4 | FTM Channel] | PTA6: [FTM5_CH5 | FTM Channel] | PTA30: [FTM5_CH5 | FTM Channel] | PTA31: [FTM5_CH6 | FTM Channel] | PTC31: [FTM5_CH6 | FTM Channel] | PTB18: [FTM5_CH7 | FTM Channel] | PTD18: [FTM5_CH7 | FTM Channel] | PTD15: [FTM0_CH0 | FTM Channel] | PTB13: [FTM0_CH1 | FTM Channel] | PTC1: [FTM0_CH1 | FTM Channel] | PTD16: [FTM0_CH1 | FTM Channel] | PTC2: [FTM0_CH2 | FTM Channel] | PTD0: [FTM0_CH2 | FTM Channel] | PTC3: [FTM0_CH3 | FTM Channel] | PTD1: [FTM0_CH3 | FTM Channel] | PTB4: [FTM0_CH4 | FTM Channel] | PTB5: [FTM0_CH5 | FTM Channel] | PTE8: [FTM0_CH6 | FTM Channel] | PTE9: [FTM0_CH7 | FTM Channel] | PTB2: [FTM1_CH0 | FTM Channel] | PTC4: [FTM1_CH0 | FTM Channel] | PTA1: [FTM1_CH1 | FTM Channel] | PTB3: [FTM1_CH1 | FTM Channel] | PTC14: [FTM1_CH2 | FTM Channel] | PTC15: [FTM1_CH3 | FTM Channel] | PTA10: [FTM1_CH4 | FTM Channel] | PTA11: [FTM1_CH5 | FTM Channel] | PTA12: [FTM1_CH6 | FTM Channel] | PTA13: [FTM1_CH7 | FTM Channel] | PTC1: [FTM1_CH7 | FTM Channel] | PTC5: [FTM2_CH0 | FTM Channel] | PTD0: [FTM2_CH0 | FTM Channel] | PTD10: [FTM2_CH0 | FTM Channel] | PTA0: [FTM2_CH1 | FTM Channel] | PTD1: [FTM2_CH1 | FTM Channel] | PTD11: [FTM2_CH1 | FTM Channel] | PTD12: [FTM2_CH2 | FTM Channel] | PTE4: [FTM2_CH2 | FTM Channel] | PTD5: [FTM2_CH3 | FTM Channel] | PTE5: [FTM2_CH3 | FTM Channel] | PTD13: [FTM2_CH4 | FTM Channel] | PTE10: [FTM2_CH4 | FTM Channel] | PTD14: [FTM2_CH5 | FTM Channel] | PTE11: [FTM2_CH5 | FTM Channel] | PTC12: [FTM2_CH6 | FTM Channel] | PTE15: [FTM2_CH6 | FTM Channel] | PTC13: [FTM2_CH7 | FTM Channel] | PTE16: [FTM2_CH7 | FTM Channel] | PTA2: [FTM3_CH0 | FTM Channel] | PTB8: [FTM3_CH0 | FTM Channel] | PTA3: [FTM3_CH1 | FTM Channel] | PTB9: [FTM3_CH1 | FTM Channel] | PTB10: [FTM3_CH2 | FTM Channel] | PTC6: [FTM3_CH2 | FTM Channel] | PTB11: [FTM3_CH3 | FTM Channel] | PTC7: [FTM3_CH3 | FTM Channel] | PTC10: [FTM3_CH4 | FTM Channel] | PTD2: [FTM3_CH4 | FTM Channel] | PTC11: [FTM3_CH5 | FTM Channel] | PTD3: [FTM3_CH5 | FTM Channel] | PTC12: [FTM3_CH6 | FTM Channel] | PTE2: [FTM3_CH6 | FTM Channel] | PTC13: [FTM3_CH7 | FTM Channel] | PTE6: [FTM3_CH7 | FTM Channel] | PTE20: [FTM4_CH0 | FTM Channel] | PTE21: [FTM4_CH1 | FTM Channel] | PTC11: [FTM4_CH2 | FTM Channel] | PTE22: [FTM4_CH2 | FTM Channel] | PTE23: [FTM4_CH3 | FTM Channel] | PTC27: [FTM4_CH4 | FTM Channel] | PTE24: [FTM4_CH4 | FTM Channel] | PTB1: [FTM4_CH5 | FTM Channel] | PTE13: [FTM4_CH5 | FTM Channel] | PTE25: [FTM4_CH5 | FTM Channel] | PTB0: [FTM4_CH6 | FTM Channel] | PTC28: [FTM4_CH7 | FTM Channel] | PTA25: [FTM5_CH0 | FTM Channel] | PTC9: [FTM5_CH0 | FTM Channel] | PTA26: [FTM5_CH1 | FTM Channel] | PTC8: [FTM5_CH1 | FTM Channel] | PTA27: [FTM5_CH2 | FTM Channel] | PTC29: [FTM5_CH2 | FTM Channel] | PTA7: [FTM5_CH3 | FTM Channel] | PTA28: [FTM5_CH3 | FTM Channel] | PTA29: [FTM5_CH4 | FTM Channel] | PTC30: [FTM5_CH4 | FTM Channel] | PTA6: [FTM5_CH5 | FTM Channel] | PTA30: [FTM5_CH5 | FTM Channel] | PTA31: [FTM5_CH6 | FTM Channel] | PTC31: [FTM5_CH6 | FTM Channel] | PTB18: [FTM5_CH7 | FTM Channel] | PTD18: [FTM5_CH7 | FTM Channel] | PTA18: [FTM6_CH0 | FTM Channel] | PTB20: [FTM6_CH0 | FTM Channel] | PTD19: [FTM6_CH0 | FTM Channel] | PTB21: [FTM6_CH1 | FTM Channel] | PTD20: [FTM6_CH1 | FTM Channel] | PTB22: [FTM6_CH2 | FTM Channel] | PTD21: [FTM6_CH2 | FTM Channel] | PTB23: [FTM6_CH3 | FTM Channel] | PTD22: [FTM6_CH3 | FTM Channel] | PTB24: [FTM6_CH4 | FTM Channel] | PTD23: [FTM6_CH4 | FTM Channel] | PTB25: [FTM6_CH5 | FTM Channel] | PTD24: [FTM6_CH5 | FTM Channel] | PTB26: [FTM6_CH6 | FTM Channel] | PTD25: [FTM6_CH6 | FTM Channel] | PTB27: [FTM6_CH7 | FTM Channel] | PTD26: [FTM6_CH7 | FTM Channel] | PTB28: [FTM7_CH0 | FTM Channel] | PTD27: [FTM7_CH0 | FTM Channel] | PTB29: [FTM7_CH1 | FTM Channel] | PTD28: [FTM7_CH1 | FTM Channel] | PTB30: [FTM7_CH2 | FTM Channel] | PTD29: [FTM7_CH2 | FTM Channel] | PTB31: [FTM7_CH3 | FTM Channel] | PTD30: [FTM7_CH3 | FTM Channel] | PTC18: [FTM7_CH4 | FTM Channel] | PTD31: [FTM7_CH4 | FTM Channel] | PTC19: [FTM7_CH5 | FTM Channel] | PTE17: [FTM7_CH5 | FTM Channel] | PTC20: [FTM7_CH6 | FTM Channel] | PTE18: [FTM7_CH6 | FTM Channel] | PTC21: [FTM7_CH7 | FTM Channel] | PTE19: [FTM7_CH7 | FTM Channel]
      mask TypeOptions pinFtmCh3: None | PTD15: [FTM0_CH0 | FTM Channel] | PTB13: [FTM0_CH1 | FTM Channel] | PTC1: [FTM0_CH1 | FTM Channel] | PTD16: [FTM0_CH1 | FTM Channel] | PTC2: [FTM0_CH2 | FTM Channel] | PTD0: [FTM0_CH2 | FTM Channel] | PTC3: [FTM0_CH3 | FTM Channel] | PTD1: [FTM0_CH3 | FTM Channel] | PTB4: [FTM0_CH4 | FTM Channel] | PTB5: [FTM0_CH5 | FTM Channel] | PTE8: [FTM0_CH6 | FTM Channel] | PTE9: [FTM0_CH7 | FTM Channel] | PTB2: [FTM1_CH0 | FTM Channel] | PTC4: [FTM1_CH0 | FTM Channel] | PTA1: [FTM1_CH1 | FTM Channel] | PTB3: [FTM1_CH1 | FTM Channel] | PTC14: [FTM1_CH2 | FTM Channel] | PTC15: [FTM1_CH3 | FTM Channel] | PTA10: [FTM1_CH4 | FTM Channel] | PTA11: [FTM1_CH5 | FTM Channel] | PTA12: [FTM1_CH6 | FTM Channel] | PTA13: [FTM1_CH7 | FTM Channel] | PTC1: [FTM1_CH7 | FTM Channel] | PTD15: [FTM0_CH0 | FTM Channel] | PTB13: [FTM0_CH1 | FTM Channel] | PTC1: [FTM0_CH1 | FTM Channel] | PTD16: [FTM0_CH1 | FTM Channel] | PTC2: [FTM0_CH2 | FTM Channel] | PTD0: [FTM0_CH2 | FTM Channel] | PTC3: [FTM0_CH3 | FTM Channel] | PTD1: [FTM0_CH3 | FTM Channel] | PTB4: [FTM0_CH4 | FTM Channel] | PTB5: [FTM0_CH5 | FTM Channel] | PTE8: [FTM0_CH6 | FTM Channel] | PTE9: [FTM0_CH7 | FTM Channel] | PTB2: [FTM1_CH0 | FTM Channel] | PTC4: [FTM1_CH0 | FTM Channel] | PTA1: [FTM1_CH1 | FTM Channel] | PTB3: [FTM1_CH1 | FTM Channel] | PTC14: [FTM1_CH2 | FTM Channel] | PTC15: [FTM1_CH3 | FTM Channel] | PTA10: [FTM1_CH4 | FTM Channel] | PTA11: [FTM1_CH5 | FTM Channel] | PTA12: [FTM1_CH6 | FTM Channel] | PTA13: [FTM1_CH7 | FTM Channel] | PTC1: [FTM1_CH7 | FTM Channel] | PTD15: [FTM0_CH0 | FTM Channel] | PTB13: [FTM0_CH1 | FTM Channel] | PTC1: [FTM0_CH1 | FTM Channel] | PTD16: [FTM0_CH1 | FTM Channel] | PTC2: [FTM0_CH2 | FTM Channel] | PTD0: [FTM0_CH2 | FTM Channel] | PTC3: [FTM0_CH3 | FTM Channel] | PTD1: [FTM0_CH3 | FTM Channel] | PTB4: [FTM0_CH4 | FTM Channel] | PTB5: [FTM0_CH5 | FTM Channel] | PTE8: [FTM0_CH6 | FTM Channel] | PTE9: [FTM0_CH7 | FTM Channel] | PTB2: [FTM1_CH0 | FTM Channel] | PTC4: [FTM1_CH0 | FTM Channel] | PTA1: [FTM1_CH1 | FTM Channel] | PTB3: [FTM1_CH1 | FTM Channel] | PTC14: [FTM1_CH2 | FTM Channel] | PTC15: [FTM1_CH3 | FTM Channel] | PTA10: [FTM1_CH4 | FTM Channel] | PTA11: [FTM1_CH5 | FTM Channel] | PTA12: [FTM1_CH6 | FTM Channel] | PTA13: [FTM1_CH7 | FTM Channel] | PTC1: [FTM1_CH7 | FTM Channel] | PTC5: [FTM2_CH0 | FTM Channel] | PTD0: [FTM2_CH0 | FTM Channel] | PTD10: [FTM2_CH0 | FTM Channel] | PTA0: [FTM2_CH1 | FTM Channel] | PTD1: [FTM2_CH1 | FTM Channel] | PTD11: [FTM2_CH1 | FTM Channel] | PTD12: [FTM2_CH2 | FTM Channel] | PTE4: [FTM2_CH2 | FTM Channel] | PTD5: [FTM2_CH3 | FTM Channel] | PTE5: [FTM2_CH3 | FTM Channel] | PTD13: [FTM2_CH4 | FTM Channel] | PTE10: [FTM2_CH4 | FTM Channel] | PTD14: [FTM2_CH5 | FTM Channel] | PTE11: [FTM2_CH5 | FTM Channel] | PTC12: [FTM2_CH6 | FTM Channel] | PTE15: [FTM2_CH6 | FTM Channel] | PTC13: [FTM2_CH7 | FTM Channel] | PTE16: [FTM2_CH7 | FTM Channel] | PTA2: [FTM3_CH0 | FTM Channel] | PTB8: [FTM3_CH0 | FTM Channel] | PTA3: [FTM3_CH1 | FTM Channel] | PTB9: [FTM3_CH1 | FTM Channel] | PTB10: [FTM3_CH2 | FTM Channel] | PTC6: [FTM3_CH2 | FTM Channel] | PTB11: [FTM3_CH3 | FTM Channel] | PTC7: [FTM3_CH3 | FTM Channel] | PTC10: [FTM3_CH4 | FTM Channel] | PTD2: [FTM3_CH4 | FTM Channel] | PTC11: [FTM3_CH5 | FTM Channel] | PTD3: [FTM3_CH5 | FTM Channel] | PTC12: [FTM3_CH6 | FTM Channel] | PTE2: [FTM3_CH6 | FTM Channel] | PTC13: [FTM3_CH7 | FTM Channel] | PTE6: [FTM3_CH7 | FTM Channel] | PTD15: [FTM0_CH0 | FTM Channel] | PTB13: [FTM0_CH1 | FTM Channel] | PTC1: [FTM0_CH1 | FTM Channel] | PTD16: [FTM0_CH1 | FTM Channel] | PTC2: [FTM0_CH2 | FTM Channel] | PTD0: [FTM0_CH2 | FTM Channel] | PTC3: [FTM0_CH3 | FTM Channel] | PTD1: [FTM0_CH3 | FTM Channel] | PTB4: [FTM0_CH4 | FTM Channel] | PTB5: [FTM0_CH5 | FTM Channel] | PTE8: [FTM0_CH6 | FTM Channel] | PTE9: [FTM0_CH7 | FTM Channel] | PTB2: [FTM1_CH0 | FTM Channel] | PTC4: [FTM1_CH0 | FTM Channel] | PTA1: [FTM1_CH1 | FTM Channel] | PTB3: [FTM1_CH1 | FTM Channel] | PTC14: [FTM1_CH2 | FTM Channel] | PTC15: [FTM1_CH3 | FTM Channel] | PTA10: [FTM1_CH4 | FTM Channel] | PTA11: [FTM1_CH5 | FTM Channel] | PTA12: [FTM1_CH6 | FTM Channel] | PTA13: [FTM1_CH7 | FTM Channel] | PTC1: [FTM1_CH7 | FTM Channel] | PTC5: [FTM2_CH0 | FTM Channel] | PTD0: [FTM2_CH0 | FTM Channel] | PTD10: [FTM2_CH0 | FTM Channel] | PTA0: [FTM2_CH1 | FTM Channel] | PTD1: [FTM2_CH1 | FTM Channel] | PTD11: [FTM2_CH1 | FTM Channel] | PTD12: [FTM2_CH2 | FTM Channel] | PTE4: [FTM2_CH2 | FTM Channel] | PTD5: [FTM2_CH3 | FTM Channel] | PTE5: [FTM2_CH3 | FTM Channel] | PTD13: [FTM2_CH4 | FTM Channel] | PTE10: [FTM2_CH4 | FTM Channel] | PTD14: [FTM2_CH5 | FTM Channel] | PTE11: [FTM2_CH5 | FTM Channel] | PTC12: [FTM2_CH6 | FTM Channel] | PTE15: [FTM2_CH6 | FTM Channel] | PTC13: [FTM2_CH7 | FTM Channel] | PTE16: [FTM2_CH7 | FTM Channel] | PTA2: [FTM3_CH0 | FTM Channel] | PTB8: [FTM3_CH0 | FTM Channel] | PTA3: [FTM3_CH1 | FTM Channel] | PTB9: [FTM3_CH1 | FTM Channel] | PTB10: [FTM3_CH2 | FTM Channel] | PTC6: [FTM3_CH2 | FTM Channel] | PTB11: [FTM3_CH3 | FTM Channel] | PTC7: [FTM3_CH3 | FTM Channel] | PTC10: [FTM3_CH4 | FTM Channel] | PTD2: [FTM3_CH4 | FTM Channel] | PTC11: [FTM3_CH5 | FTM Channel] | PTD3: [FTM3_CH5 | FTM Channel] | PTC12: [FTM3_CH6 | FTM Channel] | PTE2: [FTM3_CH6 | FTM Channel] | PTC13: [FTM3_CH7 | FTM Channel] | PTE6: [FTM3_CH7 | FTM Channel] | PTD15: [FTM0_CH0 | FTM Channel] | PTB13: [FTM0_CH1 | FTM Channel] | PTC1: [FTM0_CH1 | FTM Channel] | PTD16: [FTM0_CH1 | FTM Channel] | PTC2: [FTM0_CH2 | FTM Channel] | PTD0: [FTM0_CH2 | FTM Channel] | PTC3: [FTM0_CH3 | FTM Channel] | PTD1: [FTM0_CH3 | FTM Channel] | PTB4: [FTM0_CH4 | FTM Channel] | PTB5: [FTM0_CH5 | FTM Channel] | PTE8: [FTM0_CH6 | FTM Channel] | PTE9: [FTM0_CH7 | FTM Channel] | PTB2: [FTM1_CH0 | FTM Channel] | PTC4: [FTM1_CH0 | FTM Channel] | PTA1: [FTM1_CH1 | FTM Channel] | PTB3: [FTM1_CH1 | FTM Channel] | PTC14: [FTM1_CH2 | FTM Channel] | PTC15: [FTM1_CH3 | FTM Channel] | PTA10: [FTM1_CH4 | FTM Channel] | PTA11: [FTM1_CH5 | FTM Channel] | PTA12: [FTM1_CH6 | FTM Channel] | PTA13: [FTM1_CH7 | FTM Channel] | PTC1: [FTM1_CH7 | FTM Channel] | PTC5: [FTM2_CH0 | FTM Channel] | PTD0: [FTM2_CH0 | FTM Channel] | PTD10: [FTM2_CH0 | FTM Channel] | PTA0: [FTM2_CH1 | FTM Channel] | PTD1: [FTM2_CH1 | FTM Channel] | PTD11: [FTM2_CH1 | FTM Channel] | PTD12: [FTM2_CH2 | FTM Channel] | PTE4: [FTM2_CH2 | FTM Channel] | PTD5: [FTM2_CH3 | FTM Channel] | PTE5: [FTM2_CH3 | FTM Channel] | PTD13: [FTM2_CH4 | FTM Channel] | PTE10: [FTM2_CH4 | FTM Channel] | PTD14: [FTM2_CH5 | FTM Channel] | PTE11: [FTM2_CH5 | FTM Channel] | PTC12: [FTM2_CH6 | FTM Channel] | PTE15: [FTM2_CH6 | FTM Channel] | PTC13: [FTM2_CH7 | FTM Channel] | PTE16: [FTM2_CH7 | FTM Channel] | PTA2: [FTM3_CH0 | FTM Channel] | PTB8: [FTM3_CH0 | FTM Channel] | PTA3: [FTM3_CH1 | FTM Channel] | PTB9: [FTM3_CH1 | FTM Channel] | PTB10: [FTM3_CH2 | FTM Channel] | PTC6: [FTM3_CH2 | FTM Channel] | PTB11: [FTM3_CH3 | FTM Channel] | PTC7: [FTM3_CH3 | FTM Channel] | PTC10: [FTM3_CH4 | FTM Channel] | PTD2: [FTM3_CH4 | FTM Channel] | PTC11: [FTM3_CH5 | FTM Channel] | PTD3: [FTM3_CH5 | FTM Channel] | PTC12: [FTM3_CH6 | FTM Channel] | PTE2: [FTM3_CH6 | FTM Channel] | PTC13: [FTM3_CH7 | FTM Channel] | PTE6: [FTM3_CH7 | FTM Channel] | PTE20: [FTM4_CH0 | FTM Channel] | PTE21: [FTM4_CH1 | FTM Channel] | PTC11: [FTM4_CH2 | FTM Channel] | PTE22: [FTM4_CH2 | FTM Channel] | PTE23: [FTM4_CH3 | FTM Channel] | PTC27: [FTM4_CH4 | FTM Channel] | PTE24: [FTM4_CH4 | FTM Channel] | PTB1: [FTM4_CH5 | FTM Channel] | PTE13: [FTM4_CH5 | FTM Channel] | PTE25: [FTM4_CH5 | FTM Channel] | PTB0: [FTM4_CH6 | FTM Channel] | PTC28: [FTM4_CH7 | FTM Channel] | PTA25: [FTM5_CH0 | FTM Channel] | PTC9: [FTM5_CH0 | FTM Channel] | PTA26: [FTM5_CH1 | FTM Channel] | PTC8: [FTM5_CH1 | FTM Channel] | PTA27: [FTM5_CH2 | FTM Channel] | PTC29: [FTM5_CH2 | FTM Channel] | PTA7: [FTM5_CH3 | FTM Channel] | PTA28: [FTM5_CH3 | FTM Channel] | PTA29: [FTM5_CH4 | FTM Channel] | PTC30: [FTM5_CH4 | FTM Channel] | PTA6: [FTM5_CH5 | FTM Channel] | PTA30: [FTM5_CH5 | FTM Channel] | PTA31: [FTM5_CH6 | FTM Channel] | PTC31: [FTM5_CH6 | FTM Channel] | PTB18: [FTM5_CH7 | FTM Channel] | PTD18: [FTM5_CH7 | FTM Channel] | PTD15: [FTM0_CH0 | FTM Channel] | PTB13: [FTM0_CH1 | FTM Channel] | PTC1: [FTM0_CH1 | FTM Channel] | PTD16: [FTM0_CH1 | FTM Channel] | PTC2: [FTM0_CH2 | FTM Channel] | PTD0: [FTM0_CH2 | FTM Channel] | PTC3: [FTM0_CH3 | FTM Channel] | PTD1: [FTM0_CH3 | FTM Channel] | PTB4: [FTM0_CH4 | FTM Channel] | PTB5: [FTM0_CH5 | FTM Channel] | PTE8: [FTM0_CH6 | FTM Channel] | PTE9: [FTM0_CH7 | FTM Channel] | PTB2: [FTM1_CH0 | FTM Channel] | PTC4: [FTM1_CH0 | FTM Channel] | PTA1: [FTM1_CH1 | FTM Channel] | PTB3: [FTM1_CH1 | FTM Channel] | PTC14: [FTM1_CH2 | FTM Channel] | PTC15: [FTM1_CH3 | FTM Channel] | PTA10: [FTM1_CH4 | FTM Channel] | PTA11: [FTM1_CH5 | FTM Channel] | PTA12: [FTM1_CH6 | FTM Channel] | PTA13: [FTM1_CH7 | FTM Channel] | PTC1: [FTM1_CH7 | FTM Channel] | PTC5: [FTM2_CH0 | FTM Channel] | PTD0: [FTM2_CH0 | FTM Channel] | PTD10: [FTM2_CH0 | FTM Channel] | PTA0: [FTM2_CH1 | FTM Channel] | PTD1: [FTM2_CH1 | FTM Channel] | PTD11: [FTM2_CH1 | FTM Channel] | PTD12: [FTM2_CH2 | FTM Channel] | PTE4: [FTM2_CH2 | FTM Channel] | PTD5: [FTM2_CH3 | FTM Channel] | PTE5: [FTM2_CH3 | FTM Channel] | PTD13: [FTM2_CH4 | FTM Channel] | PTE10: [FTM2_CH4 | FTM Channel] | PTD14: [FTM2_CH5 | FTM Channel] | PTE11: [FTM2_CH5 | FTM Channel] | PTC12: [FTM2_CH6 | FTM Channel] | PTE15: [FTM2_CH6 | FTM Channel] | PTC13: [FTM2_CH7 | FTM Channel] | PTE16: [FTM2_CH7 | FTM Channel] | PTA2: [FTM3_CH0 | FTM Channel] | PTB8: [FTM3_CH0 | FTM Channel] | PTA3: [FTM3_CH1 | FTM Channel] | PTB9: [FTM3_CH1 | FTM Channel] | PTB10: [FTM3_CH2 | FTM Channel] | PTC6: [FTM3_CH2 | FTM Channel] | PTB11: [FTM3_CH3 | FTM Channel] | PTC7: [FTM3_CH3 | FTM Channel] | PTC10: [FTM3_CH4 | FTM Channel] | PTD2: [FTM3_CH4 | FTM Channel] | PTC11: [FTM3_CH5 | FTM Channel] | PTD3: [FTM3_CH5 | FTM Channel] | PTC12: [FTM3_CH6 | FTM Channel] | PTE2: [FTM3_CH6 | FTM Channel] | PTC13: [FTM3_CH7 | FTM Channel] | PTE6: [FTM3_CH7 | FTM Channel] | PTE20: [FTM4_CH0 | FTM Channel] | PTE21: [FTM4_CH1 | FTM Channel] | PTC11: [FTM4_CH2 | FTM Channel] | PTE22: [FTM4_CH2 | FTM Channel] | PTE23: [FTM4_CH3 | FTM Channel] | PTC27: [FTM4_CH4 | FTM Channel] | PTE24: [FTM4_CH4 | FTM Channel] | PTB1: [FTM4_CH5 | FTM Channel] | PTE13: [FTM4_CH5 | FTM Channel] | PTE25: [FTM4_CH5 | FTM Channel] | PTB0: [FTM4_CH6 | FTM Channel] | PTC28: [FTM4_CH7 | FTM Channel] | PTA25: [FTM5_CH0 | FTM Channel] | PTC9: [FTM5_CH0 | FTM Channel] | PTA26: [FTM5_CH1 | FTM Channel] | PTC8: [FTM5_CH1 | FTM Channel] | PTA27: [FTM5_CH2 | FTM Channel] | PTC29: [FTM5_CH2 | FTM Channel] | PTA7: [FTM5_CH3 | FTM Channel] | PTA28: [FTM5_CH3 | FTM Channel] | PTA29: [FTM5_CH4 | FTM Channel] | PTC30: [FTM5_CH4 | FTM Channel] | PTA6: [FTM5_CH5 | FTM Channel] | PTA30: [FTM5_CH5 | FTM Channel] | PTA31: [FTM5_CH6 | FTM Channel] | PTC31: [FTM5_CH6 | FTM Channel] | PTB18: [FTM5_CH7 | FTM Channel] | PTD18: [FTM5_CH7 | FTM Channel] | PTA18: [FTM6_CH0 | FTM Channel] | PTB20: [FTM6_CH0 | FTM Channel] | PTD19: [FTM6_CH0 | FTM Channel] | PTB21: [FTM6_CH1 | FTM Channel] | PTD20: [FTM6_CH1 | FTM Channel] | PTB22: [FTM6_CH2 | FTM Channel] | PTD21: [FTM6_CH2 | FTM Channel] | PTB23: [FTM6_CH3 | FTM Channel] | PTD22: [FTM6_CH3 | FTM Channel] | PTB24: [FTM6_CH4 | FTM Channel] | PTD23: [FTM6_CH4 | FTM Channel] | PTB25: [FTM6_CH5 | FTM Channel] | PTD24: [FTM6_CH5 | FTM Channel] | PTB26: [FTM6_CH6 | FTM Channel] | PTD25: [FTM6_CH6 | FTM Channel] | PTB27: [FTM6_CH7 | FTM Channel] | PTD26: [FTM6_CH7 | FTM Channel] | PTB28: [FTM7_CH0 | FTM Channel] | PTD27: [FTM7_CH0 | FTM Channel] | PTB29: [FTM7_CH1 | FTM Channel] | PTD28: [FTM7_CH1 | FTM Channel] | PTB30: [FTM7_CH2 | FTM Channel] | PTD29: [FTM7_CH2 | FTM Channel] | PTB31: [FTM7_CH3 | FTM Channel] | PTD30: [FTM7_CH3 | FTM Channel] | PTC18: [FTM7_CH4 | FTM Channel] | PTD31: [FTM7_CH4 | FTM Channel] | PTC19: [FTM7_CH5 | FTM Channel] | PTE17: [FTM7_CH5 | FTM Channel] | PTC20: [FTM7_CH6 | FTM Channel] | PTE18: [FTM7_CH6 | FTM Channel] | PTC21: [FTM7_CH7 | FTM Channel] | PTE19: [FTM7_CH7 | FTM Channel]
      mask TypeOptions pinPolCh2: Active Low | Active High
      mask TypeOptions pinPolCh3: Active Low | Active High
      mask TypeOptions outputComplem2: Main duplicated | Main inverted
      mask TypeOptions outputLevel2: Low | High
      mask TypeOptions outputLevel3: Low | High
      mask TypeOptions pinFtmCh4: PTD15: [FTM0_CH0 | FTM Channel] | PTB13: [FTM0_CH1 | FTM Channel] | PTC1: [FTM0_CH1 | FTM Channel] | PTD16: [FTM0_CH1 | FTM Channel] | PTC2: [FTM0_CH2 | FTM Channel] | PTD0: [FTM0_CH2 | FTM Channel] | PTC3: [FTM0_CH3 | FTM Channel] | PTD1: [FTM0_CH3 | FTM Channel] | PTB4: [FTM0_CH4 | FTM Channel] | PTB5: [FTM0_CH5 | FTM Channel] | PTE8: [FTM0_CH6 | FTM Channel] | PTE9: [FTM0_CH7 | FTM Channel] | PTB2: [FTM1_CH0 | FTM Channel] | PTC4: [FTM1_CH0 | FTM Channel] | PTA1: [FTM1_CH1 | FTM Channel] | PTB3: [FTM1_CH1 | FTM Channel] | PTC14: [FTM1_CH2 | FTM Channel] | PTC15: [FTM1_CH3 | FTM Channel] | PTA10: [FTM1_CH4 | FTM Channel] | PTA11: [FTM1_CH5 | FTM Channel] | PTA12: [FTM1_CH6 | FTM Channel] | PTA13: [FTM1_CH7 | FTM Channel] | PTC1: [FTM1_CH7 | FTM Channel] | PTD15: [FTM0_CH0 | FTM Channel] | PTB13: [FTM0_CH1 | FTM Channel] | PTC1: [FTM0_CH1 | FTM Channel] | PTD16: [FTM0_CH1 | FTM Channel] | PTC2: [FTM0_CH2 | FTM Channel] | PTD0: [FTM0_CH2 | FTM Channel] | PTC3: [FTM0_CH3 | FTM Channel] | PTD1: [FTM0_CH3 | FTM Channel] | PTB4: [FTM0_CH4 | FTM Channel] | PTB5: [FTM0_CH5 | FTM Channel] | PTE8: [FTM0_CH6 | FTM Channel] | PTE9: [FTM0_CH7 | FTM Channel] | PTB2: [FTM1_CH0 | FTM Channel] | PTC4: [FTM1_CH0 | FTM Channel] | PTA1: [FTM1_CH1 | FTM Channel] | PTB3: [FTM1_CH1 | FTM Channel] | PTC14: [FTM1_CH2 | FTM Channel] | PTC15: [FTM1_CH3 | FTM Channel] | PTA10: [FTM1_CH4 | FTM Channel] | PTA11: [FTM1_CH5 | FTM Channel] | PTA12: [FTM1_CH6 | FTM Channel] | PTA13: [FTM1_CH7 | FTM Channel] | PTC1: [FTM1_CH7 | FTM Channel] | PTD15: [FTM0_CH0 | FTM Channel] | PTB13: [FTM0_CH1 | FTM Channel] | PTC1: [FTM0_CH1 | FTM Channel] | PTD16: [FTM0_CH1 | FTM Channel] | PTC2: [FTM0_CH2 | FTM Channel] | PTD0: [FTM0_CH2 | FTM Channel] | PTC3: [FTM0_CH3 | FTM Channel] | PTD1: [FTM0_CH3 | FTM Channel] | PTB4: [FTM0_CH4 | FTM Channel] | PTB5: [FTM0_CH5 | FTM Channel] | PTE8: [FTM0_CH6 | FTM Channel] | PTE9: [FTM0_CH7 | FTM Channel] | PTB2: [FTM1_CH0 | FTM Channel] | PTC4: [FTM1_CH0 | FTM Channel] | PTA1: [FTM1_CH1 | FTM Channel] | PTB3: [FTM1_CH1 | FTM Channel] | PTC14: [FTM1_CH2 | FTM Channel] | PTC15: [FTM1_CH3 | FTM Channel] | PTA10: [FTM1_CH4 | FTM Channel] | PTA11: [FTM1_CH5 | FTM Channel] | PTA12: [FTM1_CH6 | FTM Channel] | PTA13: [FTM1_CH7 | FTM Channel] | PTC1: [FTM1_CH7 | FTM Channel] | PTC5: [FTM2_CH0 | FTM Channel] | PTD0: [FTM2_CH0 | FTM Channel] | PTD10: [FTM2_CH0 | FTM Channel] | PTA0: [FTM2_CH1 | FTM Channel] | PTD1: [FTM2_CH1 | FTM Channel] | PTD11: [FTM2_CH1 | FTM Channel] | PTD12: [FTM2_CH2 | FTM Channel] | PTE4: [FTM2_CH2 | FTM Channel] | PTD5: [FTM2_CH3 | FTM Channel] | PTE5: [FTM2_CH3 | FTM Channel] | PTD13: [FTM2_CH4 | FTM Channel] | PTE10: [FTM2_CH4 | FTM Channel] | PTD14: [FTM2_CH5 | FTM Channel] | PTE11: [FTM2_CH5 | FTM Channel] | PTC12: [FTM2_CH6 | FTM Channel] | PTE15: [FTM2_CH6 | FTM Channel] | PTC13: [FTM2_CH7 | FTM Channel] | PTE16: [FTM2_CH7 | FTM Channel] | PTA2: [FTM3_CH0 | FTM Channel] | PTB8: [FTM3_CH0 | FTM Channel] | PTA3: [FTM3_CH1 | FTM Channel] | PTB9: [FTM3_CH1 | FTM Channel] | PTB10: [FTM3_CH2 | FTM Channel] | PTC6: [FTM3_CH2 | FTM Channel] | PTB11: [FTM3_CH3 | FTM Channel] | PTC7: [FTM3_CH3 | FTM Channel] | PTC10: [FTM3_CH4 | FTM Channel] | PTD2: [FTM3_CH4 | FTM Channel] | PTC11: [FTM3_CH5 | FTM Channel] | PTD3: [FTM3_CH5 | FTM Channel] | PTC12: [FTM3_CH6 | FTM Channel] | PTE2: [FTM3_CH6 | FTM Channel] | PTC13: [FTM3_CH7 | FTM Channel] | PTE6: [FTM3_CH7 | FTM Channel] | PTD15: [FTM0_CH0 | FTM Channel] | PTB13: [FTM0_CH1 | FTM Channel] | PTC1: [FTM0_CH1 | FTM Channel] | PTD16: [FTM0_CH1 | FTM Channel] | PTC2: [FTM0_CH2 | FTM Channel] | PTD0: [FTM0_CH2 | FTM Channel] | PTC3: [FTM0_CH3 | FTM Channel] | PTD1: [FTM0_CH3 | FTM Channel] | PTB4: [FTM0_CH4 | FTM Channel] | PTB5: [FTM0_CH5 | FTM Channel] | PTE8: [FTM0_CH6 | FTM Channel] | PTE9: [FTM0_CH7 | FTM Channel] | PTB2: [FTM1_CH0 | FTM Channel] | PTC4: [FTM1_CH0 | FTM Channel] | PTA1: [FTM1_CH1 | FTM Channel] | PTB3: [FTM1_CH1 | FTM Channel] | PTC14: [FTM1_CH2 | FTM Channel] | PTC15: [FTM1_CH3 | FTM Channel] | PTA10: [FTM1_CH4 | FTM Channel] | PTA11: [FTM1_CH5 | FTM Channel] | PTA12: [FTM1_CH6 | FTM Channel] | PTA13: [FTM1_CH7 | FTM Channel] | PTC1: [FTM1_CH7 | FTM Channel] | PTC5: [FTM2_CH0 | FTM Channel] | PTD0: [FTM2_CH0 | FTM Channel] | PTD10: [FTM2_CH0 | FTM Channel] | PTA0: [FTM2_CH1 | FTM Channel] | PTD1: [FTM2_CH1 | FTM Channel] | PTD11: [FTM2_CH1 | FTM Channel] | PTD12: [FTM2_CH2 | FTM Channel] | PTE4: [FTM2_CH2 | FTM Channel] | PTD5: [FTM2_CH3 | FTM Channel] | PTE5: [FTM2_CH3 | FTM Channel] | PTD13: [FTM2_CH4 | FTM Channel] | PTE10: [FTM2_CH4 | FTM Channel] | PTD14: [FTM2_CH5 | FTM Channel] | PTE11: [FTM2_CH5 | FTM Channel] | PTC12: [FTM2_CH6 | FTM Channel] | PTE15: [FTM2_CH6 | FTM Channel] | PTC13: [FTM2_CH7 | FTM Channel] | PTE16: [FTM2_CH7 | FTM Channel] | PTA2: [FTM3_CH0 | FTM Channel] | PTB8: [FTM3_CH0 | FTM Channel] | PTA3: [FTM3_CH1 | FTM Channel] | PTB9: [FTM3_CH1 | FTM Channel] | PTB10: [FTM3_CH2 | FTM Channel] | PTC6: [FTM3_CH2 | FTM Channel] | PTB11: [FTM3_CH3 | FTM Channel] | PTC7: [FTM3_CH3 | FTM Channel] | PTC10: [FTM3_CH4 | FTM Channel] | PTD2: [FTM3_CH4 | FTM Channel] | PTC11: [FTM3_CH5 | FTM Channel] | PTD3: [FTM3_CH5 | FTM Channel] | PTC12: [FTM3_CH6 | FTM Channel] | PTE2: [FTM3_CH6 | FTM Channel] | PTC13: [FTM3_CH7 | FTM Channel] | PTE6: [FTM3_CH7 | FTM Channel] | PTD15: [FTM0_CH0 | FTM Channel] | PTB13: [FTM0_CH1 | FTM Channel] | PTC1: [FTM0_CH1 | FTM Channel] | PTD16: [FTM0_CH1 | FTM Channel] | PTC2: [FTM0_CH2 | FTM Channel] | PTD0: [FTM0_CH2 | FTM Channel] | PTC3: [FTM0_CH3 | FTM Channel] | PTD1: [FTM0_CH3 | FTM Channel] | PTB4: [FTM0_CH4 | FTM Channel] | PTB5: [FTM0_CH5 | FTM Channel] | PTE8: [FTM0_CH6 | FTM Channel] | PTE9: [FTM0_CH7 | FTM Channel] | PTB2: [FTM1_CH0 | FTM Channel] | PTC4: [FTM1_CH0 | FTM Channel] | PTA1: [FTM1_CH1 | FTM Channel] | PTB3: [FTM1_CH1 | FTM Channel] | PTC14: [FTM1_CH2 | FTM Channel] | PTC15: [FTM1_CH3 | FTM Channel] | PTA10: [FTM1_CH4 | FTM Channel] | PTA11: [FTM1_CH5 | FTM Channel] | PTA12: [FTM1_CH6 | FTM Channel] | PTA13: [FTM1_CH7 | FTM Channel] | PTC1: [FTM1_CH7 | FTM Channel] | PTC5: [FTM2_CH0 | FTM Channel] | PTD0: [FTM2_CH0 | FTM Channel] | PTD10: [FTM2_CH0 | FTM Channel] | PTA0: [FTM2_CH1 | FTM Channel] | PTD1: [FTM2_CH1 | FTM Channel] | PTD11: [FTM2_CH1 | FTM Channel] | PTD12: [FTM2_CH2 | FTM Channel] | PTE4: [FTM2_CH2 | FTM Channel] | PTD5: [FTM2_CH3 | FTM Channel] | PTE5: [FTM2_CH3 | FTM Channel] | PTD13: [FTM2_CH4 | FTM Channel] | PTE10: [FTM2_CH4 | FTM Channel] | PTD14: [FTM2_CH5 | FTM Channel] | PTE11: [FTM2_CH5 | FTM Channel] | PTC12: [FTM2_CH6 | FTM Channel] | PTE15: [FTM2_CH6 | FTM Channel] | PTC13: [FTM2_CH7 | FTM Channel] | PTE16: [FTM2_CH7 | FTM Channel] | PTA2: [FTM3_CH0 | FTM Channel] | PTB8: [FTM3_CH0 | FTM Channel] | PTA3: [FTM3_CH1 | FTM Channel] | PTB9: [FTM3_CH1 | FTM Channel] | PTB10: [FTM3_CH2 | FTM Channel] | PTC6: [FTM3_CH2 | FTM Channel] | PTB11: [FTM3_CH3 | FTM Channel] | PTC7: [FTM3_CH3 | FTM Channel] | PTC10: [FTM3_CH4 | FTM Channel] | PTD2: [FTM3_CH4 | FTM Channel] | PTC11: [FTM3_CH5 | FTM Channel] | PTD3: [FTM3_CH5 | FTM Channel] | PTC12: [FTM3_CH6 | FTM Channel] | PTE2: [FTM3_CH6 | FTM Channel] | PTC13: [FTM3_CH7 | FTM Channel] | PTE6: [FTM3_CH7 | FTM Channel] | PTE20: [FTM4_CH0 | FTM Channel] | PTE21: [FTM4_CH1 | FTM Channel] | PTC11: [FTM4_CH2 | FTM Channel] | PTE22: [FTM4_CH2 | FTM Channel] | PTE23: [FTM4_CH3 | FTM Channel] | PTC27: [FTM4_CH4 | FTM Channel] | PTE24: [FTM4_CH4 | FTM Channel] | PTB1: [FTM4_CH5 | FTM Channel] | PTE13: [FTM4_CH5 | FTM Channel] | PTE25: [FTM4_CH5 | FTM Channel] | PTB0: [FTM4_CH6 | FTM Channel] | PTC28: [FTM4_CH7 | FTM Channel] | PTA25: [FTM5_CH0 | FTM Channel] | PTC9: [FTM5_CH0 | FTM Channel] | PTA26: [FTM5_CH1 | FTM Channel] | PTC8: [FTM5_CH1 | FTM Channel] | PTA27: [FTM5_CH2 | FTM Channel] | PTC29: [FTM5_CH2 | FTM Channel] | PTA7: [FTM5_CH3 | FTM Channel] | PTA28: [FTM5_CH3 | FTM Channel] | PTA29: [FTM5_CH4 | FTM Channel] | PTC30: [FTM5_CH4 | FTM Channel] | PTA6: [FTM5_CH5 | FTM Channel] | PTA30: [FTM5_CH5 | FTM Channel] | PTA31: [FTM5_CH6 | FTM Channel] | PTC31: [FTM5_CH6 | FTM Channel] | PTB18: [FTM5_CH7 | FTM Channel] | PTD18: [FTM5_CH7 | FTM Channel] | PTD15: [FTM0_CH0 | FTM Channel] | PTB13: [FTM0_CH1 | FTM Channel] | PTC1: [FTM0_CH1 | FTM Channel] | PTD16: [FTM0_CH1 | FTM Channel] | PTC2: [FTM0_CH2 | FTM Channel] | PTD0: [FTM0_CH2 | FTM Channel] | PTC3: [FTM0_CH3 | FTM Channel] | PTD1: [FTM0_CH3 | FTM Channel] | PTB4: [FTM0_CH4 | FTM Channel] | PTB5: [FTM0_CH5 | FTM Channel] | PTE8: [FTM0_CH6 | FTM Channel] | PTE9: [FTM0_CH7 | FTM Channel] | PTB2: [FTM1_CH0 | FTM Channel] | PTC4: [FTM1_CH0 | FTM Channel] | PTA1: [FTM1_CH1 | FTM Channel] | PTB3: [FTM1_CH1 | FTM Channel] | PTC14: [FTM1_CH2 | FTM Channel] | PTC15: [FTM1_CH3 | FTM Channel] | PTA10: [FTM1_CH4 | FTM Channel] | PTA11: [FTM1_CH5 | FTM Channel] | PTA12: [FTM1_CH6 | FTM Channel] | PTA13: [FTM1_CH7 | FTM Channel] | PTC1: [FTM1_CH7 | FTM Channel] | PTC5: [FTM2_CH0 | FTM Channel] | PTD0: [FTM2_CH0 | FTM Channel] | PTD10: [FTM2_CH0 | FTM Channel] | PTA0: [FTM2_CH1 | FTM Channel] | PTD1: [FTM2_CH1 | FTM Channel] | PTD11: [FTM2_CH1 | FTM Channel] | PTD12: [FTM2_CH2 | FTM Channel] | PTE4: [FTM2_CH2 | FTM Channel] | PTD5: [FTM2_CH3 | FTM Channel] | PTE5: [FTM2_CH3 | FTM Channel] | PTD13: [FTM2_CH4 | FTM Channel] | PTE10: [FTM2_CH4 | FTM Channel] | PTD14: [FTM2_CH5 | FTM Channel] | PTE11: [FTM2_CH5 | FTM Channel] | PTC12: [FTM2_CH6 | FTM Channel] | PTE15: [FTM2_CH6 | FTM Channel] | PTC13: [FTM2_CH7 | FTM Channel] | PTE16: [FTM2_CH7 | FTM Channel] | PTA2: [FTM3_CH0 | FTM Channel] | PTB8: [FTM3_CH0 | FTM Channel] | PTA3: [FTM3_CH1 | FTM Channel] | PTB9: [FTM3_CH1 | FTM Channel] | PTB10: [FTM3_CH2 | FTM Channel] | PTC6: [FTM3_CH2 | FTM Channel] | PTB11: [FTM3_CH3 | FTM Channel] | PTC7: [FTM3_CH3 | FTM Channel] | PTC10: [FTM3_CH4 | FTM Channel] | PTD2: [FTM3_CH4 | FTM Channel] | PTC11: [FTM3_CH5 | FTM Channel] | PTD3: [FTM3_CH5 | FTM Channel] | PTC12: [FTM3_CH6 | FTM Channel] | PTE2: [FTM3_CH6 | FTM Channel] | PTC13: [FTM3_CH7 | FTM Channel] | PTE6: [FTM3_CH7 | FTM Channel] | PTE20: [FTM4_CH0 | FTM Channel] | PTE21: [FTM4_CH1 | FTM Channel] | PTC11: [FTM4_CH2 | FTM Channel] | PTE22: [FTM4_CH2 | FTM Channel] | PTE23: [FTM4_CH3 | FTM Channel] | PTC27: [FTM4_CH4 | FTM Channel] | PTE24: [FTM4_CH4 | FTM Channel] | PTB1: [FTM4_CH5 | FTM Channel] | PTE13: [FTM4_CH5 | FTM Channel] | PTE25: [FTM4_CH5 | FTM Channel] | PTB0: [FTM4_CH6 | FTM Channel] | PTC28: [FTM4_CH7 | FTM Channel] | PTA25: [FTM5_CH0 | FTM Channel] | PTC9: [FTM5_CH0 | FTM Channel] | PTA26: [FTM5_CH1 | FTM Channel] | PTC8: [FTM5_CH1 | FTM Channel] | PTA27: [FTM5_CH2 | FTM Channel] | PTC29: [FTM5_CH2 | FTM Channel] | PTA7: [FTM5_CH3 | FTM Channel] | PTA28: [FTM5_CH3 | FTM Channel] | PTA29: [FTM5_CH4 | FTM Channel] | PTC30: [FTM5_CH4 | FTM Channel] | PTA6: [FTM5_CH5 | FTM Channel] | PTA30: [FTM5_CH5 | FTM Channel] | PTA31: [FTM5_CH6 | FTM Channel] | PTC31: [FTM5_CH6 | FTM Channel] | PTB18: [FTM5_CH7 | FTM Channel] | PTD18: [FTM5_CH7 | FTM Channel] | PTA18: [FTM6_CH0 | FTM Channel] | PTB20: [FTM6_CH0 | FTM Channel] | PTD19: [FTM6_CH0 | FTM Channel] | PTB21: [FTM6_CH1 | FTM Channel] | PTD20: [FTM6_CH1 | FTM Channel] | PTB22: [FTM6_CH2 | FTM Channel] | PTD21: [FTM6_CH2 | FTM Channel] | PTB23: [FTM6_CH3 | FTM Channel] | PTD22: [FTM6_CH3 | FTM Channel] | PTB24: [FTM6_CH4 | FTM Channel] | PTD23: [FTM6_CH4 | FTM Channel] | PTB25: [FTM6_CH5 | FTM Channel] | PTD24: [FTM6_CH5 | FTM Channel] | PTB26: [FTM6_CH6 | FTM Channel] | PTD25: [FTM6_CH6 | FTM Channel] | PTB27: [FTM6_CH7 | FTM Channel] | PTD26: [FTM6_CH7 | FTM Channel] | PTB28: [FTM7_CH0 | FTM Channel] | PTD27: [FTM7_CH0 | FTM Channel] | PTB29: [FTM7_CH1 | FTM Channel] | PTD28: [FTM7_CH1 | FTM Channel] | PTB30: [FTM7_CH2 | FTM Channel] | PTD29: [FTM7_CH2 | FTM Channel] | PTB31: [FTM7_CH3 | FTM Channel] | PTD30: [FTM7_CH3 | FTM Channel] | PTC18: [FTM7_CH4 | FTM Channel] | PTD31: [FTM7_CH4 | FTM Channel] | PTC19: [FTM7_CH5 | FTM Channel] | PTE17: [FTM7_CH5 | FTM Channel] | PTC20: [FTM7_CH6 | FTM Channel] | PTE18: [FTM7_CH6 | FTM Channel] | PTC21: [FTM7_CH7 | FTM Channel] | PTE19: [FTM7_CH7 | FTM Channel]
